simulink model "ATRIAS_vnmc"  (R2015a)
settings: Solver=ode45  StartTime=0.0  StopTime=60  FixedStep=1e-3  MinStep=1e-6  RelTol=1e-3  AbsTol=1e-4
values from neighbouring files (symbols this model uses):
  initial_boom_yaw = initial_boom_yaw + delta_yaw0    [run_model.m]
  max_floor_diff = cost_fun_opts.max_floor_diff    [opt_cmaes.m]    (also in run_model.m; set_all_params_simple.m = 0)
  noise_on_off = cost_fun_opts.noise_on_off    [opt_cmaes.m]    (also in run_model.m; set_all_params_simple.m = 0)
  noise_seed = cost_fun_opts.noise_seed    [opt_cmaes.m]    (also in run_model.m; set_all_params_simple.m = 1)
  noise_variance = cost_fun_opts.noise_variance    [opt_cmaes.m]    (also in run_model.m; set_all_params_simple.m = 0.000174532925199)
  SEA_swing_ctrl_on_off = cost_fun_opts.SEA_swing_ctrl_on_off    [opt_cmaes.m]    (also in run_model.m; set_all_params_simple.m = 0)
  sim_t = simout.twalk    [run_model.m]
  steady_dist = cost_fun_opts.steady_dist    [opt_cmaes.m]    (also in run_model.m; set_all_params_simple.m = 10)
  ts_anim = 0.0333    [run_model.m]
undefined symbols (not defined in the file or in its folder): A1_notch_f1, A2_notch_f1, A_lpf_dtau, A_lpf_velocity, B1_lpf_dtau, B1_lpf_velocity, B1_notch_f1, B2_lpf_dtau, B2_lpf_velocity, B2_notch_f1, b_hmotor, b_leg_spring, b_rotor, base_color_d, boom_color_d, boom_mount_to_center_diagonal, breakaway_friction, c, c_jointstop, com_height_offset, contactThr, coulomb_friction, CtrlPar_theta0, D12_S, D12_T, d_com, ddx_max, ddy_max, delta_phi_max, delta_phi_max_buffer, delta_phi_max_dropoff, delta_phi_min, des_forward_velocity, DS_width, dtau_des_max, dtheta0_vmc, dx0_vmc, dy_max, eref, fblink_color_d, fcut_acceleration, floor_color_d, floor_tile_width, floor_zero_height, FmaxBFSH, FmaxGLU, FmaxHAM, FmaxHFL, FmaxRF, FmaxVAS, FPCtrlPar, friction_linear_zone, g, gain_nodes_sea_torque, gamma_stance_thr, gamma_swing_thr, hip_height, HIP_MTR_MAX_CONT_TORQUE, HIP_MTR_MAX_TORQUE, hshaft_color_d ... (+236)
libraries: sm_lib x280, nesl_utility x174, simulink x114, simulink_extras x58, fl_lib x16, mblibv1 x2, dspswit3 x2
(part 21 of 23)

== matlab function ATRIAS_vnmc/control/Virtual Model Control/KKT_DS ==
  settings: updateMethod=DISCRETE  sampleTime=sample_time
  data: motor_trq output size=[4,1]; leg_force_hip_torque output size=[4,1]; grf output size=[4,1]; ddx_des input size=1; ddy_des input size=1; ddtheta_des input size=1; R_leg_length input size=1; L_leg_length input size=1; min_Fy input; R_gamma input size=1; L_gamma input size=1; R_splay input size=1; L_splay input size=1; theta input size=1; lambda1 input size=1; lambda2 input size=1; lambda3 input size=1; lambda4 input; mu_s input; sea_trqs input; cost_tie_break output size=1; err output size=[1,3]; grf_prev input
function [motor_trq,leg_force_hip_torque,grf,cost_tie_break,err]  = ...
         vmc(ddx_des,ddy_des,ddtheta_des,R_leg_length,L_leg_length,...
                min_Fy,R_gamma,L_gamma,R_splay,L_splay,theta,...
                lambda1,lambda2,lambda3,lambda4,mu_s,sea_trqs,grf_prev)

L1 = R_leg_length;
L2 = L_leg_length;
gamma1 = R_gamma;
gamma2 = L_gamma;
m = 64;
I = 4;
d = 0.1;
l_seg = 0.5;
g = 9.81;
% mu_s = 0.25;

% leg_force_hip_torque = J1*grf;
% motor_trq = J2*leg_force_hip_torque;
% motor_trq = J2*J1*grf;
% grf = J1_inv * J2_inv * motor_trq

J1 = [-sin(gamma1) -cos(gamma1) 0 0;
      -L1*cos(gamma1) L1*sin(gamma1) 0 0;
      0 0 -sin(gamma2) -cos(gamma2);
      0 0 -L2*cos(gamma2) L2*sin(gamma2)];
  
J2 = [-l_seg*sin(R_splay/2) 0.5 0 0;
       l_seg*sin(R_splay/2) 0.5 0 0;
       0 0 -l_seg*sin(L_splay/2) 0.5;
       0 0 l_seg*sin(R_splay/2) 0.5];
   
grf_meas = J1\J2\sea_trqs;


f1 = real([(I*ddtheta_des - L2*ddx_des*m*cos(gamma2) + L1*ddy_des*m*sin(gamma1) + L1*g*m*sin(gamma1) + d*ddx_des*m*cos(theta) - d*ddy_des*m*sin(theta) - d*g*m*sin(theta))/(L1*cos(gamma1) - L2*cos(gamma2));                                                                                                                                                                                                                                                                                                                                                                                                                                                                                                                                                                                                                                                                                                                                                                                                                                                                                                                                                                                                                                                                                                                                                                                                                                                                                                                                                                                                                                                                                                                                                                                                                                                                                                                                                                                                                                                                                                                                                                                                                                                                                                                                                                                                                                                                                                                                                                                                                                                                                                                                                                                                                                                                                                                                                                                                                                                                                                                                                                                                                                                                                                                                                                                                                                                                                                                                                                                                                                                                                                                                                                                                                                                                                                                                                                                                                                                                                                                                                                                                                                                                                                                                                                                                                                                                                                                                                                                                                                                                                                                                                                                                                                                                                                                                                                                                                                                                                                                                                                                                                                                                                                                                                                                                                                                                                                                                                                                                                                        
    (I*ddtheta_des - L2*ddx_des*m*cos(gamma2) + L2*ddy_des*m*sin(gamma2) + L2*g*m*sin(gamma2) + d*ddx_des*m*cos(theta) - d*ddy_des*m*sin(theta) - d*g*m*sin(theta))/(L1*cos(gamma1) - L2*cos(gamma2));
    (I^2*ddx_des*lambda1*lambda2*m + L1^2*ddx_des*lambda1*lambda3*m^3*sin(gamma1)^2 + d^2*ddx_des*lambda1*lambda3*m^3*sin(theta)^2 + L1^2*ddy_des*lambda2*lambda3*m^3*cos(gamma1)*sin(gamma1) + L1^2*g*lambda2*lambda3*m^3*cos(gamma1)*sin(gamma1) + I*L1*ddtheta_des*lambda2*lambda3*m^2*cos(gamma1) + d^2*ddy_des*lambda2*lambda3*m^3*cos(theta)*sin(theta) - I*d*ddtheta_des*lambda2*lambda3*m^2*cos(theta) + d^2*g*lambda2*lambda3*m^3*cos(theta)*sin(theta) - L1*d*ddy_des*lambda2*lambda3*m^3*cos(gamma1)*sin(theta) - L1*d*ddy_des*lambda2*lambda3*m^3*cos(theta)*sin(gamma1) - L1*d*g*lambda2*lambda3*m^3*cos(gamma1)*sin(theta) - L1*d*g*lambda2*lambda3*m^3*cos(theta)*sin(gamma1) - 2*L1*d*ddx_des*lambda1*lambda3*m^3*sin(gamma1)*sin(theta))/(I^2*lambda1*lambda2 + d^2*lambda1*lambda3*m^2*sin(theta)^2 + L1^2*lambda2*lambda3*m^2*cos(gamma1)^2 + L1^2*lambda1*lambda3*m^2*sin(gamma1)^2 + d^2*lambda2*lambda3*m^2*cos(theta)^2 - 2*L1*d*lambda2*lambda3*m^2*cos(gamma1)*cos(theta) - 2*L1*d*lambda1*lambda3*m^2*sin(gamma1)*sin(theta));
    0;
    0;
    0;
    0;
    0;
    (I*ddtheta_des - L2*ddx_des*m*cos(gamma2) + L1*ddy_des*m*sin(gamma1) + L1*g*m*sin(gamma1) + d*ddx_des*m*cos(theta) - d*ddy_des*m*sin(theta) - d*g*m*sin(theta))/(L1*cos(gamma1) - L2*cos(gamma2));
    0;
    (I^2*ddx_des*lambda1*lambda2*m + L1^2*ddx_des*lambda1*lambda3*m^3*sin(gamma1)^2 + d^2*ddx_des*lambda1*lambda3*m^3*sin(theta)^2 + L1^2*ddy_des*lambda2*lambda3*m^3*cos(gamma1)*sin(gamma1) + L1^2*g*lambda2*lambda3*m^3*cos(gamma1)*sin(gamma1) + I*L1*ddtheta_des*lambda2*lambda3*m^2*cos(gamma1) + d^2*ddy_des*lambda2*lambda3*m^3*cos(theta)*sin(theta) - I*d*ddtheta_des*lambda2*lambda3*m^2*cos(theta) + d^2*g*lambda2*lambda3*m^3*cos(theta)*sin(theta) - L1*d*ddy_des*lambda2*lambda3*m^3*cos(gamma1)*sin(theta) - L1*d*ddy_des*lambda2*lambda3*m^3*cos(theta)*sin(gamma1) - L1*d*g*lambda2*lambda3*m^3*cos(gamma1)*sin(theta) - L1*d*g*lambda2*lambda3*m^3*cos(theta)*sin(gamma1) - 2*L1*d*ddx_des*lambda1*lambda3*m^3*sin(gamma1)*sin(theta))/(I^2*lambda1*lambda2 + d^2*lambda1*lambda3*m^2*sin(theta)^2 + L1^2*lambda2*lambda3*m^2*cos(gamma1)^2 + L1^2*lambda1*lambda3*m^2*sin(gamma1)^2 + d^2*lambda2*lambda3*m^2*cos(theta)^2 - 2*L1*d*lambda2*lambda3*m^2*cos(gamma1)*cos(theta) - 2*L1*d*lambda1*lambda3*m^2*sin(gamma1)*sin(theta));
    0;
    0;
    0;
    0;
    0;
    (I*ddtheta_des*mu_s + L1*ddx_des*m*sin(gamma1) - L2*ddx_des*m*sin(gamma2) - L2*ddx_des*m*mu_s*cos(gamma2) + L1*ddy_des*m*mu_s*sin(gamma1) + L1*g*m*mu_s*sin(gamma1) + d*ddx_des*m*mu_s*cos(theta) - d*ddy_des*m*mu_s*sin(theta) - d*g*m*mu_s*sin(theta))/(L1*sin(gamma1) - L2*sin(gamma2) + L1*mu_s*cos(gamma1) - L2*mu_s*cos(gamma2));
    -(I*ddtheta_des*mu_s - L1*ddx_des*m*sin(gamma1) + L2*ddx_des*m*sin(gamma2) - L2*ddx_des*m*mu_s*cos(gamma2) + L1*ddy_des*m*mu_s*sin(gamma1) + L1*g*m*mu_s*sin(gamma1) + d*ddx_des*m*mu_s*cos(theta) - d*ddy_des*m*mu_s*sin(theta) - d*g*m*mu_s*sin(theta))/(L1*sin(gamma1) - L2*sin(gamma2) - L1*mu_s*cos(gamma1) + L2*mu_s*cos(gamma2));
    (mu_s*(I*ddtheta_des - L2*ddx_des*m*cos(gamma2) + L2*ddy_des*m*sin(gamma2) + L2*g*m*sin(gamma2) + d*ddx_des*m*cos(theta) - d*ddy_des*m*sin(theta) - d*g*m*sin(theta)))/(L1*sin(gamma1) - L2*sin(gamma2) + L1*mu_s*cos(gamma1) - L2*mu_s*cos(gamma2));
    -(mu_s*(I*ddtheta_des - L2*ddx_des*m*cos(gamma2) + L2*ddy_des*m*sin(gamma2) + L2*g*m*sin(gamma2) + d*ddx_des*m*cos(theta) - d*ddy_des*m*sin(theta) - d*g*m*sin(theta)))/(L1*sin(gamma1) - L2*sin(gamma2) - L1*mu_s*cos(gamma1) + L2*mu_s*cos(gamma2));
    (m*mu_s*(I^2*ddy_des*lambda1*lambda2 + I^2*g*lambda1*lambda2 + L2^2*ddy_des*lambda2*lambda3*m^2*cos(gamma2)^2 + L2^2*g*lambda2*lambda3*m^2*cos(gamma2)^2 + d^2*ddy_des*lambda2*lambda3*m^2*cos(theta)^2 + d^2*g*lambda2*lambda3*m^2*cos(theta)^2 - I*L1*ddtheta_des*lambda1*lambda3*m*sin(gamma1) + I*d*ddtheta_des*lambda1*lambda3*m*sin(theta) + L2^2*ddx_des*lambda1*lambda3*m^2*mu_s*cos(gamma2)^2 + d^2*ddx_des*lambda1*lambda3*m^2*cos(theta)*sin(theta) + L1*L2*ddx_des*lambda1*lambda3*m^2*cos(gamma2)*sin(gamma1) - 2*L2*d*ddy_des*lambda2*lambda3*m^2*cos(gamma2)*cos(theta) - 2*L2*d*g*lambda2*lambda3*m^2*cos(gamma2)*cos(theta) - L1*d*ddx_des*lambda1*lambda3*m^2*cos(theta)*sin(gamma1) - L2*d*ddx_des*lambda1*lambda3*m^2*cos(gamma2)*sin(theta) + I*L1*ddtheta_des*lambda1*lambda3*m*mu_s*cos(gamma1) - I*L2*ddtheta_des*lambda1*lambda3*m*mu_s*cos(gamma2) - L1*L2*ddx_des*lambda1*lambda3*m^2*mu_s*cos(gamma1)*cos(gamma2) + L1*d*ddx_des*lambda1*lambda3*m^2*mu_s*cos(gamma1)*cos(theta) - L2*d*ddx_des*lambda1*lambda3*m^2*mu_s*cos(gamma2)*cos(theta)))/(I^2*lambda1*lambda2 + d^2*lambda1*lambda3*m^2*sin(theta)^2 + L2^2*lambda2*lambda3*m^2*cos(gamma2)^2 + L1^2*lambda1*lambda3*m^2*sin(gamma1)^2 + d^2*lambda2*lambda3*m^2*cos(theta)^2 + L1^2*lambda1*lambda3*m^2*mu_s^2*cos(gamma1)^2 + L2^2*lambda1*lambda3*m^2*mu_s^2*cos(gamma2)^2 - 2*L2*d*lambda2*lambda3*m^2*cos(gamma2)*cos(theta) - 2*L1*d*lambda1*lambda3*m^2*sin(gamma1)*sin(theta) - 2*L1^2*lambda1*lambda3*m^2*mu_s*cos(gamma1)*sin(gamma1) + 2*L1*L2*lambda1*lambda3*m^2*mu_s*cos(gamma2)*sin(gamma1) + 2*L1*d*lambda1*lambda3*m^2*mu_s*cos(gamma1)*sin(theta) - 2*L2*d*lambda1*lambda3*m^2*mu_s*cos(gamma2)*sin(theta) - 2*L1*L2*lambda1*lambda3*m^2*mu_s^2*cos(gamma1)*cos(gamma2));
    0;
    (I*m*mu_s*(I*ddy_des*lambda2 + I*g*lambda2 + I*ddx_des*lambda1*mu_s - L1*ddtheta_des*lambda3*m*sin(gamma1) + d*ddtheta_des*lambda3*m*sin(theta) + L1*ddtheta_des*lambda3*m*mu_s*cos(gamma1) - d*ddtheta_des*lambda3*m*mu_s*cos(theta)))/(I^2*lambda2 + I^2*lambda1*mu_s^2 + L1^2*lambda3*m^2*sin(gamma1)^2 + d^2*lambda3*m^2*sin(theta)^2 + L1^2*lambda3*m^2*mu_s^2*cos(gamma1)^2 + d^2*lambda3*m^2*mu_s^2*cos(theta)^2 - 2*L1*d*lambda3*m^2*sin(gamma1)*sin(theta) - 2*L1^2*lambda3*m^2*mu_s*cos(gamma1)*sin(gamma1) - 2*d^2*lambda3*m^2*mu_s*cos(theta)*sin(theta) + 2*L1*d*lambda3*m^2*mu_s*cos(gamma1)*sin(theta) + 2*L1*d*lambda3*m^2*mu_s*cos(theta)*sin(gamma1) - 2*L1*d*lambda3*m^2*mu_s^2*cos(gamma1)*cos(theta));
    -(I*m*mu_s*(I*ddy_des*lambda2 + I*g*lambda2 - I*ddx_des*lambda1*mu_s - L1*ddtheta_des*lambda3*m*sin(gamma1) + d*ddtheta_des*lambda3*m*sin(theta) - L1*ddtheta_des*lambda3*m*mu_s*cos(gamma1) + d*ddtheta_des*lambda3*m*mu_s*cos(theta)))/(I^2*lambda2 + I^2*lambda1*mu_s^2 + L1^2*lambda3*m^2*sin(gamma1)^2 + d^2*lambda3*m^2*sin(theta)^2 + L1^2*lambda3*m^2*mu_s^2*cos(gamma1)^2 + d^2*lambda3*m^2*mu_s^2*cos(theta)^2 - 2*L1*d*lambda3*m^2*sin(gamma1)*sin(theta) + 2*L1^2*lambda3*m^2*mu_s*cos(gamma1)*sin(gamma1) + 2*d^2*lambda3*m^2*mu_s*cos(theta)*sin(theta) - 2*L1*d*lambda3*m^2*mu_s*cos(gamma1)*sin(theta) - 2*L1*d*lambda3*m^2*mu_s*cos(theta)*sin(gamma1) - 2*L1*d*lambda3*m^2*mu_s^2*cos(gamma1)*cos(theta));
    0;
    0;
    (I*(I*ddx_des*lambda1*m + L1*ddtheta_des*lambda3*m^2*cos(gamma1) - d*ddtheta_des*lambda3*m^2*cos(theta)))/(I^2*lambda1 + L1^2*lambda3*m^2*cos(gamma1)^2 + d^2*lambda3*m^2*cos(theta)^2 - 2*L1*d*lambda3*m^2*cos(gamma1)*cos(theta));
    (mu_s*(I*ddtheta_des*lambda2 + I*ddtheta_des*lambda1*mu_s^2 + L2*ddy_des*lambda2*m*sin(gamma2) + L2*g*lambda2*m*sin(gamma2) - d*ddy_des*lambda2*m*sin(theta) - d*g*lambda2*m*sin(theta) + L2*ddy_des*lambda2*m*mu_s*cos(gamma2) + L2*g*lambda2*m*mu_s*cos(gamma2) - L2*ddx_des*lambda1*m*mu_s*sin(gamma2) - d*ddy_des*lambda2*m*mu_s*cos(theta) - d*g*lambda2*m*mu_s*cos(theta) + d*ddx_des*lambda1*m*mu_s*sin(theta) - L2*ddx_des*lambda1*m*mu_s^2*cos(gamma2) + d*ddx_des*lambda1*m*mu_s^2*cos(theta)))/((lambda1*mu_s^2 + lambda2)*(L1*sin(gamma1) - L2*sin(gamma2) + L1*mu_s*cos(gamma1) - L2*mu_s*cos(gamma2)));
    -(mu_s*(I*ddtheta_des*lambda2 + I*ddtheta_des*lambda1*mu_s^2 + L2*ddy_des*lambda2*m*sin(gamma2) + L2*g*lambda2*m*sin(gamma2) - d*ddy_des*lambda2*m*sin(theta) - d*g*lambda2*m*sin(theta) - L2*ddy_des*lambda2*m*mu_s*cos(gamma2) - L2*g*lambda2*m*mu_s*cos(gamma2) + L2*ddx_des*lambda1*m*mu_s*sin(gamma2) + d*ddy_des*lambda2*m*mu_s*cos(theta) + d*g*lambda2*m*mu_s*cos(theta) - d*ddx_des*lambda1*m*mu_s*sin(theta) - L2*ddx_des*lambda1*m*mu_s^2*cos(gamma2) + d*ddx_des*lambda1*m*mu_s^2*cos(theta)))/((lambda1*mu_s^2 + lambda2)*(L1*sin(gamma1) - L2*sin(gamma2) - L1*mu_s*cos(gamma1) + L2*mu_s*cos(gamma2)));
    -(m*mu_s*(I^2*ddy_des*lambda1*lambda2 + I^2*g*lambda1*lambda2 + L2^2*ddy_des*lambda2*lambda3*m^2*cos(gamma2)^2 + L2^2*g*lambda2*lambda3*m^2*cos(gamma2)^2 + d^2*ddy_des*lambda2*lambda3*m^2*cos(theta)^2 + d^2*g*lambda2*lambda3*m^2*cos(theta)^2 - I*L1*ddtheta_des*lambda1*lambda3*m*sin(gamma1) + I*d*ddtheta_des*lambda1*lambda3*m*sin(theta) - L2^2*ddx_des*lambda1*lambda3*m^2*mu_s*cos(gamma2)^2 + d^2*ddx_des*lambda1*lambda3*m^2*cos(theta)*sin(theta) + L1*L2*ddx_des*lambda1*lambda3*m^2*cos(gamma2)*sin(gamma1) - 2*L2*d*ddy_des*lambda2*lambda3*m^2*cos(gamma2)*cos(theta) - 2*L2*d*g*lambda2*lambda3*m^2*cos(gamma2)*cos(theta) - L1*d*ddx_des*lambda1*lambda3*m^2*cos(theta)*sin(gamma1) - L2*d*ddx_des*lambda1*lambda3*m^2*cos(gamma2)*sin(theta) - I*L1*ddtheta_des*lambda1*lambda3*m*mu_s*cos(gamma1) + I*L2*ddtheta_des*lambda1*lambda3*m*mu_s*cos(gamma2) + L1*L2*ddx_des*lambda1*lambda3*m^2*mu_s*cos(gamma1)*cos(gamma2) - L1*d*ddx_des*lambda1*lambda3*m^2*mu_s*cos(gamma1)*cos(theta) + L2*d*ddx_des*lambda1*lambda3*m^2*mu_s*cos(gamma2)*cos(theta)))/(I^2*lambda1*lambda2 + d^2*lambda1*lambda3*m^2*sin(theta)^2 + L2^2*lambda2*lambda3*m^2*cos(gamma2)^2 + L1^2*lambda1*lambda3*m^2*sin(gamma1)^2 + d^2*lambda2*lambda3*m^2*cos(theta)^2 + L1^2*lambda1*lambda3*m^2*mu_s^2*cos(gamma1)^2 + L2^2*lambda1*lambda3*m^2*mu_s^2*cos(gamma2)^2 - 2*L2*d*lambda2*lambda3*m^2*cos(gamma2)*cos(theta) - 2*L1*d*lambda1*lambda3*m^2*sin(gamma1)*sin(theta) + 2*L1^2*lambda1*lambda3*m^2*mu_s*cos(gamma1)*sin(gamma1) - 2*L1*L2*lambda1*lambda3*m^2*mu_s*cos(gamma2)*sin(gamma1) - 2*L1*d*lambda1*lambda3*m^2*mu_s*cos(gamma1)*sin(theta) + 2*L2*d*lambda1*lambda3*m^2*mu_s*cos(gamma2)*sin(theta) - 2*L1*L2*lambda1*lambda3*m^2*mu_s^2*cos(gamma1)*cos(gamma2));
    (I^2*ddx_des*lambda1*lambda2*m - I^2*ddy_des*lambda1*lambda2*m*mu_s - I^2*g*lambda1*lambda2*m*mu_s + L2^2*ddx_des*lambda1*lambda3*m^3*sin(gamma2)^2 + d^2*ddx_des*lambda1*lambda3*m^3*sin(theta)^2 + L2^2*ddx_des*lambda1*lambda3*m^3*mu_s^2*cos(gamma2)^2 + I*L1*ddtheta_des*lambda2*lambda3*m^2*cos(gamma1) - d^2*ddy_des*lambda2*lambda3*m^3*mu_s*cos(theta)^2 - d^2*g*lambda2*lambda3*m^3*mu_s*cos(theta)^2 + d^2*ddy_des*lambda2*lambda3*m^3*cos(theta)*sin(theta) - I*d*ddtheta_des*lambda2*lambda3*m^2*cos(theta) + d^2*g*lambda2*lambda3*m^3*cos(theta)*sin(theta) - 2*L2^2*ddx_des*lambda1*lambda3*m^3*mu_s*cos(gamma2)*sin(gamma2) + I*L2*ddtheta_des*lambda1*lambda3*m^2*mu_s*sin(gamma2) - d^2*ddx_des*lambda1*lambda3*m^3*mu_s*cos(theta)*sin(theta) - I*d*ddtheta_des*lambda1*lambda3*m^2*mu_s*sin(theta) + I*L1*ddtheta_des*lambda1*lambda3*m^2*mu_s^2*cos(gamma1) - I*L2*ddtheta_des*lambda1*lambda3*m^2*mu_s^2*cos(gamma2) + L1*L2*ddy_des*lambda2*lambda3*m^3*cos(gamma1)*sin(gamma2) + L1*L2*g*lambda2*lambda3*m^3*cos(gamma1)*sin(gamma2) - L1*d*ddy_des*lambda2*lambda3*m^3*cos(gamma1)*sin(theta) - L2*d*ddy_des*lambda2*lambda3*m^3*cos(theta)*sin(gamma2) - L1*d*g*lambda2*lambda3*m^3*cos(gamma1)*sin(theta) - L2*d*g*lambda2*lambda3*m^3*cos(theta)*sin(gamma2) - 2*L2*d*ddx_des*lambda1*lambda3*m^3*sin(gamma2)*sin(theta) - L1*L2*ddy_des*lambda2*lambda3*m^3*mu_s*cos(gamma1)*cos(gamma2) - L1*L2*g*lambda2*lambda3*m^3*mu_s*cos(gamma1)*cos(gamma2) + L1*L2*ddx_des*lambda1*lambda3*m^3*mu_s*cos(gamma1)*sin(gamma2) + L1*d*ddy_des*lambda2*lambda3*m^3*mu_s*cos(gamma1)*cos(theta) + L2*d*ddy_des*lambda2*lambda3*m^3*mu_s*cos(gamma2)*cos(theta) + L1*d*g*lambda2*lambda3*m^3*mu_s*cos(gamma1)*cos(theta) + L2*d*g*lambda2*lambda3*m^3*mu_s*cos(gamma2)*cos(theta) - L1*d*ddx_des*lambda1*lambda3*m^3*mu_s*cos(gamma1)*sin(theta) + 2*L2*d*ddx_des*lambda1*lambda3*m^3*mu_s*cos(gamma2)*sin(theta) + L2*d*ddx_des*lambda1*lambda3*m^3*mu_s*cos(theta)*sin(gamma2) - L1*L2*ddx_des*lambda1*lambda3*m^3*mu_s^2*cos(gamma1)*cos(gamma2) + L1*d*ddx_des*lambda1*lambda3*m^3*mu_s^2*cos(gamma1)*cos(theta) - L2*d*ddx_des*lambda1*lambda3*m^3*mu_s^2*cos(gamma2)*cos(theta))/(I^2*lambda1*lambda2 + d^2*lambda1*lambda3*m^2*sin(theta)^2 + L1^2*lambda2*lambda3*m^2*cos(gamma1)^2 + L2^2*lambda1*lambda3*m^2*sin(gamma2)^2 + d^2*lambda2*lambda3*m^2*cos(theta)^2 + L1^2*lambda1*lambda3*m^2*mu_s^2*cos(gamma1)^2 + L2^2*lambda1*lambda3*m^2*mu_s^2*cos(gamma2)^2 - 2*L1*d*lambda2*lambda3*m^2*cos(gamma1)*cos(theta) - 2*L2*d*lambda1*lambda3*m^2*sin(gamma2)*sin(theta) - 2*L2^2*lambda1*lambda3*m^2*mu_s*cos(gamma2)*sin(gamma2) + 2*L1*L2*lambda1*lambda3*m^2*mu_s*cos(gamma1)*sin(gamma2) - 2*L1*d*lambda1*lambda3*m^2*mu_s*cos(gamma1)*sin(theta) + 2*L2*d*lambda1*lambda3*m^2*mu_s*cos(gamma2)*sin(theta) - 2*L1*L2*lambda1*lambda3*m^2*mu_s^2*cos(gamma1)*cos(gamma2));
    (I^2*ddx_des*lambda1*lambda2*m + I^2*ddy_des*lambda1*lambda2*m*mu_s + I^2*g*lambda1*lambda2*m*mu_s + L2^2*ddx_des*lambda1*lambda3*m^3*sin(gamma2)^2 + d^2*ddx_des*lambda1*lambda3*m^3*sin(theta)^2 + L2^2*ddx_des*lambda1*lambda3*m^3*mu_s^2*cos(gamma2)^2 + I*L1*ddtheta_des*lambda2*lambda3*m^2*cos(gamma1) + d^2*ddy_des*lambda2*lambda3*m^3*mu_s*cos(theta)^2 + d^2*g*lambda2*lambda3*m^3*mu_s*cos(theta)^2 + d^2*ddy_des*lambda2*lambda3*m^3*cos(theta)*sin(theta) - I*d*ddtheta_des*lambda2*lambda3*m^2*cos(theta) + d^2*g*lambda2*lambda3*m^3*cos(theta)*sin(theta) + 2*L2^2*ddx_des*lambda1*lambda3*m^3*mu_s*cos(gamma2)*sin(gamma2) - I*L2*ddtheta_des*lambda1*lambda3*m^2*mu_s*sin(gamma2) + d^2*ddx_des*lambda1*lambda3*m^3*mu_s*cos(theta)*sin(theta) + I*d*ddtheta_des*lambda1*lambda3*m^2*mu_s*sin(theta) + I*L1*ddtheta_des*lambda1*lambda3*m^2*mu_s^2*cos(gamma1) - I*L2*ddtheta_des*lambda1*lambda3*m^2*mu_s^2*cos(gamma2) + L1*L2*ddy_des*lambda2*lambda3*m^3*cos(gamma1)*sin(gamma2) + L1*L2*g*lambda2*lambda3*m^3*cos(gamma1)*sin(gamma2) - L1*d*ddy_des*lambda2*lambda3*m^3*cos(gamma1)*sin(theta) - L2*d*ddy_des*lambda2*lambda3*m^3*cos(theta)*sin(gamma2) - L1*d*g*lambda2*lambda3*m^3*cos(gamma1)*sin(theta) - L2*d*g*lambda2*lambda3*m^3*cos(theta)*sin(gamma2) - 2*L2*d*ddx_des*lambda1*lambda3*m^3*sin(gamma2)*sin(theta) + L1*L2*ddy_des*lambda2*lambda3*m^3*mu_s*cos(gamma1)*cos(gamma2) + L1*L2*g*lambda2*lambda3*m^3*mu_s*cos(gamma1)*cos(gamma2) - L1*L2*ddx_des*lambda1*lambda3*m^3*mu_s*cos(gamma1)*sin(gamma2) - L1*d*ddy_des*lambda2*lambda3*m^3*mu_s*cos(gamma1)*cos(theta) - L2*d*ddy_des*lambda2*lambda3*m^3*mu_s*cos(gamma2)*cos(theta) - L1*d*g*lambda2*lambda3*m^3*mu_s*cos(gamma1)*cos(theta) - L2*d*g*lambda2*lambda3*m^3*mu_s*cos(gamma2)*cos(theta) + L1*d*ddx_des*lambda1*lambda3*m^3*mu_s*cos(gamma1)*sin(theta) - 2*L2*d*ddx_des*lambda1*lambda3*m^3*mu_s*cos(gamma2)*sin(theta) - L2*d*ddx_des*lambda1*lambda3*m^3*mu_s*cos(theta)*sin(gamma2) - L1*L2*ddx_des*lambda1*lambda3*m^3*mu_s^2*cos(gamma1)*cos(gamma2) + L1*d*ddx_des*lambda1*lambda3*m^3*mu_s^2*cos(gamma1)*cos(theta) - L2*d*ddx_des*lambda1*lambda3*m^3*mu_s^2*cos(gamma2)*cos(theta))/(I^2*lambda1*lambda2 + d^2*lambda1*lambda3*m^2*sin(theta)^2 + L1^2*lambda2*lambda3*m^2*cos(gamma1)^2 + L2^2*lambda1*lambda3*m^2*sin(gamma2)^2 + d^2*lambda2*lambda3*m^2*cos(theta)^2 + L1^2*lambda1*lambda3*m^2*mu_s^2*cos(gamma1)^2 + L2^2*lambda1*lambda3*m^2*mu_s^2*cos(gamma2)^2 - 2*L1*d*lambda2*lambda3*m^2*cos(gamma1)*cos(theta) - 2*L2*d*lambda1*lambda3*m^2*sin(gamma2)*sin(theta) + 2*L2^2*lambda1*lambda3*m^2*mu_s*cos(gamma2)*sin(gamma2) - 2*L1*L2*lambda1*lambda3*m^2*mu_s*cos(gamma1)*sin(gamma2) + 2*L1*d*lambda1*lambda3*m^2*mu_s*cos(gamma1)*sin(theta) - 2*L2*d*lambda1*lambda3*m^2*mu_s*cos(gamma2)*sin(theta) - 2*L1*L2*lambda1*lambda3*m^2*mu_s^2*cos(gamma1)*cos(gamma2));
    (I*(I*ddx_des*lambda1*m + L1*ddtheta_des*lambda3*m^2*cos(gamma1) - d*ddtheta_des*lambda3*m^2*cos(theta)))/(I^2*lambda1 + L1^2*lambda3*m^2*cos(gamma1)^2 + d^2*lambda3*m^2*cos(theta)^2 - 2*L1*d*lambda3*m^2*cos(gamma1)*cos(theta));
    (I^2*ddx_des*lambda1*lambda2*m + L1^2*ddx_des*lambda1*lambda3*m^3*sin(gamma1)^2 + d^2*ddx_des*lambda1*lambda3*m^3*sin(theta)^2 + L1^2*ddy_des*lambda2*lambda3*m^3*cos(gamma1)*sin(gamma1) + L1^2*g*lambda2*lambda3*m^3*cos(gamma1)*sin(gamma1) + I*L1*ddtheta_des*lambda2*lambda3*m^2*cos(gamma1) + d^2*ddy_des*lambda2*lambda3*m^3*cos(theta)*sin(theta) - I*d*ddtheta_des*lambda2*lambda3*m^2*cos(theta) + d^2*g*lambda2*lambda3*m^3*cos(theta)*sin(theta) - L1*d*ddy_des*lambda2*lambda3*m^3*cos(gamma1)*sin(theta) - L1*d*ddy_des*lambda2*lambda3*m^3*cos(theta)*sin(gamma1) - L1*d*g*lambda2*lambda3*m^3*cos(gamma1)*sin(theta) - L1*d*g*lambda2*lambda3*m^3*cos(theta)*sin(gamma1) - 2*L1*d*ddx_des*lambda1*lambda3*m^3*sin(gamma1)*sin(theta))/(I^2*lambda1*lambda2 + d^2*lambda1*lambda3*m^2*sin(theta)^2 + L1^2*lambda2*lambda3*m^2*cos(gamma1)^2 + L1^2*lambda1*lambda3*m^2*sin(gamma1)^2 + d^2*lambda2*lambda3*m^2*cos(theta)^2 - 2*L1*d*lambda2*lambda3*m^2*cos(gamma1)*cos(theta) - 2*L1*d*lambda1*lambda3*m^2*sin(gamma1)*sin(theta));
    (I^2*ddx_des*lambda1*lambda2*m + L1^2*ddx_des*lambda1*lambda3*m^3*sin(gamma1)^2 + d^2*ddx_des*lambda1*lambda3*m^3*sin(theta)^2 + L1^2*ddy_des*lambda2*lambda3*m^3*cos(gamma1)*sin(gamma1) + L1^2*g*lambda2*lambda3*m^3*cos(gamma1)*sin(gamma1) + I*L1*ddtheta_des*lambda2*lambda3*m^2*cos(gamma1) + d^2*ddy_des*lambda2*lambda3*m^3*cos(theta)*sin(theta) - I*d*ddtheta_des*lambda2*lambda3*m^2*cos(theta) + d^2*g*lambda2*lambda3*m^3*cos(theta)*sin(theta) - L1*d*ddy_des*lambda2*lambda3*m^3*cos(gamma1)*sin(theta) - L1*d*ddy_des*lambda2*lambda3*m^3*cos(theta)*sin(gamma1) - L1*d*g*lambda2*lambda3*m^3*cos(gamma1)*sin(theta) - L1*d*g*lambda2*lambda3*m^3*cos(theta)*sin(gamma1) - 2*L1*d*ddx_des*lambda1*lambda3*m^3*sin(gamma1)*sin(theta))/(I^2*lambda1*lambda2 + d^2*lambda1*lambda3*m^2*sin(theta)^2 + L1^2*lambda2*lambda3*m^2*cos(gamma1)^2 + L1^2*lambda1*lambda3*m^2*sin(gamma1)^2 + d^2*lambda2*lambda3*m^2*cos(theta)^2 - 2*L1*d*lambda2*lambda3*m^2*cos(gamma1)*cos(theta) - 2*L1*d*lambda1*lambda3*m^2*sin(gamma1)*sin(theta));
    0;
    0;
    (I*ddtheta_des - L2*ddx_des*m*cos(gamma2) + d*ddx_des*m*cos(theta))/(L1*cos(gamma1) - L2*cos(gamma2));
    (I*(I*ddx_des*lambda1*m + L1*ddtheta_des*lambda3*m^2*cos(gamma1) - d*ddtheta_des*lambda3*m^2*cos(theta)))/(I^2*lambda1 + L1^2*lambda3*m^2*cos(gamma1)^2 + d^2*lambda3*m^2*cos(theta)^2 - 2*L1*d*lambda3*m^2*cos(gamma1)*cos(theta));
    (I*(I*ddx_des*lambda1*m + L1*ddtheta_des*lambda3*m^2*cos(gamma1) - d*ddtheta_des*lambda3*m^2*cos(theta)))/(I^2*lambda1 + L1^2*lambda3*m^2*cos(gamma1)^2 + d^2*lambda3*m^2*cos(theta)^2 - 2*L1*d*lambda3*m^2*cos(gamma1)*cos(theta));
    0;
    0;
    0;
    0;
    0;
    0;
    0;
    0;
    (I*m*mu_s*(I*ddy_des*lambda2 + I*g*lambda2 + I*ddx_des*lambda1*mu_s - L1*ddtheta_des*lambda3*m*sin(gamma1) + d*ddtheta_des*lambda3*m*sin(theta) + L1*ddtheta_des*lambda3*m*mu_s*cos(gamma1) - d*ddtheta_des*lambda3*m*mu_s*cos(theta)))/(I^2*lambda2 + I^2*lambda1*mu_s^2 + L1^2*lambda3*m^2*sin(gamma1)^2 + d^2*lambda3*m^2*sin(theta)^2 + L1^2*lambda3*m^2*mu_s^2*cos(gamma1)^2 + d^2*lambda3*m^2*mu_s^2*cos(theta)^2 - 2*L1*d*lambda3*m^2*sin(gamma1)*sin(theta) - 2*L1^2*lambda3*m^2*mu_s*cos(gamma1)*sin(gamma1) - 2*d^2*lambda3*m^2*mu_s*cos(theta)*sin(theta) + 2*L1*d*lambda3*m^2*mu_s*cos(gamma1)*sin(theta) + 2*L1*d*lambda3*m^2*mu_s*cos(theta)*sin(gamma1) - 2*L1*d*lambda3*m^2*mu_s^2*cos(gamma1)*cos(theta));
    -(I*m*mu_s*(I*ddy_des*lambda2 + I*g*lambda2 - I*ddx_des*lambda1*mu_s - L1*ddtheta_des*lambda3*m*sin(gamma1) + d*ddtheta_des*lambda3*m*sin(theta) - L1*ddtheta_des*lambda3*m*mu_s*cos(gamma1) + d*ddtheta_des*lambda3*m*mu_s*cos(theta)))/(I^2*lambda2 + I^2*lambda1*mu_s^2 + L1^2*lambda3*m^2*sin(gamma1)^2 + d^2*lambda3*m^2*sin(theta)^2 + L1^2*lambda3*m^2*mu_s^2*cos(gamma1)^2 + d^2*lambda3*m^2*mu_s^2*cos(theta)^2 - 2*L1*d*lambda3*m^2*sin(gamma1)*sin(theta) + 2*L1^2*lambda3*m^2*mu_s*cos(gamma1)*sin(gamma1) + 2*d^2*lambda3*m^2*mu_s*cos(theta)*sin(theta) - 2*L1*d*lambda3*m^2*mu_s*cos(gamma1)*sin(theta) - 2*L1*d*lambda3*m^2*mu_s*cos(theta)*sin(gamma1) - 2*L1*d*lambda3*m^2*mu_s^2*cos(gamma1)*cos(theta));
    0;
    0;
    0;
    0;
    -(I*m*mu_s*(I*ddy_des*lambda2 + I*g*lambda2 - I*ddx_des*lambda1*mu_s - L1*ddtheta_des*lambda3*m*sin(gamma1) + d*ddtheta_des*lambda3*m*sin(theta) - L1*ddtheta_des*lambda3*m*mu_s*cos(gamma1) + d*ddtheta_des*lambda3*m*mu_s*cos(theta)))/(I^2*lambda2 + I^2*lambda1*mu_s^2 + L1^2*lambda3*m^2*sin(gamma1)^2 + d^2*lambda3*m^2*sin(theta)^2 + L1^2*lambda3*m^2*mu_s^2*cos(gamma1)^2 + d^2*lambda3*m^2*mu_s^2*cos(theta)^2 - 2*L1*d*lambda3*m^2*sin(gamma1)*sin(theta) + 2*L1^2*lambda3*m^2*mu_s*cos(gamma1)*sin(gamma1) + 2*d^2*lambda3*m^2*mu_s*cos(theta)*sin(theta) - 2*L1*d*lambda3*m^2*mu_s*cos(gamma1)*sin(theta) - 2*L1*d*lambda3*m^2*mu_s*cos(theta)*sin(gamma1) - 2*L1*d*lambda3*m^2*mu_s^2*cos(gamma1)*cos(theta));
    (I*m*mu_s*(I*ddy_des*lambda2 + I*g*lambda2 + I*ddx_des*lambda1*mu_s - L1*ddtheta_des*lambda3*m*sin(gamma1) + d*ddtheta_des*lambda3*m*sin(theta) + L1*ddtheta_des*lambda3*m*mu_s*cos(gamma1) - d*ddtheta_des*lambda3*m*mu_s*cos(theta)))/(I^2*lambda2 + I^2*lambda1*mu_s^2 + L1^2*lambda3*m^2*sin(gamma1)^2 + d^2*lambda3*m^2*sin(theta)^2 + L1^2*lambda3*m^2*mu_s^2*cos(gamma1)^2 + d^2*lambda3*m^2*mu_s^2*cos(theta)^2 - 2*L1*d*lambda3*m^2*sin(gamma1)*sin(theta) - 2*L1^2*lambda3*m^2*mu_s*cos(gamma1)*sin(gamma1) - 2*d^2*lambda3*m^2*mu_s*cos(theta)*sin(theta) + 2*L1*d*lambda3*m^2*mu_s*cos(gamma1)*sin(theta) + 2*L1*d*lambda3*m^2*mu_s*cos(theta)*sin(gamma1) - 2*L1*d*lambda3*m^2*mu_s^2*cos(gamma1)*cos(theta));
    0;
    0;
    (I*m*mu_s*(I*ddy_des*lambda2 + I*g*lambda2 + I*ddx_des*lambda1*mu_s - L1*ddtheta_des*lambda3*m*sin(gamma1) + d*ddtheta_des*lambda3*m*sin(theta) + L1*ddtheta_des*lambda3*m*mu_s*cos(gamma1) - d*ddtheta_des*lambda3*m*mu_s*cos(theta)))/(I^2*lambda2 + I^2*lambda1*mu_s^2 + L1^2*lambda3*m^2*sin(gamma1)^2 + d^2*lambda3*m^2*sin(theta)^2 + L1^2*lambda3*m^2*mu_s^2*cos(gamma1)^2 + d^2*lambda3*m^2*mu_s^2*cos(theta)^2 - 2*L1*d*lambda3*m^2*sin(gamma1)*sin(theta) - 2*L1^2*lambda3*m^2*mu_s*cos(gamma1)*sin(gamma1) - 2*d^2*lambda3*m^2*mu_s*cos(theta)*sin(theta) + 2*L1*d*lambda3*m^2*mu_s*cos(gamma1)*sin(theta) + 2*L1*d*lambda3*m^2*mu_s*cos(theta)*sin(gamma1) - 2*L1*d*lambda3*m^2*mu_s^2*cos(gamma1)*cos(theta));
    -(I*m*mu_s*(I*ddy_des*lambda2 + I*g*lambda2 - I*ddx_des*lambda1*mu_s - L1*ddtheta_des*lambda3*m*sin(gamma1) + d*ddtheta_des*lambda3*m*sin(theta) - L1*ddtheta_des*lambda3*m*mu_s*cos(gamma1) + d*ddtheta_des*lambda3*m*mu_s*cos(theta)))/(I^2*lambda2 + I^2*lambda1*mu_s^2 + L1^2*lambda3*m^2*sin(gamma1)^2 + d^2*lambda3*m^2*sin(theta)^2 + L1^2*lambda3*m^2*mu_s^2*cos(gamma1)^2 + d^2*lambda3*m^2*mu_s^2*cos(theta)^2 - 2*L1*d*lambda3*m^2*sin(gamma1)*sin(theta) + 2*L1^2*lambda3*m^2*mu_s*cos(gamma1)*sin(gamma1) + 2*d^2*lambda3*m^2*mu_s*cos(theta)*sin(theta) - 2*L1*d*lambda3*m^2*mu_s*cos(gamma1)*sin(theta) - 2*L1*d*lambda3*m^2*mu_s*cos(theta)*sin(gamma1) - 2*L1*d*lambda3*m^2*mu_s^2*cos(gamma1)*cos(theta));
    0;
    0;
    -(m*mu_s*(2*I^2*ddy_des*lambda1*lambda2*mu_s^2 + 2*I^2*g*lambda1*lambda2*mu_s^2 - 2*I^2*ddx_des*lambda1*lambda2*mu_s + L2^2*ddy_des*lambda2*lambda3*m^2*sin(gamma2)^2 + L2^2*g*lambda2*lambda3*m^2*sin(gamma2)^2 - L2^2*ddx_des*lambda1*lambda3*m^2*mu_s^3*cos(gamma2)^2 + L2^2*ddy_des*lambda2*lambda3*m^2*mu_s^2*cos(gamma2)^2 + L2^2*g*lambda2*lambda3*m^2*mu_s^2*cos(gamma2)^2 + 2*d^2*ddy_des*lambda2*lambda3*m^2*mu_s^2*cos(theta)^2 + 2*d^2*g*lambda2*lambda3*m^2*mu_s^2*cos(theta)^2 - I*L1*ddtheta_des*lambda2*lambda3*m*sin(gamma1) + I*L2*ddtheta_des*lambda2*lambda3*m*sin(gamma2) - L2^2*ddx_des*lambda1*lambda3*m^2*mu_s*sin(gamma2)^2 - 2*d^2*ddx_des*lambda1*lambda3*m^2*mu_s*sin(theta)^2 - 2*L2^2*ddy_des*lambda2*lambda3*m^2*mu_s*cos(gamma2)*sin(gamma2) - 2*L2^2*g*lambda2*lambda3*m^2*mu_s*cos(gamma2)*sin(gamma2) - I*L1*ddtheta_des*lambda1*lambda3*m*mu_s^3*cos(gamma1) + I*L2*ddtheta_des*lambda1*lambda3*m*mu_s^3*cos(gamma2) - I*L1*ddtheta_des*lambda1*lambda3*m*mu_s^2*sin(gamma1) - I*L2*ddtheta_des*lambda1*lambda3*m*mu_s^2*sin(gamma2) - 2*d^2*ddy_des*lambda2*lambda3*m^2*mu_s*cos(theta)*sin(theta) - 2*d^2*g*lambda2*lambda3*m^2*mu_s*cos(theta)*sin(theta) + 2*I*d*ddtheta_des*lambda1*lambda3*m*mu_s^2*sin(theta) + 2*L2^2*ddx_des*lambda1*lambda3*m^2*mu_s^2*cos(gamma2)*sin(gamma2) - L1*L2*ddy_des*lambda2*lambda3*m^2*sin(gamma1)*sin(gamma2) + 2*d^2*ddx_des*lambda1*lambda3*m^2*mu_s^2*cos(theta)*sin(theta) - L1*L2*g*lambda2*lambda3*m^2*sin(gamma1)*sin(gamma2) - I*L1*ddtheta_des*lambda2*lambda3*m*mu_s*cos(gamma1) - I*L2*ddtheta_des*lambda2*lambda3*m*mu_s*cos(gamma2) + L1*d*ddy_des*lambda2*lambda3*m^2*sin(gamma1)*sin(theta) - L2*d*ddy_des*lambda2*lambda3*m^2*sin(gamma2)*sin(theta) + L1*d*g*lambda2*lambda3*m^2*sin(gamma1)*sin(theta) - L2*d*g*lambda2*lambda3*m^2*sin(gamma2)*sin(theta) + 2*I*d*ddtheta_des*lambda2*lambda3*m*mu_s*cos(theta) - L1*L2*ddy_des*lambda2*lambda3*m^2*mu_s*cos(gamma1)*sin(gamma2) + L1*L2*ddy_des*lambda2*lambda3*m^2*mu_s*cos(gamma2)*sin(gamma1) - L1*L2*g*lambda2*lambda3*m^2*mu_s*cos(gamma1)*sin(gamma2) + L1*L2*g*lambda2*lambda3*m^2*mu_s*cos(gamma2)*sin(gamma1) - L1*L2*ddx_des*lambda1*lambda3*m^2*mu_s*sin(gamma1)*sin(gamma2) + L1*d*ddy_des*lambda2*lambda3*m^2*mu_s*cos(gamma1)*sin(theta) - L1*d*ddy_des*lambda2*lambda3*m^2*mu_s*cos(theta)*sin(gamma1) + L2*d*ddy_des*lambda2*lambda3*m^2*mu_s*cos(gamma2)*sin(theta) + 3*L2*d*ddy_des*lambda2*lambda3*m^2*mu_s*cos(theta)*sin(gamma2) + L1*d*g*lambda2*lambda3*m^2*mu_s*cos(gamma1)*sin(theta) - L1*d*g*lambda2*lambda3*m^2*mu_s*cos(theta)*sin(gamma1) + L2*d*g*lambda2*lambda3*m^2*mu_s*cos(gamma2)*sin(theta) + 3*L2*d*g*lambda2*lambda3*m^2*mu_s*cos(theta)*sin(gamma2) + L1*d*ddx_des*lambda1*lambda3*m^2*mu_s*sin(gamma1)*sin(theta) + 3*L2*d*ddx_des*lambda1*lambda3*m^2*mu_s*sin(gamma2)*sin(theta) + L1*L2*ddx_des*lambda1*lambda3*m^2*mu_s^3*cos(gamma1)*cos(gamma2) + L1*L2*ddy_des*lambda2*lambda3*m^2*mu_s^2*cos(gamma1)*cos(gamma2) + L1*L2*g*lambda2*lambda3*m^2*mu_s^2*cos(gamma1)*cos(gamma2) - L1*L2*ddx_des*lambda1*lambda3*m^2*mu_s^2*cos(gamma1)*sin(gamma2) + L1*L2*ddx_des*lambda1*lambda3*m^2*mu_s^2*cos(gamma2)*sin(gamma1) - L1*d*ddx_des*lambda1*lambda3*m^2*mu_s^3*cos(gamma1)*cos(theta) + L2*d*ddx_des*lambda1*lambda3*m^2*mu_s^3*cos(gamma2)*cos(theta) - L1*d*ddy_des*lambda2*lambda3*m^2*mu_s^2*cos(gamma1)*cos(theta) - 3*L2*d*ddy_des*lambda2*lambda3*m^2*mu_s^2*cos(gamma2)*cos(theta) - L1*d*g*lambda2*lambda3*m^2*mu_s^2*cos(gamma1)*cos(theta) - 3*L2*d*g*lambda2*lambda3*m^2*mu_s^2*cos(gamma2)*cos(theta) + L1*d*ddx_des*lambda1*lambda3*m^2*mu_s^2*cos(gamma1)*sin(theta) - L1*d*ddx_des*lambda1*lambda3*m^2*mu_s^2*cos(theta)*sin(gamma1) - 3*L2*d*ddx_des*lambda1*lambda3*m^2*mu_s^2*cos(gamma2)*sin(theta) - L2*d*ddx_des*lambda1*lambda3*m^2*mu_s^2*cos(theta)*sin(gamma2)))/(4*I^2*lambda1*lambda2*mu_s^2 + L1^2*lambda2*lambda3*m^2*sin(gamma1)^2 + L2^2*lambda2*lambda3*m^2*sin(gamma2)^2 + L1^2*lambda2*lambda3*m^2*mu_s^2*cos(gamma1)^2 + L1^2*lambda1*lambda3*m^2*mu_s^4*cos(gamma1)^2 + L2^2*lambda2*lambda3*m^2*mu_s^2*cos(gamma2)^2 + L2^2*lambda1*lambda3*m^2*mu_s^4*cos(gamma2)^2 + L1^2*lambda1*lambda3*m^2*mu_s^2*sin(gamma1)^2 + L2^2*lambda1*lambda3*m^2*mu_s^2*sin(gamma2)^2 + 4*d^2*lambda2*lambda3*m^2*mu_s^2*cos(theta)^2 + 4*d^2*lambda1*lambda3*m^2*mu_s^2*sin(theta)^2 + 2*L1^2*lambda1*lambda3*m^2*mu_s^3*cos(gamma1)*sin(gamma1) - 2*L2^2*lambda1*lambda3*m^2*mu_s^3*cos(gamma2)*sin(gamma2) - 2*L1*L2*lambda2*lambda3*m^2*sin(gamma1)*sin(gamma2) + 2*L1^2*lambda2*lambda3*m^2*mu_s*cos(gamma1)*sin(gamma1) - 2*L2^2*lambda2*lambda3*m^2*mu_s*cos(gamma2)*sin(gamma2) + 2*L1*L2*lambda1*lambda3*m^2*mu_s^3*cos(gamma1)*sin(gamma2) - 2*L1*L2*lambda1*lambda3*m^2*mu_s^3*cos(gamma2)*sin(gamma1) + 2*L1*L2*lambda1*lambda3*m^2*mu_s^2*sin(gamma1)*sin(gamma2) - 4*L1*d*lambda2*lambda3*m^2*mu_s^2*cos(gamma1)*cos(theta) - 4*L2*d*lambda2*lambda3*m^2*mu_s^2*cos(gamma2)*cos(theta) - 4*L1*d*lambda1*lambda3*m^2*mu_s^3*cos(gamma1)*sin(theta) + 4*L2*d*lambda1*lambda3*m^2*mu_s^3*cos(gamma2)*sin(theta) - 4*L1*d*lambda1*lambda3*m^2*mu_s^2*sin(gamma1)*sin(theta) - 4*L2*d*lambda1*lambda3*m^2*mu_s^2*sin(gamma2)*sin(theta) - 2*L1*L2*lambda2*lambda3*m^2*mu_s*cos(gamma1)*sin(gamma2) + 2*L1*L2*lambda2*lambda3*m^2*mu_s*cos(gamma2)*sin(gamma1) - 4*L1*d*lambda2*lambda3*m^2*mu_s*cos(theta)*sin(gamma1) + 4*L2*d*lambda2*lambda3*m^2*mu_s*cos(theta)*sin(gamma2) + 2*L1*L2*lambda2*lambda3*m^2*mu_s^2*cos(gamma1)*cos(gamma2) - 2*L1*L2*lambda1*lambda3*m^2*mu_s^4*cos(gamma1)*cos(gamma2));
    (m*mu_s*(2*I^2*ddy_des*lambda1*lambda2*mu_s^2 + 2*I^2*g*lambda1*lambda2*mu_s^2 + 2*I^2*ddx_des*lambda1*lambda2*mu_s + L2^2*ddy_des*lambda2*lambda3*m^2*sin(gamma2)^2 + L2^2*g*lambda2*lambda3*m^2*sin(gamma2)^2 + L2^2*ddx_des*lambda1*lambda3*m^2*mu_s^3*cos(gamma2)^2 + L2^2*ddy_des*lambda2*lambda3*m^2*mu_s^2*cos(gamma2)^2 + L2^2*g*lambda2*lambda3*m^2*mu_s^2*cos(gamma2)^2 + 2*d^2*ddy_des*lambda2*lambda3*m^2*mu_s^2*cos(theta)^2 + 2*d^2*g*lambda2*lambda3*m^2*mu_s^2*cos(theta)^2 - I*L1*ddtheta_des*lambda2*lambda3*m*sin(gamma1) + I*L2*ddtheta_des*lambda2*lambda3*m*sin(gamma2) + L2^2*ddx_des*lambda1*lambda3*m^2*mu_s*sin(gamma2)^2 + 2*d^2*ddx_des*lambda1*lambda3*m^2*mu_s*sin(theta)^2 + 2*L2^2*ddy_des*lambda2*lambda3*m^2*mu_s*cos(gamma2)*sin(gamma2) + 2*L2^2*g*lambda2*lambda3*m^2*mu_s*cos(gamma2)*sin(gamma2) + I*L1*ddtheta_des*lambda1*lambda3*m*mu_s^3*cos(gamma1) - I*L2*ddtheta_des*lambda1*lambda3*m*mu_s^3*cos(gamma2) - I*L1*ddtheta_des*lambda1*lambda3*m*mu_s^2*sin(gamma1) - I*L2*ddtheta_des*lambda1*lambda3*m*mu_s^2*sin(gamma2) + 2*d^2*ddy_des*lambda2*lambda3*m^2*mu_s*cos(theta)*sin(theta) + 2*d^2*g*lambda2*lambda3*m^2*mu_s*cos(theta)*sin(theta) + 2*I*d*ddtheta_des*lambda1*lambda3*m*mu_s^2*sin(theta) + 2*L2^2*ddx_des*lambda1*lambda3*m^2*mu_s^2*cos(gamma2)*sin(gamma2) - L1*L2*ddy_des*lambda2*lambda3*m^2*sin(gamma1)*sin(gamma2) + 2*d^2*ddx_des*lambda1*lambda3*m^2*mu_s^2*cos(theta)*sin(theta) - L1*L2*g*lambda2*lambda3*m^2*sin(gamma1)*sin(gamma2) + I*L1*ddtheta_des*lambda2*lambda3*m*mu_s*cos(gamma1) + I*L2*ddtheta_des*lambda2*lambda3*m*mu_s*cos(gamma2) + L1*d*ddy_des*lambda2*lambda3*m^2*sin(gamma1)*sin(theta) - L2*d*ddy_des*lambda2*lambda3*m^2*sin(gamma2)*sin(theta) + L1*d*g*lambda2*lambda3*m^2*sin(gamma1)*sin(theta) - L2*d*g*lambda2*lambda3*m^2*sin(gamma2)*sin(theta) - 2*I*d*ddtheta_des*lambda2*lambda3*m*mu_s*cos(theta) + L1*L2*ddy_des*lambda2*lambda3*m^2*mu_s*cos(gamma1)*sin(gamma2) - L1*L2*ddy_des*lambda2*lambda3*m^2*mu_s*cos(gamma2)*sin(gamma1) + L1*L2*g*lambda2*lambda3*m^2*mu_s*cos(gamma1)*sin(gamma2) - L1*L2*g*lambda2*lambda3*m^2*mu_s*cos(gamma2)*sin(gamma1) + L1*L2*ddx_des*lambda1*lambda3*m^2*mu_s*sin(gamma1)*sin(gamma2) - L1*d*ddy_des*lambda2*lambda3*m^2*mu_s*cos(gamma1)*sin(theta) + L1*d*ddy_des*lambda2*lambda3*m^2*mu_s*cos(theta)*sin(gamma1) - L2*d*ddy_des*lambda2*lambda3*m^2*mu_s*cos(gamma2)*sin(theta) - 3*L2*d*ddy_des*lambda2*lambda3*m^2*mu_s*cos(theta)*sin(gamma2) - L1*d*g*lambda2*lambda3*m^2*mu_s*cos(gamma1)*sin(theta) + L1*d*g*lambda2*lambda3*m^2*mu_s*cos(theta)*sin(gamma1) - L2*d*g*lambda2*lambda3*m^2*mu_s*cos(gamma2)*sin(theta) - 3*L2*d*g*lambda2*lambda3*m^2*mu_s*cos(theta)*sin(gamma2) - L1*d*ddx_des*lambda1*lambda3*m^2*mu_s*sin(gamma1)*sin(theta) - 3*L2*d*ddx_des*lambda1*lambda3*m^2*mu_s*sin(gamma2)*sin(theta) - L1*L2*ddx_des*lambda1*lambda3*m^2*mu_s^3*cos(gamma1)*cos(gamma2) + L1*L2*ddy_des*lambda2*lambda3*m^2*mu_s^2*cos(gamma1)*cos(gamma2) + L1*L2*g*lambda2*lambda3*m^2*mu_s^2*cos(gamma1)*cos(gamma2) - L1*L2*ddx_des*lambda1*lambda3*m^2*mu_s^2*cos(gamma1)*sin(gamma2) + L1*L2*ddx_des*lambda1*lambda3*m^2*mu_s^2*cos(gamma2)*sin(gamma1) + L1*d*ddx_des*lambda1*lambda3*m^2*mu_s^3*cos(gamma1)*cos(theta) - L2*d*ddx_des*lambda1*lambda3*m^2*mu_s^3*cos(gamma2)*cos(theta) - L1*d*ddy_des*lambda2*lambda3*m^2*mu_s^2*cos(gamma1)*cos(theta) - 3*L2*d*ddy_des*lambda2*lambda3*m^2*mu_s^2*cos(gamma2)*cos(theta) - L1*d*g*lambda2*lambda3*m^2*mu_s^2*cos(gamma1)*cos(theta) - 3*L2*d*g*lambda2*lambda3*m^2*mu_s^2*cos(gamma2)*cos(theta) + L1*d*ddx_des*lambda1*lambda3*m^2*mu_s^2*cos(gamma1)*sin(theta) - L1*d*ddx_des*lambda1*lambda3*m^2*mu_s^2*cos(theta)*sin(gamma1) - 3*L2*d*ddx_des*lambda1*lambda3*m^2*mu_s^2*cos(gamma2)*sin(theta) - L2*d*ddx_des*lambda1*lambda3*m^2*mu_s^2*cos(theta)*sin(gamma2)))/(4*I^2*lambda1*lambda2*mu_s^2 + L1^2*lambda2*lambda3*m^2*sin(gamma1)^2 + L2^2*lambda2*lambda3*m^2*sin(gamma2)^2 + L1^2*lambda2*lambda3*m^2*mu_s^2*cos(gamma1)^2 + L1^2*lambda1*lambda3*m^2*mu_s^4*cos(gamma1)^2 + L2^2*lambda2*lambda3*m^2*mu_s^2*cos(gamma2)^2 + L2^2*lambda1*lambda3*m^2*mu_s^4*cos(gamma2)^2 + L1^2*lambda1*lambda3*m^2*mu_s^2*sin(gamma1)^2 + L2^2*lambda1*lambda3*m^2*mu_s^2*sin(gamma2)^2 + 4*d^2*lambda2*lambda3*m^2*mu_s^2*cos(theta)^2 + 4*d^2*lambda1*lambda3*m^2*mu_s^2*sin(theta)^2 - 2*L1^2*lambda1*lambda3*m^2*mu_s^3*cos(gamma1)*sin(gamma1) + 2*L2^2*lambda1*lambda3*m^2*mu_s^3*cos(gamma2)*sin(gamma2) - 2*L1*L2*lambda2*lambda3*m^2*sin(gamma1)*sin(gamma2) - 2*L1^2*lambda2*lambda3*m^2*mu_s*cos(gamma1)*sin(gamma1) + 2*L2^2*lambda2*lambda3*m^2*mu_s*cos(gamma2)*sin(gamma2) - 2*L1*L2*lambda1*lambda3*m^2*mu_s^3*cos(gamma1)*sin(gamma2) + 2*L1*L2*lambda1*lambda3*m^2*mu_s^3*cos(gamma2)*sin(gamma1) + 2*L1*L2*lambda1*lambda3*m^2*mu_s^2*sin(gamma1)*sin(gamma2) - 4*L1*d*lambda2*lambda3*m^2*mu_s^2*cos(gamma1)*cos(theta) - 4*L2*d*lambda2*lambda3*m^2*mu_s^2*cos(gamma2)*cos(theta) + 4*L1*d*lambda1*lambda3*m^2*mu_s^3*cos(gamma1)*sin(theta) - 4*L2*d*lambda1*lambda3*m^2*mu_s^3*cos(gamma2)*sin(theta) - 4*L1*d*lambda1*lambda3*m^2*mu_s^2*sin(gamma1)*sin(theta) - 4*L2*d*lambda1*lambda3*m^2*mu_s^2*sin(gamma2)*sin(theta) + 2*L1*L2*lambda2*lambda3*m^2*mu_s*cos(gamma1)*sin(gamma2) - 2*L1*L2*lambda2*lambda3*m^2*mu_s*cos(gamma2)*sin(gamma1) + 4*L1*d*lambda2*lambda3*m^2*mu_s*cos(theta)*sin(gamma1) - 4*L2*d*lambda2*lambda3*m^2*mu_s*cos(theta)*sin(gamma2) + 2*L1*L2*lambda2*lambda3*m^2*mu_s^2*cos(gamma1)*cos(gamma2) - 2*L1*L2*lambda1*lambda3*m^2*mu_s^4*cos(gamma1)*cos(gamma2));
    ]);

f2 = real([                                                                                                                                                                                                                                                                                                                                                                                                                                                                                                                                                                                                                                                                                                                                                                                                                                                                                                                                                                                                                                                                                                                                                                                                                                                                                                                                                                                                                                                                                                                                                                                                                                                                                                                                                                                                                                                                                                                                                                                                                                                                                                                                                                                                                                                                                                                                                                                                                                                                                                                                                                                                                                                                                                                                                                                                                                                                                                                                                                                                                                                                                                                                                                                                                                                                                                                                                                                                                                                                                                                                                                                                                                                                                                                                                                                                                                                                                                                                                                                                                                                                                                                                                                                                                                                                                                                                                                                                                                                                                                                                                                                                                                                                                                                                                                                                                                                                                                                                                                                                                                                                                                                                                                                                                                                                                                                                                                                                                                                                                                                                                                                                                   m*(ddy_des + g);
    0;
    (m*(I^2*ddy_des*lambda1*lambda2 + I^2*g*lambda1*lambda2 + L1^2*ddy_des*lambda2*lambda3*m^2*cos(gamma1)^2 + L1^2*g*lambda2*lambda3*m^2*cos(gamma1)^2 + d^2*ddy_des*lambda2*lambda3*m^2*cos(theta)^2 + d^2*g*lambda2*lambda3*m^2*cos(theta)^2 - I*L1*ddtheta_des*lambda1*lambda3*m*sin(gamma1) + I*d*ddtheta_des*lambda1*lambda3*m*sin(theta) + L1^2*ddx_des*lambda1*lambda3*m^2*cos(gamma1)*sin(gamma1) + d^2*ddx_des*lambda1*lambda3*m^2*cos(theta)*sin(theta) - 2*L1*d*ddy_des*lambda2*lambda3*m^2*cos(gamma1)*cos(theta) - 2*L1*d*g*lambda2*lambda3*m^2*cos(gamma1)*cos(theta) - L1*d*ddx_des*lambda1*lambda3*m^2*cos(gamma1)*sin(theta) - L1*d*ddx_des*lambda1*lambda3*m^2*cos(theta)*sin(gamma1)))/(I^2*lambda1*lambda2 + d^2*lambda1*lambda3*m^2*sin(theta)^2 + L1^2*lambda2*lambda3*m^2*cos(gamma1)^2 + L1^2*lambda1*lambda3*m^2*sin(gamma1)^2 + d^2*lambda2*lambda3*m^2*cos(theta)^2 - 2*L1*d*lambda2*lambda3*m^2*cos(gamma1)*cos(theta) - 2*L1*d*lambda1*lambda3*m^2*sin(gamma1)*sin(theta));
    0;
    0;
    0;
    0;
    0;
    ddy_des*m + g*m;
    0;
    (m*(I^2*ddy_des*lambda1*lambda2 + I^2*g*lambda1*lambda2 + L1^2*ddy_des*lambda2*lambda3*m^2*cos(gamma1)^2 + L1^2*g*lambda2*lambda3*m^2*cos(gamma1)^2 + d^2*ddy_des*lambda2*lambda3*m^2*cos(theta)^2 + d^2*g*lambda2*lambda3*m^2*cos(theta)^2 - I*L1*ddtheta_des*lambda1*lambda3*m*sin(gamma1) + I*d*ddtheta_des*lambda1*lambda3*m*sin(theta) + L1^2*ddx_des*lambda1*lambda3*m^2*cos(gamma1)*sin(gamma1) + d^2*ddx_des*lambda1*lambda3*m^2*cos(theta)*sin(theta) - 2*L1*d*ddy_des*lambda2*lambda3*m^2*cos(gamma1)*cos(theta) - 2*L1*d*g*lambda2*lambda3*m^2*cos(gamma1)*cos(theta) - L1*d*ddx_des*lambda1*lambda3*m^2*cos(gamma1)*sin(theta) - L1*d*ddx_des*lambda1*lambda3*m^2*cos(theta)*sin(gamma1)))/(I^2*lambda1*lambda2 + d^2*lambda1*lambda3*m^2*sin(theta)^2 + L1^2*lambda2*lambda3*m^2*cos(gamma1)^2 + L1^2*lambda1*lambda3*m^2*sin(gamma1)^2 + d^2*lambda2*lambda3*m^2*cos(theta)^2 - 2*L1*d*lambda2*lambda3*m^2*cos(gamma1)*cos(theta) - 2*L1*d*lambda1*lambda3*m^2*sin(gamma1)*sin(theta));
    0;
    0;
    0;
    0;
    0;
    -(I*ddtheta_des - L1*ddx_des*m*cos(gamma1) + L2*ddy_des*m*sin(gamma2) + L2*g*m*sin(gamma2) + d*ddx_des*m*cos(theta) - d*ddy_des*m*sin(theta) - d*g*m*sin(theta) - L1*ddy_des*m*mu_s*cos(gamma1) + L2*ddy_des*m*mu_s*cos(gamma2) - L1*g*m*mu_s*cos(gamma1) + L2*g*m*mu_s*cos(gamma2))/(L1*sin(gamma1) - L2*sin(gamma2) + L1*mu_s*cos(gamma1) - L2*mu_s*cos(gamma2));
    -(I*ddtheta_des - L1*ddx_des*m*cos(gamma1) + L2*ddy_des*m*sin(gamma2) + L2*g*m*sin(gamma2) + d*ddx_des*m*cos(theta) - d*ddy_des*m*sin(theta) - d*g*m*sin(theta) + L1*ddy_des*m*mu_s*cos(gamma1) - L2*ddy_des*m*mu_s*cos(gamma2) + L1*g*m*mu_s*cos(gamma1) - L2*g*m*mu_s*cos(gamma2))/(L1*sin(gamma1) - L2*sin(gamma2) - L1*mu_s*cos(gamma1) + L2*mu_s*cos(gamma2));
    -(I*ddtheta_des - L2*ddx_des*m*cos(gamma2) + L2*ddy_des*m*sin(gamma2) + L2*g*m*sin(gamma2) + d*ddx_des*m*cos(theta) - d*ddy_des*m*sin(theta) - d*g*m*sin(theta))/(L1*sin(gamma1) - L2*sin(gamma2) + L1*mu_s*cos(gamma1) - L2*mu_s*cos(gamma2));
    -(I*ddtheta_des - L2*ddx_des*m*cos(gamma2) + L2*ddy_des*m*sin(gamma2) + L2*g*m*sin(gamma2) + d*ddx_des*m*cos(theta) - d*ddy_des*m*sin(theta) - d*g*m*sin(theta))/(L1*sin(gamma1) - L2*sin(gamma2) - L1*mu_s*cos(gamma1) + L2*mu_s*cos(gamma2));
    (m*(I^2*ddy_des*lambda1*lambda2 + I^2*g*lambda1*lambda2 + L2^2*ddy_des*lambda2*lambda3*m^2*cos(gamma2)^2 + L2^2*g*lambda2*lambda3*m^2*cos(gamma2)^2 + d^2*ddy_des*lambda2*lambda3*m^2*cos(theta)^2 + d^2*g*lambda2*lambda3*m^2*cos(theta)^2 - I*L1*ddtheta_des*lambda1*lambda3*m*sin(gamma1) + I*d*ddtheta_des*lambda1*lambda3*m*sin(theta) + L2^2*ddx_des*lambda1*lambda3*m^2*mu_s*cos(gamma2)^2 + d^2*ddx_des*lambda1*lambda3*m^2*cos(theta)*sin(theta) + L1*L2*ddx_des*lambda1*lambda3*m^2*cos(gamma2)*sin(gamma1) - 2*L2*d*ddy_des*lambda2*lambda3*m^2*cos(gamma2)*cos(theta) - 2*L2*d*g*lambda2*lambda3*m^2*cos(gamma2)*cos(theta) - L1*d*ddx_des*lambda1*lambda3*m^2*cos(theta)*sin(gamma1) - L2*d*ddx_des*lambda1*lambda3*m^2*cos(gamma2)*sin(theta) + I*L1*ddtheta_des*lambda1*lambda3*m*mu_s*cos(gamma1) - I*L2*ddtheta_des*lambda1*lambda3*m*mu_s*cos(gamma2) - L1*L2*ddx_des*lambda1*lambda3*m^2*mu_s*cos(gamma1)*cos(gamma2) + L1*d*ddx_des*lambda1*lambda3*m^2*mu_s*cos(gamma1)*cos(theta) - L2*d*ddx_des*lambda1*lambda3*m^2*mu_s*cos(gamma2)*cos(theta)))/(I^2*lambda1*lambda2 + d^2*lambda1*lambda3*m^2*sin(theta)^2 + L2^2*lambda2*lambda3*m^2*cos(gamma2)^2 + L1^2*lambda1*lambda3*m^2*sin(gamma1)^2 + d^2*lambda2*lambda3*m^2*cos(theta)^2 + L1^2*lambda1*lambda3*m^2*mu_s^2*cos(gamma1)^2 + L2^2*lambda1*lambda3*m^2*mu_s^2*cos(gamma2)^2 - 2*L2*d*lambda2*lambda3*m^2*cos(gamma2)*cos(theta) - 2*L1*d*lambda1*lambda3*m^2*sin(gamma1)*sin(theta) - 2*L1^2*lambda1*lambda3*m^2*mu_s*cos(gamma1)*sin(gamma1) + 2*L1*L2*lambda1*lambda3*m^2*mu_s*cos(gamma2)*sin(gamma1) + 2*L1*d*lambda1*lambda3*m^2*mu_s*cos(gamma1)*sin(theta) - 2*L2*d*lambda1*lambda3*m^2*mu_s*cos(gamma2)*sin(theta) - 2*L1*L2*lambda1*lambda3*m^2*mu_s^2*cos(gamma1)*cos(gamma2));
    0;
    (I*m*(I*ddy_des*lambda2 + I*g*lambda2 + I*ddx_des*lambda1*mu_s - L1*ddtheta_des*lambda3*m*sin(gamma1) + d*ddtheta_des*lambda3*m*sin(theta) + L1*ddtheta_des*lambda3*m*mu_s*cos(gamma1) - d*ddtheta_des*lambda3*m*mu_s*cos(theta)))/(I^2*lambda2 + I^2*lambda1*mu_s^2 + L1^2*lambda3*m^2*sin(gamma1)^2 + d^2*lambda3*m^2*sin(theta)^2 + L1^2*lambda3*m^2*mu_s^2*cos(gamma1)^2 + d^2*lambda3*m^2*mu_s^2*cos(theta)^2 - 2*L1*d*lambda3*m^2*sin(gamma1)*sin(theta) - 2*L1^2*lambda3*m^2*mu_s*cos(gamma1)*sin(gamma1) - 2*d^2*lambda3*m^2*mu_s*cos(theta)*sin(theta) + 2*L1*d*lambda3*m^2*mu_s*cos(gamma1)*sin(theta) + 2*L1*d*lambda3*m^2*mu_s*cos(theta)*sin(gamma1) - 2*L1*d*lambda3*m^2*mu_s^2*cos(gamma1)*cos(theta));
    (I*m*(I*ddy_des*lambda2 + I*g*lambda2 - I*ddx_des*lambda1*mu_s - L1*ddtheta_des*lambda3*m*sin(gamma1) + d*ddtheta_des*lambda3*m*sin(theta) - L1*ddtheta_des*lambda3*m*mu_s*cos(gamma1) + d*ddtheta_des*lambda3*m*mu_s*cos(theta)))/(I^2*lambda2 + I^2*lambda1*mu_s^2 + L1^2*lambda3*m^2*sin(gamma1)^2 + d^2*lambda3*m^2*sin(theta)^2 + L1^2*lambda3*m^2*mu_s^2*cos(gamma1)^2 + d^2*lambda3*m^2*mu_s^2*cos(theta)^2 - 2*L1*d*lambda3*m^2*sin(gamma1)*sin(theta) + 2*L1^2*lambda3*m^2*mu_s*cos(gamma1)*sin(gamma1) + 2*d^2*lambda3*m^2*mu_s*cos(theta)*sin(theta) - 2*L1*d*lambda3*m^2*mu_s*cos(gamma1)*sin(theta) - 2*L1*d*lambda3*m^2*mu_s*cos(theta)*sin(gamma1) - 2*L1*d*lambda3*m^2*mu_s^2*cos(gamma1)*cos(theta));
    0;
    0;
    0;
    -(I*ddtheta_des*lambda2 + I*ddtheta_des*lambda1*mu_s^2 + L2*ddy_des*lambda2*m*sin(gamma2) + L2*g*lambda2*m*sin(gamma2) - d*ddy_des*lambda2*m*sin(theta) - d*g*lambda2*m*sin(theta) + L2*ddy_des*lambda2*m*mu_s*cos(gamma2) + L2*g*lambda2*m*mu_s*cos(gamma2) - L2*ddx_des*lambda1*m*mu_s*sin(gamma2) - d*ddy_des*lambda2*m*mu_s*cos(theta) - d*g*lambda2*m*mu_s*cos(theta) + d*ddx_des*lambda1*m*mu_s*sin(theta) - L2*ddx_des*lambda1*m*mu_s^2*cos(gamma2) + d*ddx_des*lambda1*m*mu_s^2*cos(theta))/((lambda1*mu_s^2 + lambda2)*(L1*sin(gamma1) - L2*sin(gamma2) + L1*mu_s*cos(gamma1) - L2*mu_s*cos(gamma2)));
    -(I*ddtheta_des*lambda2 + I*ddtheta_des*lambda1*mu_s^2 + L2*ddy_des*lambda2*m*sin(gamma2) + L2*g*lambda2*m*sin(gamma2) - d*ddy_des*lambda2*m*sin(theta) - d*g*lambda2*m*sin(theta) - L2*ddy_des*lambda2*m*mu_s*cos(gamma2) - L2*g*lambda2*m*mu_s*cos(gamma2) + L2*ddx_des*lambda1*m*mu_s*sin(gamma2) + d*ddy_des*lambda2*m*mu_s*cos(theta) + d*g*lambda2*m*mu_s*cos(theta) - d*ddx_des*lambda1*m*mu_s*sin(theta) - L2*ddx_des*lambda1*m*mu_s^2*cos(gamma2) + d*ddx_des*lambda1*m*mu_s^2*cos(theta))/((lambda1*mu_s^2 + lambda2)*(L1*sin(gamma1) - L2*sin(gamma2) - L1*mu_s*cos(gamma1) + L2*mu_s*cos(gamma2)));
    (m*(I^2*ddy_des*lambda1*lambda2 + I^2*g*lambda1*lambda2 + L2^2*ddy_des*lambda2*lambda3*m^2*cos(gamma2)^2 + L2^2*g*lambda2*lambda3*m^2*cos(gamma2)^2 + d^2*ddy_des*lambda2*lambda3*m^2*cos(theta)^2 + d^2*g*lambda2*lambda3*m^2*cos(theta)^2 - I*L1*ddtheta_des*lambda1*lambda3*m*sin(gamma1) + I*d*ddtheta_des*lambda1*lambda3*m*sin(theta) - L2^2*ddx_des*lambda1*lambda3*m^2*mu_s*cos(gamma2)^2 + d^2*ddx_des*lambda1*lambda3*m^2*cos(theta)*sin(theta) + L1*L2*ddx_des*lambda1*lambda3*m^2*cos(gamma2)*sin(gamma1) - 2*L2*d*ddy_des*lambda2*lambda3*m^2*cos(gamma2)*cos(theta) - 2*L2*d*g*lambda2*lambda3*m^2*cos(gamma2)*cos(theta) - L1*d*ddx_des*lambda1*lambda3*m^2*cos(theta)*sin(gamma1) - L2*d*ddx_des*lambda1*lambda3*m^2*cos(gamma2)*sin(theta) - I*L1*ddtheta_des*lambda1*lambda3*m*mu_s*cos(gamma1) + I*L2*ddtheta_des*lambda1*lambda3*m*mu_s*cos(gamma2) + L1*L2*ddx_des*lambda1*lambda3*m^2*mu_s*cos(gamma1)*cos(gamma2) - L1*d*ddx_des*lambda1*lambda3*m^2*mu_s*cos(gamma1)*cos(theta) + L2*d*ddx_des*lambda1*lambda3*m^2*mu_s*cos(gamma2)*cos(theta)))/(I^2*lambda1*lambda2 + d^2*lambda1*lambda3*m^2*sin(theta)^2 + L2^2*lambda2*lambda3*m^2*cos(gamma2)^2 + L1^2*lambda1*lambda3*m^2*sin(gamma1)^2 + d^2*lambda2*lambda3*m^2*cos(theta)^2 + L1^2*lambda1*lambda3*m^2*mu_s^2*cos(gamma1)^2 + L2^2*lambda1*lambda3*m^2*mu_s^2*cos(gamma2)^2 - 2*L2*d*lambda2*lambda3*m^2*cos(gamma2)*cos(theta) - 2*L1*d*lambda1*lambda3*m^2*sin(gamma1)*sin(theta) + 2*L1^2*lambda1*lambda3*m^2*mu_s*cos(gamma1)*sin(gamma1) - 2*L1*L2*lambda1*lambda3*m^2*mu_s*cos(gamma2)*sin(gamma1) - 2*L1*d*lambda1*lambda3*m^2*mu_s*cos(gamma1)*sin(theta) + 2*L2*d*lambda1*lambda3*m^2*mu_s*cos(gamma2)*sin(theta) - 2*L1*L2*lambda1*lambda3*m^2*mu_s^2*cos(gamma1)*cos(gamma2));
    0;
    0;
    0;
    (m*(I^2*ddy_des*lambda1*lambda2 + I^2*g*lambda1*lambda2 + L1^2*ddy_des*lambda2*lambda3*m^2*cos(gamma1)^2 + L1^2*g*lambda2*lambda3*m^2*cos(gamma1)^2 + d^2*ddy_des*lambda2*lambda3*m^2*cos(theta)^2 + d^2*g*lambda2*lambda3*m^2*cos(theta)^2 - I*L1*ddtheta_des*lambda1*lambda3*m*sin(gamma1) + I*d*ddtheta_des*lambda1*lambda3*m*sin(theta) + L1^2*ddx_des*lambda1*lambda3*m^2*cos(gamma1)*sin(gamma1) + d^2*ddx_des*lambda1*lambda3*m^2*cos(theta)*sin(theta) - 2*L1*d*ddy_des*lambda2*lambda3*m^2*cos(gamma1)*cos(theta) - 2*L1*d*g*lambda2*lambda3*m^2*cos(gamma1)*cos(theta) - L1*d*ddx_des*lambda1*lambda3*m^2*cos(gamma1)*sin(theta) - L1*d*ddx_des*lambda1*lambda3*m^2*cos(theta)*sin(gamma1)))/(I^2*lambda1*lambda2 + d^2*lambda1*lambda3*m^2*sin(theta)^2 + L1^2*lambda2*lambda3*m^2*cos(gamma1)^2 + L1^2*lambda1*lambda3*m^2*sin(gamma1)^2 + d^2*lambda2*lambda3*m^2*cos(theta)^2 - 2*L1*d*lambda2*lambda3*m^2*cos(gamma1)*cos(theta) - 2*L1*d*lambda1*lambda3*m^2*sin(gamma1)*sin(theta));
    (m*(I^2*ddy_des*lambda1*lambda2 + I^2*g*lambda1*lambda2 + L1^2*ddy_des*lambda2*lambda3*m^2*cos(gamma1)^2 + L1^2*g*lambda2*lambda3*m^2*cos(gamma1)^2 + d^2*ddy_des*lambda2*lambda3*m^2*cos(theta)^2 + d^2*g*lambda2*lambda3*m^2*cos(theta)^2 - I*L1*ddtheta_des*lambda1*lambda3*m*sin(gamma1) + I*d*ddtheta_des*lambda1*lambda3*m*sin(theta) + L1^2*ddx_des*lambda1*lambda3*m^2*cos(gamma1)*sin(gamma1) + d^2*ddx_des*lambda1*lambda3*m^2*cos(theta)*sin(theta) - 2*L1*d*ddy_des*lambda2*lambda3*m^2*cos(gamma1)*cos(theta) - 2*L1*d*g*lambda2*lambda3*m^2*cos(gamma1)*cos(theta) - L1*d*ddx_des*lambda1*lambda3*m^2*cos(gamma1)*sin(theta) - L1*d*ddx_des*lambda1*lambda3*m^2*cos(theta)*sin(gamma1)))/(I^2*lambda1*lambda2 + d^2*lambda1*lambda3*m^2*sin(theta)^2 + L1^2*lambda2*lambda3*m^2*cos(gamma1)^2 + L1^2*lambda1*lambda3*m^2*sin(gamma1)^2 + d^2*lambda2*lambda3*m^2*cos(theta)^2 - 2*L1*d*lambda2*lambda3*m^2*cos(gamma1)*cos(theta) - 2*L1*d*lambda1*lambda3*m^2*sin(gamma1)*sin(theta));
    0;
    0;
    0;
    0;
    0;
    0;
    0;
    0;
    0;
    0;
    0;
    0;
    0;
    (I*m*(I*ddy_des*lambda2 + I*g*lambda2 + I*ddx_des*lambda1*mu_s - L1*ddtheta_des*lambda3*m*sin(gamma1) + d*ddtheta_des*lambda3*m*sin(theta) + L1*ddtheta_des*lambda3*m*mu_s*cos(gamma1) - d*ddtheta_des*lambda3*m*mu_s*cos(theta)))/(I^2*lambda2 + I^2*lambda1*mu_s^2 + L1^2*lambda3*m^2*sin(gamma1)^2 + d^2*lambda3*m^2*sin(theta)^2 + L1^2*lambda3*m^2*mu_s^2*cos(gamma1)^2 + d^2*lambda3*m^2*mu_s^2*cos(theta)^2 - 2*L1*d*lambda3*m^2*sin(gamma1)*sin(theta) - 2*L1^2*lambda3*m^2*mu_s*cos(gamma1)*sin(gamma1) - 2*d^2*lambda3*m^2*mu_s*cos(theta)*sin(theta) + 2*L1*d*lambda3*m^2*mu_s*cos(gamma1)*sin(theta) + 2*L1*d*lambda3*m^2*mu_s*cos(theta)*sin(gamma1) - 2*L1*d*lambda3*m^2*mu_s^2*cos(gamma1)*cos(theta));
    (I*m*(I*ddy_des*lambda2 + I*g*lambda2 - I*ddx_des*lambda1*mu_s - L1*ddtheta_des*lambda3*m*sin(gamma1) + d*ddtheta_des*lambda3*m*sin(theta) - L1*ddtheta_des*lambda3*m*mu_s*cos(gamma1) + d*ddtheta_des*lambda3*m*mu_s*cos(theta)))/(I^2*lambda2 + I^2*lambda1*mu_s^2 + L1^2*lambda3*m^2*sin(gamma1)^2 + d^2*lambda3*m^2*sin(theta)^2 + L1^2*lambda3*m^2*mu_s^2*cos(gamma1)^2 + d^2*lambda3*m^2*mu_s^2*cos(theta)^2 - 2*L1*d*lambda3*m^2*sin(gamma1)*sin(theta) + 2*L1^2*lambda3*m^2*mu_s*cos(gamma1)*sin(gamma1) + 2*d^2*lambda3*m^2*mu_s*cos(theta)*sin(theta) - 2*L1*d*lambda3*m^2*mu_s*cos(gamma1)*sin(theta) - 2*L1*d*lambda3*m^2*mu_s*cos(theta)*sin(gamma1) - 2*L1*d*lambda3*m^2*mu_s^2*cos(gamma1)*cos(theta));
    0;
    0;
    0;
    0;
    (I*m*(I*ddy_des*lambda2 + I*g*lambda2 - I*ddx_des*lambda1*mu_s - L1*ddtheta_des*lambda3*m*sin(gamma1) + d*ddtheta_des*lambda3*m*sin(theta) - L1*ddtheta_des*lambda3*m*mu_s*cos(gamma1) + d*ddtheta_des*lambda3*m*mu_s*cos(theta)))/(I^2*lambda2 + I^2*lambda1*mu_s^2 + L1^2*lambda3*m^2*sin(gamma1)^2 + d^2*lambda3*m^2*sin(theta)^2 + L1^2*lambda3*m^2*mu_s^2*cos(gamma1)^2 + d^2*lambda3*m^2*mu_s^2*cos(theta)^2 - 2*L1*d*lambda3*m^2*sin(gamma1)*sin(theta) + 2*L1^2*lambda3*m^2*mu_s*cos(gamma1)*sin(gamma1) + 2*d^2*lambda3*m^2*mu_s*cos(theta)*sin(theta) - 2*L1*d*lambda3*m^2*mu_s*cos(gamma1)*sin(theta) - 2*L1*d*lambda3*m^2*mu_s*cos(theta)*sin(gamma1) - 2*L1*d*lambda3*m^2*mu_s^2*cos(gamma1)*cos(theta));
    (I*m*(I*ddy_des*lambda2 + I*g*lambda2 + I*ddx_des*lambda1*mu_s - L1*ddtheta_des*lambda3*m*sin(gamma1) + d*ddtheta_des*lambda3*m*sin(theta) + L1*ddtheta_des*lambda3*m*mu_s*cos(gamma1) - d*ddtheta_des*lambda3*m*mu_s*cos(theta)))/(I^2*lambda2 + I^2*lambda1*mu_s^2 + L1^2*lambda3*m^2*sin(gamma1)^2 + d^2*lambda3*m^2*sin(theta)^2 + L1^2*lambda3*m^2*mu_s^2*cos(gamma1)^2 + d^2*lambda3*m^2*mu_s^2*cos(theta)^2 - 2*L1*d*lambda3*m^2*sin(gamma1)*sin(theta) - 2*L1^2*lambda3*m^2*mu_s*cos(gamma1)*sin(gamma1) - 2*d^2*lambda3*m^2*mu_s*cos(theta)*sin(theta) + 2*L1*d*lambda3*m^2*mu_s*cos(gamma1)*sin(theta) + 2*L1*d*lambda3*m^2*mu_s*cos(theta)*sin(gamma1) - 2*L1*d*lambda3*m^2*mu_s^2*cos(gamma1)*cos(theta));
    0;
    0;
    (I*m*(I*ddy_des*lambda2 + I*g*lambda2 + I*ddx_des*lambda1*mu_s - L1*ddtheta_des*lambda3*m*sin(gamma1) + d*ddtheta_des*lambda3*m*sin(theta) + L1*ddtheta_des*lambda3*m*mu_s*cos(gamma1) - d*ddtheta_des*lambda3*m*mu_s*cos(theta)))/(I^2*lambda2 + I^2*lambda1*mu_s^2 + L1^2*lambda3*m^2*sin(gamma1)^2 + d^2*lambda3*m^2*sin(theta)^2 + L1^2*lambda3*m^2*mu_s^2*cos(gamma1)^2 + d^2*lambda3*m^2*mu_s^2*cos(theta)^2 - 2*L1*d*lambda3*m^2*sin(gamma1)*sin(theta) - 2*L1^2*lambda3*m^2*mu_s*cos(gamma1)*sin(gamma1) - 2*d^2*lambda3*m^2*mu_s*cos(theta)*sin(theta) + 2*L1*d*lambda3*m^2*mu_s*cos(gamma1)*sin(theta) + 2*L1*d*lambda3*m^2*mu_s*cos(theta)*sin(gamma1) - 2*L1*d*lambda3*m^2*mu_s^2*cos(gamma1)*cos(theta));
    (I*m*(I*ddy_des*lambda2 + I*g*lambda2 - I*ddx_des*lambda1*mu_s - L1*ddtheta_des*lambda3*m*sin(gamma1) + d*ddtheta_des*lambda3*m*sin(theta) - L1*ddtheta_des*lambda3*m*mu_s*cos(gamma1) + d*ddtheta_des*lambda3*m*mu_s*cos(theta)))/(I^2*lambda2 + I^2*lambda1*mu_s^2 + L1^2*lambda3*m^2*sin(gamma1)^2 + d^2*lambda3*m^2*sin(theta)^2 + L1^2*lambda3*m^2*mu_s^2*cos(gamma1)^2 + d^2*lambda3*m^2*mu_s^2*cos(theta)^2 - 2*L1*d*lambda3*m^2*sin(gamma1)*sin(theta) + 2*L1^2*lambda3*m^2*mu_s*cos(gamma1)*sin(gamma1) + 2*d^2*lambda3*m^2*mu_s*cos(theta)*sin(theta) - 2*L1*d*lambda3*m^2*mu_s*cos(gamma1)*sin(theta) - 2*L1*d*lambda3*m^2*mu_s*cos(theta)*sin(gamma1) - 2*L1*d*lambda3*m^2*mu_s^2*cos(gamma1)*cos(theta));
    0;
    0;
    (m*(2*I^2*ddy_des*lambda1*lambda2*mu_s^2 + 2*I^2*g*lambda1*lambda2*mu_s^2 - 2*I^2*ddx_des*lambda1*lambda2*mu_s + L2^2*ddy_des*lambda2*lambda3*m^2*sin(gamma2)^2 + L2^2*g*lambda2*lambda3*m^2*sin(gamma2)^2 - L2^2*ddx_des*lambda1*lambda3*m^2*mu_s^3*cos(gamma2)^2 + L2^2*ddy_des*lambda2*lambda3*m^2*mu_s^2*cos(gamma2)^2 + L2^2*g*lambda2*lambda3*m^2*mu_s^2*cos(gamma2)^2 + 2*d^2*ddy_des*lambda2*lambda3*m^2*mu_s^2*cos(theta)^2 + 2*d^2*g*lambda2*lambda3*m^2*mu_s^2*cos(theta)^2 - I*L1*ddtheta_des*lambda2*lambda3*m*sin(gamma1) + I*L2*ddtheta_des*lambda2*lambda3*m*sin(gamma2) - L2^2*ddx_des*lambda1*lambda3*m^2*mu_s*sin(gamma2)^2 - 2*d^2*ddx_des*lambda1*lambda3*m^2*mu_s*sin(theta)^2 - 2*L2^2*ddy_des*lambda2*lambda3*m^2*mu_s*cos(gamma2)*sin(gamma2) - 2*L2^2*g*lambda2*lambda3*m^2*mu_s*cos(gamma2)*sin(gamma2) - I*L1*ddtheta_des*lambda1*lambda3*m*mu_s^3*cos(gamma1) + I*L2*ddtheta_des*lambda1*lambda3*m*mu_s^3*cos(gamma2) - I*L1*ddtheta_des*lambda1*lambda3*m*mu_s^2*sin(gamma1) - I*L2*ddtheta_des*lambda1*lambda3*m*mu_s^2*sin(gamma2) - 2*d^2*ddy_des*lambda2*lambda3*m^2*mu_s*cos(theta)*sin(theta) - 2*d^2*g*lambda2*lambda3*m^2*mu_s*cos(theta)*sin(theta) + 2*I*d*ddtheta_des*lambda1*lambda3*m*mu_s^2*sin(theta) + 2*L2^2*ddx_des*lambda1*lambda3*m^2*mu_s^2*cos(gamma2)*sin(gamma2) - L1*L2*ddy_des*lambda2*lambda3*m^2*sin(gamma1)*sin(gamma2) + 2*d^2*ddx_des*lambda1*lambda3*m^2*mu_s^2*cos(theta)*sin(theta) - L1*L2*g*lambda2*lambda3*m^2*sin(gamma1)*sin(gamma2) - I*L1*ddtheta_des*lambda2*lambda3*m*mu_s*cos(gamma1) - I*L2*ddtheta_des*lambda2*lambda3*m*mu_s*cos(gamma2) + L1*d*ddy_des*lambda2*lambda3*m^2*sin(gamma1)*sin(theta) - L2*d*ddy_des*lambda2*lambda3*m^2*sin(gamma2)*sin(theta) + L1*d*g*lambda2*lambda3*m^2*sin(gamma1)*sin(theta) - L2*d*g*lambda2*lambda3*m^2*sin(gamma2)*sin(theta) + 2*I*d*ddtheta_des*lambda2*lambda3*m*mu_s*cos(theta) - L1*L2*ddy_des*lambda2*lambda3*m^2*mu_s*cos(gamma1)*sin(gamma2) + L1*L2*ddy_des*lambda2*lambda3*m^2*mu_s*cos(gamma2)*sin(gamma1) - L1*L2*g*lambda2*lambda3*m^2*mu_s*cos(gamma1)*sin(gamma2) + L1*L2*g*lambda2*lambda3*m^2*mu_s*cos(gamma2)*sin(gamma1) - L1*L2*ddx_des*lambda1*lambda3*m^2*mu_s*sin(gamma1)*sin(gamma2) + L1*d*ddy_des*lambda2*lambda3*m^2*mu_s*cos(gamma1)*sin(theta) - L1*d*ddy_des*lambda2*lambda3*m^2*mu_s*cos(theta)*sin(gamma1) + L2*d*ddy_des*lambda2*lambda3*m^2*mu_s*cos(gamma2)*sin(theta) + 3*L2*d*ddy_des*lambda2*lambda3*m^2*mu_s*cos(theta)*sin(gamma2) + L1*d*g*lambda2*lambda3*m^2*mu_s*cos(gamma1)*sin(theta) - L1*d*g*lambda2*lambda3*m^2*mu_s*cos(theta)*sin(gamma1) + L2*d*g*lambda2*lambda3*m^2*mu_s*cos(gamma2)*sin(theta) + 3*L2*d*g*lambda2*lambda3*m^2*mu_s*cos(theta)*sin(gamma2) + L1*d*ddx_des*lambda1*lambda3*m^2*mu_s*sin(gamma1)*sin(theta) + 3*L2*d*ddx_des*lambda1*lambda3*m^2*mu_s*sin(gamma2)*sin(theta) + L1*L2*ddx_des*lambda1*lambda3*m^2*mu_s^3*cos(gamma1)*cos(gamma2) + L1*L2*ddy_des*lambda2*lambda3*m^2*mu_s^2*cos(gamma1)*cos(gamma2) + L1*L2*g*lambda2*lambda3*m^2*mu_s^2*cos(gamma1)*cos(gamma2) - L1*L2*ddx_des*lambda1*lambda3*m^2*mu_s^2*cos(gamma1)*sin(gamma2) + L1*L2*ddx_des*lambda1*lambda3*m^2*mu_s^2*cos(gamma2)*sin(gamma1) - L1*d*ddx_des*lambda1*lambda3*m^2*mu_s^3*cos(gamma1)*cos(theta) + L2*d*ddx_des*lambda1*lambda3*m^2*mu_s^3*cos(gamma2)*cos(theta) - L1*d*ddy_des*lambda2*lambda3*m^2*mu_s^2*cos(gamma1)*cos(theta) - 3*L2*d*ddy_des*lambda2*lambda3*m^2*mu_s^2*cos(gamma2)*cos(theta) - L1*d*g*lambda2*lambda3*m^2*mu_s^2*cos(gamma1)*cos(theta) - 3*L2*d*g*lambda2*lambda3*m^2*mu_s^2*cos(gamma2)*cos(theta) + L1*d*ddx_des*lambda1*lambda3*m^2*mu_s^2*cos(gamma1)*sin(theta) - L1*d*ddx_des*lambda1*lambda3*m^2*mu_s^2*cos(theta)*sin(gamma1) - 3*L2*d*ddx_des*lambda1*lambda3*m^2*mu_s^2*cos(gamma2)*sin(theta) - L2*d*ddx_des*lambda1*lambda3*m^2*mu_s^2*cos(theta)*sin(gamma2)))/(4*I^2*lambda1*lambda2*mu_s^2 + L1^2*lambda2*lambda3*m^2*sin(gamma1)^2 + L2^2*lambda2*lambda3*m^2*sin(gamma2)^2 + L1^2*lambda2*lambda3*m^2*mu_s^2*cos(gamma1)^2 + L1^2*lambda1*lambda3*m^2*mu_s^4*cos(gamma1)^2 + L2^2*lambda2*lambda3*m^2*mu_s^2*cos(gamma2)^2 + L2^2*lambda1*lambda3*m^2*mu_s^4*cos(gamma2)^2 + L1^2*lambda1*lambda3*m^2*mu_s^2*sin(gamma1)^2 + L2^2*lambda1*lambda3*m^2*mu_s^2*sin(gamma2)^2 + 4*d^2*lambda2*lambda3*m^2*mu_s^2*cos(theta)^2 + 4*d^2*lambda1*lambda3*m^2*mu_s^2*sin(theta)^2 + 2*L1^2*lambda1*lambda3*m^2*mu_s^3*cos(gamma1)*sin(gamma1) - 2*L2^2*lambda1*lambda3*m^2*mu_s^3*cos(gamma2)*sin(gamma2) - 2*L1*L2*lambda2*lambda3*m^2*sin(gamma1)*sin(gamma2) + 2*L1^2*lambda2*lambda3*m^2*mu_s*cos(gamma1)*sin(gamma1) - 2*L2^2*lambda2*lambda3*m^2*mu_s*cos(gamma2)*sin(gamma2) + 2*L1*L2*lambda1*lambda3*m^2*mu_s^3*cos(gamma1)*sin(gamma2) - 2*L1*L2*lambda1*lambda3*m^2*mu_s^3*cos(gamma2)*sin(gamma1) + 2*L1*L2*lambda1*lambda3*m^2*mu_s^2*sin(gamma1)*sin(gamma2) - 4*L1*d*lambda2*lambda3*m^2*mu_s^2*cos(gamma1)*cos(theta) - 4*L2*d*lambda2*lambda3*m^2*mu_s^2*cos(gamma2)*cos(theta) - 4*L1*d*lambda1*lambda3*m^2*mu_s^3*cos(gamma1)*sin(theta) + 4*L2*d*lambda1*lambda3*m^2*mu_s^3*cos(gamma2)*sin(theta) - 4*L1*d*lambda1*lambda3*m^2*mu_s^2*sin(gamma1)*sin(theta) - 4*L2*d*lambda1*lambda3*m^2*mu_s^2*sin(gamma2)*sin(theta) - 2*L1*L2*lambda2*lambda3*m^2*mu_s*cos(gamma1)*sin(gamma2) + 2*L1*L2*lambda2*lambda3*m^2*mu_s*cos(gamma2)*sin(gamma1) - 4*L1*d*lambda2*lambda3*m^2*mu_s*cos(theta)*sin(gamma1) + 4*L2*d*lambda2*lambda3*m^2*mu_s*cos(theta)*sin(gamma2) + 2*L1*L2*lambda2*lambda3*m^2*mu_s^2*cos(gamma1)*cos(gamma2) - 2*L1*L2*lambda1*lambda3*m^2*mu_s^4*cos(gamma1)*cos(gamma2));
    (m*(2*I^2*ddy_des*lambda1*lambda2*mu_s^2 + 2*I^2*g*lambda1*lambda2*mu_s^2 + 2*I^2*ddx_des*lambda1*lambda2*mu_s + L2^2*ddy_des*lambda2*lambda3*m^2*sin(gamma2)^2 + L2^2*g*lambda2*lambda3*m^2*sin(gamma2)^2 + L2^2*ddx_des*lambda1*lambda3*m^2*mu_s^3*cos(gamma2)^2 + L2^2*ddy_des*lambda2*lambda3*m^2*mu_s^2*cos(gamma2)^2 + L2^2*g*lambda2*lambda3*m^2*mu_s^2*cos(gamma2)^2 + 2*d^2*ddy_des*lambda2*lambda3*m^2*mu_s^2*cos(theta)^2 + 2*d^2*g*lambda2*lambda3*m^2*mu_s^2*cos(theta)^2 - I*L1*ddtheta_des*lambda2*lambda3*m*sin(gamma1) + I*L2*ddtheta_des*lambda2*lambda3*m*sin(gamma2) + L2^2*ddx_des*lambda1*lambda3*m^2*mu_s*sin(gamma2)^2 + 2*d^2*ddx_des*lambda1*lambda3*m^2*mu_s*sin(theta)^2 + 2*L2^2*ddy_des*lambda2*lambda3*m^2*mu_s*cos(gamma2)*sin(gamma2) + 2*L2^2*g*lambda2*lambda3*m^2*mu_s*cos(gamma2)*sin(gamma2) + I*L1*ddtheta_des*lambda1*lambda3*m*mu_s^3*cos(gamma1) - I*L2*ddtheta_des*lambda1*lambda3*m*mu_s^3*cos(gamma2) - I*L1*ddtheta_des*lambda1*lambda3*m*mu_s^2*sin(gamma1) - I*L2*ddtheta_des*lambda1*lambda3*m*mu_s^2*sin(gamma2) + 2*d^2*ddy_des*lambda2*lambda3*m^2*mu_s*cos(theta)*sin(theta) + 2*d^2*g*lambda2*lambda3*m^2*mu_s*cos(theta)*sin(theta) + 2*I*d*ddtheta_des*lambda1*lambda3*m*mu_s^2*sin(theta) + 2*L2^2*ddx_des*lambda1*lambda3*m^2*mu_s^2*cos(gamma2)*sin(gamma2) - L1*L2*ddy_des*lambda2*lambda3*m^2*sin(gamma1)*sin(gamma2) + 2*d^2*ddx_des*lambda1*lambda3*m^2*mu_s^2*cos(theta)*sin(theta) - L1*L2*g*lambda2*lambda3*m^2*sin(gamma1)*sin(gamma2) + I*L1*ddtheta_des*lambda2*lambda3*m*mu_s*cos(gamma1) + I*L2*ddtheta_des*lambda2*lambda3*m*mu_s*cos(gamma2) + L1*d*ddy_des*lambda2*lambda3*m^2*sin(gamma1)*sin(theta) - L2*d*ddy_des*lambda2*lambda3*m^2*sin(gamma2)*sin(theta) + L1*d*g*lambda2*lambda3*m^2*sin(gamma1)*sin(theta) - L2*d*g*lambda2*lambda3*m^2*sin(gamma2)*sin(theta) - 2*I*d*ddtheta_des*lambda2*lambda3*m*mu_s*cos(theta) + L1*L2*ddy_des*lambda2*lambda3*m^2*mu_s*cos(gamma1)*sin(gamma2) - L1*L2*ddy_des*lambda2*lambda3*m^2*mu_s*cos(gamma2)*sin(gamma1) + L1*L2*g*lambda2*lambda3*m^2*mu_s*cos(gamma1)*sin(gamma2) - L1*L2*g*lambda2*lambda3*m^2*mu_s*cos(gamma2)*sin(gamma1) + L1*L2*ddx_des*lambda1*lambda3*m^2*mu_s*sin(gamma1)*sin(gamma2) - L1*d*ddy_des*lambda2*lambda3*m^2*mu_s*cos(gamma1)*sin(theta) + L1*d*ddy_des*lambda2*lambda3*m^2*mu_s*cos(theta)*sin(gamma1) - L2*d*ddy_des*lambda2*lambda3*m^2*mu_s*cos(gamma2)*sin(theta) - 3*L2*d*ddy_des*lambda2*lambda3*m^2*mu_s*cos(theta)*sin(gamma2) - L1*d*g*lambda2*lambda3*m^2*mu_s*cos(gamma1)*sin(theta) + L1*d*g*lambda2*lambda3*m^2*mu_s*cos(theta)*sin(gamma1) - L2*d*g*lambda2*lambda3*m^2*mu_s*cos(gamma2)*sin(theta) - 3*L2*d*g*lambda2*lambda3*m^2*mu_s*cos(theta)*sin(gamma2) - L1*d*ddx_des*lambda1*lambda3*m^2*mu_s*sin(gamma1)*sin(theta) - 3*L2*d*ddx_des*lambda1*lambda3*m^2*mu_s*sin(gamma2)*sin(theta) - L1*L2*ddx_des*lambda1*lambda3*m^2*mu_s^3*cos(gamma1)*cos(gamma2) + L1*L2*ddy_des*lambda2*lambda3*m^2*mu_s^2*cos(gamma1)*cos(gamma2) + L1*L2*g*lambda2*lambda3*m^2*mu_s^2*cos(gamma1)*cos(gamma2) - L1*L2*ddx_des*lambda1*lambda3*m^2*mu_s^2*cos(gamma1)*sin(gamma2) + L1*L2*ddx_des*lambda1*lambda3*m^2*mu_s^2*cos(gamma2)*sin(gamma1) + L1*d*ddx_des*lambda1*lambda3*m^2*mu_s^3*cos(gamma1)*cos(theta) - L2*d*ddx_des*lambda1*lambda3*m^2*mu_s^3*cos(gamma2)*cos(theta) - L1*d*ddy_des*lambda2*lambda3*m^2*mu_s^2*cos(gamma1)*cos(theta) - 3*L2*d*ddy_des*lambda2*lambda3*m^2*mu_s^2*cos(gamma2)*cos(theta) - L1*d*g*lambda2*lambda3*m^2*mu_s^2*cos(gamma1)*cos(theta) - 3*L2*d*g*lambda2*lambda3*m^2*mu_s^2*cos(gamma2)*cos(theta) + L1*d*ddx_des*lambda1*lambda3*m^2*mu_s^2*cos(gamma1)*sin(theta) - L1*d*ddx_des*lambda1*lambda3*m^2*mu_s^2*cos(theta)*sin(gamma1) - 3*L2*d*ddx_des*lambda1*lambda3*m^2*mu_s^2*cos(gamma2)*sin(theta) - L2*d*ddx_des*lambda1*lambda3*m^2*mu_s^2*cos(theta)*sin(gamma2)))/(4*I^2*lambda1*lambda2*mu_s^2 + L1^2*lambda2*lambda3*m^2*sin(gamma1)^2 + L2^2*lambda2*lambda3*m^2*sin(gamma2)^2 + L1^2*lambda2*lambda3*m^2*mu_s^2*cos(gamma1)^2 + L1^2*lambda1*lambda3*m^2*mu_s^4*cos(gamma1)^2 + L2^2*lambda2*lambda3*m^2*mu_s^2*cos(gamma2)^2 + L2^2*lambda1*lambda3*m^2*mu_s^4*cos(gamma2)^2 + L1^2*lambda1*lambda3*m^2*mu_s^2*sin(gamma1)^2 + L2^2*lambda1*lambda3*m^2*mu_s^2*sin(gamma2)^2 + 4*d^2*lambda2*lambda3*m^2*mu_s^2*cos(theta)^2 + 4*d^2*lambda1*lambda3*m^2*mu_s^2*sin(theta)^2 - 2*L1^2*lambda1*lambda3*m^2*mu_s^3*cos(gamma1)*sin(gamma1) + 2*L2^2*lambda1*lambda3*m^2*mu_s^3*cos(gamma2)*sin(gamma2) - 2*L1*L2*lambda2*lambda3*m^2*sin(gamma1)*sin(gamma2) - 2*L1^2*lambda2*lambda3*m^2*mu_s*cos(gamma1)*sin(gamma1) + 2*L2^2*lambda2*lambda3*m^2*mu_s*cos(gamma2)*sin(gamma2) - 2*L1*L2*lambda1*lambda3*m^2*mu_s^3*cos(gamma1)*sin(gamma2) + 2*L1*L2*lambda1*lambda3*m^2*mu_s^3*cos(gamma2)*sin(gamma1) + 2*L1*L2*lambda1*lambda3*m^2*mu_s^2*sin(gamma1)*sin(gamma2) - 4*L1*d*lambda2*lambda3*m^2*mu_s^2*cos(gamma1)*cos(theta) - 4*L2*d*lambda2*lambda3*m^2*mu_s^2*cos(gamma2)*cos(theta) + 4*L1*d*lambda1*lambda3*m^2*mu_s^3*cos(gamma1)*sin(theta) - 4*L2*d*lambda1*lambda3*m^2*mu_s^3*cos(gamma2)*sin(theta) - 4*L1*d*lambda1*lambda3*m^2*mu_s^2*sin(gamma1)*sin(theta) - 4*L2*d*lambda1*lambda3*m^2*mu_s^2*sin(gamma2)*sin(theta) + 2*L1*L2*lambda2*lambda3*m^2*mu_s*cos(gamma1)*sin(gamma2) - 2*L1*L2*lambda2*lambda3*m^2*mu_s*cos(gamma2)*sin(gamma1) + 4*L1*d*lambda2*lambda3*m^2*mu_s*cos(theta)*sin(gamma1) - 4*L2*d*lambda2*lambda3*m^2*mu_s*cos(theta)*sin(gamma2) + 2*L1*L2*lambda2*lambda3*m^2*mu_s^2*cos(gamma1)*cos(gamma2) - 2*L1*L2*lambda1*lambda3*m^2*mu_s^4*cos(gamma1)*cos(gamma2));
    ]);

f3 = real([                                                                                                                                                                                                                                                                                                                                                                                                                                                                                                                                                                                                                                                                                                                                                                                                                                                                                                                                                                                                                                                                                                                                                                                                                                                                                                                                                                                                                                                                                                                                                                                                                                                                                                                                                                                                                                                                                                                                                                                                                                                                                                                                                                                                                                                                                                                                                                                                                                                                                                                                                                                                                                                                                                                                                                                                                                                                                                                                                                                                                                                                                                                                                                                                                                                                                                                                                                                                                                                                                                                                                                                                                                                                                                                                                                                                                                                                                                                                                                                                                                                                                                                                                                                                                                                                                                                                                                                                                                                                                                                                                                                                                                                                                                                                                                                                                                                                                                                                                                                                                                                                                                                                                                                                                                                                                                                                                                                                                                                              -(I*ddtheta_des - L1*ddx_des*m*cos(gamma1) + L1*ddy_des*m*sin(gamma1) + L1*g*m*sin(gamma1) + d*ddx_des*m*cos(theta) - d*ddy_des*m*sin(theta) - d*g*m*sin(theta))/(L1*cos(gamma1) - L2*cos(gamma2));
    -(I*ddtheta_des - L1*ddx_des*m*cos(gamma1) + L2*ddy_des*m*sin(gamma2) + L2*g*m*sin(gamma2) + d*ddx_des*m*cos(theta) - d*ddy_des*m*sin(theta) - d*g*m*sin(theta))/(L1*cos(gamma1) - L2*cos(gamma2));
    0;
    (I^2*ddx_des*lambda1*lambda2*m + L2^2*ddx_des*lambda1*lambda3*m^3*sin(gamma2)^2 + d^2*ddx_des*lambda1*lambda3*m^3*sin(theta)^2 + L2^2*ddy_des*lambda2*lambda3*m^3*cos(gamma2)*sin(gamma2) + L2^2*g*lambda2*lambda3*m^3*cos(gamma2)*sin(gamma2) + I*L2*ddtheta_des*lambda2*lambda3*m^2*cos(gamma2) + d^2*ddy_des*lambda2*lambda3*m^3*cos(theta)*sin(theta) - I*d*ddtheta_des*lambda2*lambda3*m^2*cos(theta) + d^2*g*lambda2*lambda3*m^3*cos(theta)*sin(theta) - L2*d*ddy_des*lambda2*lambda3*m^3*cos(gamma2)*sin(theta) - L2*d*ddy_des*lambda2*lambda3*m^3*cos(theta)*sin(gamma2) - L2*d*g*lambda2*lambda3*m^3*cos(gamma2)*sin(theta) - L2*d*g*lambda2*lambda3*m^3*cos(theta)*sin(gamma2) - 2*L2*d*ddx_des*lambda1*lambda3*m^3*sin(gamma2)*sin(theta))/(I^2*lambda1*lambda2 + d^2*lambda1*lambda3*m^2*sin(theta)^2 + L2^2*lambda2*lambda3*m^2*cos(gamma2)^2 + L2^2*lambda1*lambda3*m^2*sin(gamma2)^2 + d^2*lambda2*lambda3*m^2*cos(theta)^2 - 2*L2*d*lambda2*lambda3*m^2*cos(gamma2)*cos(theta) - 2*L2*d*lambda1*lambda3*m^2*sin(gamma2)*sin(theta));
    0;
    0;
    0;
    0;
    -(I*ddtheta_des - L1*ddx_des*m*cos(gamma1) + L1*ddy_des*m*sin(gamma1) + L1*g*m*sin(gamma1) + d*ddx_des*m*cos(theta) - d*ddy_des*m*sin(theta) - d*g*m*sin(theta))/(L1*cos(gamma1) - L2*cos(gamma2));
    0;
    0;
    (I^2*ddx_des*lambda1*lambda2*m + L2^2*ddx_des*lambda1*lambda3*m^3*sin(gamma2)^2 + d^2*ddx_des*lambda1*lambda3*m^3*sin(theta)^2 + L2^2*ddy_des*lambda2*lambda3*m^3*cos(gamma2)*sin(gamma2) + L2^2*g*lambda2*lambda3*m^3*cos(gamma2)*sin(gamma2) + I*L2*ddtheta_des*lambda2*lambda3*m^2*cos(gamma2) + d^2*ddy_des*lambda2*lambda3*m^3*cos(theta)*sin(theta) - I*d*ddtheta_des*lambda2*lambda3*m^2*cos(theta) + d^2*g*lambda2*lambda3*m^3*cos(theta)*sin(theta) - L2*d*ddy_des*lambda2*lambda3*m^3*cos(gamma2)*sin(theta) - L2*d*ddy_des*lambda2*lambda3*m^3*cos(theta)*sin(gamma2) - L2*d*g*lambda2*lambda3*m^3*cos(gamma2)*sin(theta) - L2*d*g*lambda2*lambda3*m^3*cos(theta)*sin(gamma2) - 2*L2*d*ddx_des*lambda1*lambda3*m^3*sin(gamma2)*sin(theta))/(I^2*lambda1*lambda2 + d^2*lambda1*lambda3*m^2*sin(theta)^2 + L2^2*lambda2*lambda3*m^2*cos(gamma2)^2 + L2^2*lambda1*lambda3*m^2*sin(gamma2)^2 + d^2*lambda2*lambda3*m^2*cos(theta)^2 - 2*L2*d*lambda2*lambda3*m^2*cos(gamma2)*cos(theta) - 2*L2*d*lambda1*lambda3*m^2*sin(gamma2)*sin(theta));
    0;
    0;
    0;
    0;
    -(mu_s*(I*ddtheta_des - L1*ddx_des*m*cos(gamma1) + L1*ddy_des*m*sin(gamma1) + L1*g*m*sin(gamma1) + d*ddx_des*m*cos(theta) - d*ddy_des*m*sin(theta) - d*g*m*sin(theta)))/(L1*sin(gamma1) - L2*sin(gamma2) + L1*mu_s*cos(gamma1) - L2*mu_s*cos(gamma2));
    (mu_s*(I*ddtheta_des - L1*ddx_des*m*cos(gamma1) + L1*ddy_des*m*sin(gamma1) + L1*g*m*sin(gamma1) + d*ddx_des*m*cos(theta) - d*ddy_des*m*sin(theta) - d*g*m*sin(theta)))/(L1*sin(gamma1) - L2*sin(gamma2) - L1*mu_s*cos(gamma1) + L2*mu_s*cos(gamma2));
    -(I*ddtheta_des*mu_s - L1*ddx_des*m*sin(gamma1) + L2*ddx_des*m*sin(gamma2) - L1*ddx_des*m*mu_s*cos(gamma1) + L2*ddy_des*m*mu_s*sin(gamma2) + L2*g*m*mu_s*sin(gamma2) + d*ddx_des*m*mu_s*cos(theta) - d*ddy_des*m*mu_s*sin(theta) - d*g*m*mu_s*sin(theta))/(L1*sin(gamma1) - L2*sin(gamma2) + L1*mu_s*cos(gamma1) - L2*mu_s*cos(gamma2));
    (I*ddtheta_des*mu_s + L1*ddx_des*m*sin(gamma1) - L2*ddx_des*m*sin(gamma2) - L1*ddx_des*m*mu_s*cos(gamma1) + L2*ddy_des*m*mu_s*sin(gamma2) + L2*g*m*mu_s*sin(gamma2) + d*ddx_des*m*mu_s*cos(theta) - d*ddy_des*m*mu_s*sin(theta) - d*g*m*mu_s*sin(theta))/(L1*sin(gamma1) - L2*sin(gamma2) - L1*mu_s*cos(gamma1) + L2*mu_s*cos(gamma2));
    (I^2*ddx_des*lambda1*lambda2*m - I^2*ddy_des*lambda1*lambda2*m*mu_s - I^2*g*lambda1*lambda2*m*mu_s + L1^2*ddx_des*lambda1*lambda3*m^3*sin(gamma1)^2 + d^2*ddx_des*lambda1*lambda3*m^3*sin(theta)^2 + L1^2*ddx_des*lambda1*lambda3*m^3*mu_s^2*cos(gamma1)^2 + I*L2*ddtheta_des*lambda2*lambda3*m^2*cos(gamma2) - d^2*ddy_des*lambda2*lambda3*m^3*mu_s*cos(theta)^2 - d^2*g*lambda2*lambda3*m^3*mu_s*cos(theta)^2 + d^2*ddy_des*lambda2*lambda3*m^3*cos(theta)*sin(theta) - I*d*ddtheta_des*lambda2*lambda3*m^2*cos(theta) + d^2*g*lambda2*lambda3*m^3*cos(theta)*sin(theta) - 2*L1^2*ddx_des*lambda1*lambda3*m^3*mu_s*cos(gamma1)*sin(gamma1) + I*L1*ddtheta_des*lambda1*lambda3*m^2*mu_s*sin(gamma1) - d^2*ddx_des*lambda1*lambda3*m^3*mu_s*cos(theta)*sin(theta) - I*d*ddtheta_des*lambda1*lambda3*m^2*mu_s*sin(theta) - I*L1*ddtheta_des*lambda1*lambda3*m^2*mu_s^2*cos(gamma1) + I*L2*ddtheta_des*lambda1*lambda3*m^2*mu_s^2*cos(gamma2) + L1*L2*ddy_des*lambda2*lambda3*m^3*cos(gamma2)*sin(gamma1) + L1*L2*g*lambda2*lambda3*m^3*cos(gamma2)*sin(gamma1) - L1*d*ddy_des*lambda2*lambda3*m^3*cos(theta)*sin(gamma1) - L2*d*ddy_des*lambda2*lambda3*m^3*cos(gamma2)*sin(theta) - L1*d*g*lambda2*lambda3*m^3*cos(theta)*sin(gamma1) - L2*d*g*lambda2*lambda3*m^3*cos(gamma2)*sin(theta) - 2*L1*d*ddx_des*lambda1*lambda3*m^3*sin(gamma1)*sin(theta) - L1*L2*ddy_des*lambda2*lambda3*m^3*mu_s*cos(gamma1)*cos(gamma2) - L1*L2*g*lambda2*lambda3*m^3*mu_s*cos(gamma1)*cos(gamma2) + L1*L2*ddx_des*lambda1*lambda3*m^3*mu_s*cos(gamma2)*sin(gamma1) + L1*d*ddy_des*lambda2*lambda3*m^3*mu_s*cos(gamma1)*cos(theta) + L2*d*ddy_des*lambda2*lambda3*m^3*mu_s*cos(gamma2)*cos(theta) + L1*d*g*lambda2*lambda3*m^3*mu_s*cos(gamma1)*cos(theta) + L2*d*g*lambda2*lambda3*m^3*mu_s*cos(gamma2)*cos(theta) + 2*L1*d*ddx_des*lambda1*lambda3*m^3*mu_s*cos(gamma1)*sin(theta) + L1*d*ddx_des*lambda1*lambda3*m^3*mu_s*cos(theta)*sin(gamma1) - L2*d*ddx_des*lambda1*lambda3*m^3*mu_s*cos(gamma2)*sin(theta) - L1*L2*ddx_des*lambda1*lambda3*m^3*mu_s^2*cos(gamma1)*cos(gamma2) - L1*d*ddx_des*lambda1*lambda3*m^3*mu_s^2*cos(gamma1)*cos(theta) + L2*d*ddx_des*lambda1*lambda3*m^3*mu_s^2*cos(gamma2)*cos(theta))/(I^2*lambda1*lambda2 + d^2*lambda1*lambda3*m^2*sin(theta)^2 + L2^2*lambda2*lambda3*m^2*cos(gamma2)^2 + L1^2*lambda1*lambda3*m^2*sin(gamma1)^2 + d^2*lambda2*lambda3*m^2*cos(theta)^2 + L1^2*lambda1*lambda3*m^2*mu_s^2*cos(gamma1)^2 + L2^2*lambda1*lambda3*m^2*mu_s^2*cos(gamma2)^2 - 2*L2*d*lambda2*lambda3*m^2*cos(gamma2)*cos(theta) - 2*L1*d*lambda1*lambda3*m^2*sin(gamma1)*sin(theta) - 2*L1^2*lambda1*lambda3*m^2*mu_s*cos(gamma1)*sin(gamma1) + 2*L1*L2*lambda1*lambda3*m^2*mu_s*cos(gamma2)*sin(gamma1) + 2*L1*d*lambda1*lambda3*m^2*mu_s*cos(gamma1)*sin(theta) - 2*L2*d*lambda1*lambda3*m^2*mu_s*cos(gamma2)*sin(theta) - 2*L1*L2*lambda1*lambda3*m^2*mu_s^2*cos(gamma1)*cos(gamma2));
    0;
    0;
    0;
    (I*m*mu_s*(I*ddy_des*lambda2 + I*g*lambda2 + I*ddx_des*lambda1*mu_s - L2*ddtheta_des*lambda3*m*sin(gamma2) + d*ddtheta_des*lambda3*m*sin(theta) + L2*ddtheta_des*lambda3*m*mu_s*cos(gamma2) - d*ddtheta_des*lambda3*m*mu_s*cos(theta)))/(I^2*lambda2 + I^2*lambda1*mu_s^2 + L2^2*lambda3*m^2*sin(gamma2)^2 + d^2*lambda3*m^2*sin(theta)^2 + L2^2*lambda3*m^2*mu_s^2*cos(gamma2)^2 + d^2*lambda3*m^2*mu_s^2*cos(theta)^2 - 2*L2*d*lambda3*m^2*sin(gamma2)*sin(theta) - 2*L2^2*lambda3*m^2*mu_s*cos(gamma2)*sin(gamma2) - 2*d^2*lambda3*m^2*mu_s*cos(theta)*sin(theta) + 2*L2*d*lambda3*m^2*mu_s*cos(gamma2)*sin(theta) + 2*L2*d*lambda3*m^2*mu_s*cos(theta)*sin(gamma2) - 2*L2*d*lambda3*m^2*mu_s^2*cos(gamma2)*cos(theta));
    -(I*m*mu_s*(I*ddy_des*lambda2 + I*g*lambda2 - I*ddx_des*lambda1*mu_s - L2*ddtheta_des*lambda3*m*sin(gamma2) + d*ddtheta_des*lambda3*m*sin(theta) - L2*ddtheta_des*lambda3*m*mu_s*cos(gamma2) + d*ddtheta_des*lambda3*m*mu_s*cos(theta)))/(I^2*lambda2 + I^2*lambda1*mu_s^2 + L2^2*lambda3*m^2*sin(gamma2)^2 + d^2*lambda3*m^2*sin(theta)^2 + L2^2*lambda3*m^2*mu_s^2*cos(gamma2)^2 + d^2*lambda3*m^2*mu_s^2*cos(theta)^2 - 2*L2*d*lambda3*m^2*sin(gamma2)*sin(theta) + 2*L2^2*lambda3*m^2*mu_s*cos(gamma2)*sin(gamma2) + 2*d^2*lambda3*m^2*mu_s*cos(theta)*sin(theta) - 2*L2*d*lambda3*m^2*mu_s*cos(gamma2)*sin(theta) - 2*L2*d*lambda3*m^2*mu_s*cos(theta)*sin(gamma2) - 2*L2*d*lambda3*m^2*mu_s^2*cos(gamma2)*cos(theta));
    0;
    -(mu_s*(I*ddtheta_des*lambda2 + I*ddtheta_des*lambda1*mu_s^2 + L1*ddy_des*lambda2*m*sin(gamma1) + L1*g*lambda2*m*sin(gamma1) - d*ddy_des*lambda2*m*sin(theta) - d*g*lambda2*m*sin(theta) + L1*ddy_des*lambda2*m*mu_s*cos(gamma1) + L1*g*lambda2*m*mu_s*cos(gamma1) - L1*ddx_des*lambda1*m*mu_s*sin(gamma1) - d*ddy_des*lambda2*m*mu_s*cos(theta) - d*g*lambda2*m*mu_s*cos(theta) + d*ddx_des*lambda1*m*mu_s*sin(theta) - L1*ddx_des*lambda1*m*mu_s^2*cos(gamma1) + d*ddx_des*lambda1*m*mu_s^2*cos(theta)))/((lambda1*mu_s^2 + lambda2)*(L1*sin(gamma1) - L2*sin(gamma2) + L1*mu_s*cos(gamma1) - L2*mu_s*cos(gamma2)));
    (mu_s*(I*ddtheta_des*lambda2 + I*ddtheta_des*lambda1*mu_s^2 + L1*ddy_des*lambda2*m*sin(gamma1) + L1*g*lambda2*m*sin(gamma1) - d*ddy_des*lambda2*m*sin(theta) - d*g*lambda2*m*sin(theta) - L1*ddy_des*lambda2*m*mu_s*cos(gamma1) - L1*g*lambda2*m*mu_s*cos(gamma1) + L1*ddx_des*lambda1*m*mu_s*sin(gamma1) + d*ddy_des*lambda2*m*mu_s*cos(theta) + d*g*lambda2*m*mu_s*cos(theta) - d*ddx_des*lambda1*m*mu_s*sin(theta) - L1*ddx_des*lambda1*m*mu_s^2*cos(gamma1) + d*ddx_des*lambda1*m*mu_s^2*cos(theta)))/((lambda1*mu_s^2 + lambda2)*(L1*sin(gamma1) - L2*sin(gamma2) - L1*mu_s*cos(gamma1) + L2*mu_s*cos(gamma2)));
    (I^2*ddx_des*lambda1*lambda2*m + I^2*ddy_des*lambda1*lambda2*m*mu_s + I^2*g*lambda1*lambda2*m*mu_s + L1^2*ddx_des*lambda1*lambda3*m^3*sin(gamma1)^2 + d^2*ddx_des*lambda1*lambda3*m^3*sin(theta)^2 + L1^2*ddx_des*lambda1*lambda3*m^3*mu_s^2*cos(gamma1)^2 + I*L2*ddtheta_des*lambda2*lambda3*m^2*cos(gamma2) + d^2*ddy_des*lambda2*lambda3*m^3*mu_s*cos(theta)^2 + d^2*g*lambda2*lambda3*m^3*mu_s*cos(theta)^2 + d^2*ddy_des*lambda2*lambda3*m^3*cos(theta)*sin(theta) - I*d*ddtheta_des*lambda2*lambda3*m^2*cos(theta) + d^2*g*lambda2*lambda3*m^3*cos(theta)*sin(theta) + 2*L1^2*ddx_des*lambda1*lambda3*m^3*mu_s*cos(gamma1)*sin(gamma1) - I*L1*ddtheta_des*lambda1*lambda3*m^2*mu_s*sin(gamma1) + d^2*ddx_des*lambda1*lambda3*m^3*mu_s*cos(theta)*sin(theta) + I*d*ddtheta_des*lambda1*lambda3*m^2*mu_s*sin(theta) - I*L1*ddtheta_des*lambda1*lambda3*m^2*mu_s^2*cos(gamma1) + I*L2*ddtheta_des*lambda1*lambda3*m^2*mu_s^2*cos(gamma2) + L1*L2*ddy_des*lambda2*lambda3*m^3*cos(gamma2)*sin(gamma1) + L1*L2*g*lambda2*lambda3*m^3*cos(gamma2)*sin(gamma1) - L1*d*ddy_des*lambda2*lambda3*m^3*cos(theta)*sin(gamma1) - L2*d*ddy_des*lambda2*lambda3*m^3*cos(gamma2)*sin(theta) - L1*d*g*lambda2*lambda3*m^3*cos(theta)*sin(gamma1) - L2*d*g*lambda2*lambda3*m^3*cos(gamma2)*sin(theta) - 2*L1*d*ddx_des*lambda1*lambda3*m^3*sin(gamma1)*sin(theta) + L1*L2*ddy_des*lambda2*lambda3*m^3*mu_s*cos(gamma1)*cos(gamma2) + L1*L2*g*lambda2*lambda3*m^3*mu_s*cos(gamma1)*cos(gamma2) - L1*L2*ddx_des*lambda1*lambda3*m^3*mu_s*cos(gamma2)*sin(gamma1) - L1*d*ddy_des*lambda2*lambda3*m^3*mu_s*cos(gamma1)*cos(theta) - L2*d*ddy_des*lambda2*lambda3*m^3*mu_s*cos(gamma2)*cos(theta) - L1*d*g*lambda2*lambda3*m^3*mu_s*cos(gamma1)*cos(theta) - L2*d*g*lambda2*lambda3*m^3*mu_s*cos(gamma2)*cos(theta) - 2*L1*d*ddx_des*lambda1*lambda3*m^3*mu_s*cos(gamma1)*sin(theta) - L1*d*ddx_des*lambda1*lambda3*m^3*mu_s*cos(theta)*sin(gamma1) + L2*d*ddx_des*lambda1*lambda3*m^3*mu_s*cos(gamma2)*sin(theta) - L1*L2*ddx_des*lambda1*lambda3*m^3*mu_s^2*cos(gamma1)*cos(gamma2) - L1*d*ddx_des*lambda1*lambda3*m^3*mu_s^2*cos(gamma1)*cos(theta) + L2*d*ddx_des*lambda1*lambda3*m^3*mu_s^2*cos(gamma2)*cos(theta))/(I^2*lambda1*lambda2 + d^2*lambda1*lambda3*m^2*sin(theta)^2 + L2^2*lambda2*lambda3*m^2*cos(gamma2)^2 + L1^2*lambda1*lambda3*m^2*sin(gamma1)^2 + d^2*lambda2*lambda3*m^2*cos(theta)^2 + L1^2*lambda1*lambda3*m^2*mu_s^2*cos(gamma1)^2 + L2^2*lambda1*lambda3*m^2*mu_s^2*cos(gamma2)^2 - 2*L2*d*lambda2*lambda3*m^2*cos(gamma2)*cos(theta) - 2*L1*d*lambda1*lambda3*m^2*sin(gamma1)*sin(theta) + 2*L1^2*lambda1*lambda3*m^2*mu_s*cos(gamma1)*sin(gamma1) - 2*L1*L2*lambda1*lambda3*m^2*mu_s*cos(gamma2)*sin(gamma1) - 2*L1*d*lambda1*lambda3*m^2*mu_s*cos(gamma1)*sin(theta) + 2*L2*d*lambda1*lambda3*m^2*mu_s*cos(gamma2)*sin(theta) - 2*L1*L2*lambda1*lambda3*m^2*mu_s^2*cos(gamma1)*cos(gamma2));
    (m*mu_s*(I^2*ddy_des*lambda1*lambda2 + I^2*g*lambda1*lambda2 + L1^2*ddy_des*lambda2*lambda3*m^2*cos(gamma1)^2 + L1^2*g*lambda2*lambda3*m^2*cos(gamma1)^2 + d^2*ddy_des*lambda2*lambda3*m^2*cos(theta)^2 + d^2*g*lambda2*lambda3*m^2*cos(theta)^2 - I*L2*ddtheta_des*lambda1*lambda3*m*sin(gamma2) + I*d*ddtheta_des*lambda1*lambda3*m*sin(theta) + L1^2*ddx_des*lambda1*lambda3*m^2*mu_s*cos(gamma1)^2 + d^2*ddx_des*lambda1*lambda3*m^2*cos(theta)*sin(theta) + L1*L2*ddx_des*lambda1*lambda3*m^2*cos(gamma1)*sin(gamma2) - 2*L1*d*ddy_des*lambda2*lambda3*m^2*cos(gamma1)*cos(theta) - 2*L1*d*g*lambda2*lambda3*m^2*cos(gamma1)*cos(theta) - L1*d*ddx_des*lambda1*lambda3*m^2*cos(gamma1)*sin(theta) - L2*d*ddx_des*lambda1*lambda3*m^2*cos(theta)*sin(gamma2) - I*L1*ddtheta_des*lambda1*lambda3*m*mu_s*cos(gamma1) + I*L2*ddtheta_des*lambda1*lambda3*m*mu_s*cos(gamma2) - L1*L2*ddx_des*lambda1*lambda3*m^2*mu_s*cos(gamma1)*cos(gamma2) - L1*d*ddx_des*lambda1*lambda3*m^2*mu_s*cos(gamma1)*cos(theta) + L2*d*ddx_des*lambda1*lambda3*m^2*mu_s*cos(gamma2)*cos(theta)))/(I^2*lambda1*lambda2 + d^2*lambda1*lambda3*m^2*sin(theta)^2 + L1^2*lambda2*lambda3*m^2*cos(gamma1)^2 + L2^2*lambda1*lambda3*m^2*sin(gamma2)^2 + d^2*lambda2*lambda3*m^2*cos(theta)^2 + L1^2*lambda1*lambda3*m^2*mu_s^2*cos(gamma1)^2 + L2^2*lambda1*lambda3*m^2*mu_s^2*cos(gamma2)^2 - 2*L1*d*lambda2*lambda3*m^2*cos(gamma1)*cos(theta) - 2*L2*d*lambda1*lambda3*m^2*sin(gamma2)*sin(theta) - 2*L2^2*lambda1*lambda3*m^2*mu_s*cos(gamma2)*sin(gamma2) + 2*L1*L2*lambda1*lambda3*m^2*mu_s*cos(gamma1)*sin(gamma2) - 2*L1*d*lambda1*lambda3*m^2*mu_s*cos(gamma1)*sin(theta) + 2*L2*d*lambda1*lambda3*m^2*mu_s*cos(gamma2)*sin(theta) - 2*L1*L2*lambda1*lambda3*m^2*mu_s^2*cos(gamma1)*cos(gamma2));
    -(m*mu_s*(I^2*ddy_des*lambda1*lambda2 + I^2*g*lambda1*lambda2 + L1^2*ddy_des*lambda2*lambda3*m^2*cos(gamma1)^2 + L1^2*g*lambda2*lambda3*m^2*cos(gamma1)^2 + d^2*ddy_des*lambda2*lambda3*m^2*cos(theta)^2 + d^2*g*lambda2*lambda3*m^2*cos(theta)^2 - I*L2*ddtheta_des*lambda1*lambda3*m*sin(gamma2) + I*d*ddtheta_des*lambda1*lambda3*m*sin(theta) - L1^2*ddx_des*lambda1*lambda3*m^2*mu_s*cos(gamma1)^2 + d^2*ddx_des*lambda1*lambda3*m^2*cos(theta)*sin(theta) + L1*L2*ddx_des*lambda1*lambda3*m^2*cos(gamma1)*sin(gamma2) - 2*L1*d*ddy_des*lambda2*lambda3*m^2*cos(gamma1)*cos(theta) - 2*L1*d*g*lambda2*lambda3*m^2*cos(gamma1)*cos(theta) - L1*d*ddx_des*lambda1*lambda3*m^2*cos(gamma1)*sin(theta) - L2*d*ddx_des*lambda1*lambda3*m^2*cos(theta)*sin(gamma2) + I*L1*ddtheta_des*lambda1*lambda3*m*mu_s*cos(gamma1) - I*L2*ddtheta_des*lambda1*lambda3*m*mu_s*cos(gamma2) + L1*L2*ddx_des*lambda1*lambda3*m^2*mu_s*cos(gamma1)*cos(gamma2) + L1*d*ddx_des*lambda1*lambda3*m^2*mu_s*cos(gamma1)*cos(theta) - L2*d*ddx_des*lambda1*lambda3*m^2*mu_s*cos(gamma2)*cos(theta)))/(I^2*lambda1*lambda2 + d^2*lambda1*lambda3*m^2*sin(theta)^2 + L1^2*lambda2*lambda3*m^2*cos(gamma1)^2 + L2^2*lambda1*lambda3*m^2*sin(gamma2)^2 + d^2*lambda2*lambda3*m^2*cos(theta)^2 + L1^2*lambda1*lambda3*m^2*mu_s^2*cos(gamma1)^2 + L2^2*lambda1*lambda3*m^2*mu_s^2*cos(gamma2)^2 - 2*L1*d*lambda2*lambda3*m^2*cos(gamma1)*cos(theta) - 2*L2*d*lambda1*lambda3*m^2*sin(gamma2)*sin(theta) + 2*L2^2*lambda1*lambda3*m^2*mu_s*cos(gamma2)*sin(gamma2) - 2*L1*L2*lambda1*lambda3*m^2*mu_s*cos(gamma1)*sin(gamma2) + 2*L1*d*lambda1*lambda3*m^2*mu_s*cos(gamma1)*sin(theta) - 2*L2*d*lambda1*lambda3*m^2*mu_s*cos(gamma2)*sin(theta) - 2*L1*L2*lambda1*lambda3*m^2*mu_s^2*cos(gamma1)*cos(gamma2));
    0;
    0;
    0;
    (I^2*ddx_des*lambda1*lambda2*m + L2^2*ddx_des*lambda1*lambda3*m^3*sin(gamma2)^2 + d^2*ddx_des*lambda1*lambda3*m^3*sin(theta)^2 + L2^2*ddy_des*lambda2*lambda3*m^3*cos(gamma2)*sin(gamma2) + L2^2*g*lambda2*lambda3*m^3*cos(gamma2)*sin(gamma2) + I*L2*ddtheta_des*lambda2*lambda3*m^2*cos(gamma2) + d^2*ddy_des*lambda2*lambda3*m^3*cos(theta)*sin(theta) - I*d*ddtheta_des*lambda2*lambda3*m^2*cos(theta) + d^2*g*lambda2*lambda3*m^3*cos(theta)*sin(theta) - L2*d*ddy_des*lambda2*lambda3*m^3*cos(gamma2)*sin(theta) - L2*d*ddy_des*lambda2*lambda3*m^3*cos(theta)*sin(gamma2) - L2*d*g*lambda2*lambda3*m^3*cos(gamma2)*sin(theta) - L2*d*g*lambda2*lambda3*m^3*cos(theta)*sin(gamma2) - 2*L2*d*ddx_des*lambda1*lambda3*m^3*sin(gamma2)*sin(theta))/(I^2*lambda1*lambda2 + d^2*lambda1*lambda3*m^2*sin(theta)^2 + L2^2*lambda2*lambda3*m^2*cos(gamma2)^2 + L2^2*lambda1*lambda3*m^2*sin(gamma2)^2 + d^2*lambda2*lambda3*m^2*cos(theta)^2 - 2*L2*d*lambda2*lambda3*m^2*cos(gamma2)*cos(theta) - 2*L2*d*lambda1*lambda3*m^2*sin(gamma2)*sin(theta));
    (I^2*ddx_des*lambda1*lambda2*m + L2^2*ddx_des*lambda1*lambda3*m^3*sin(gamma2)^2 + d^2*ddx_des*lambda1*lambda3*m^3*sin(theta)^2 + L2^2*ddy_des*lambda2*lambda3*m^3*cos(gamma2)*sin(gamma2) + L2^2*g*lambda2*lambda3*m^3*cos(gamma2)*sin(gamma2) + I*L2*ddtheta_des*lambda2*lambda3*m^2*cos(gamma2) + d^2*ddy_des*lambda2*lambda3*m^3*cos(theta)*sin(theta) - I*d*ddtheta_des*lambda2*lambda3*m^2*cos(theta) + d^2*g*lambda2*lambda3*m^3*cos(theta)*sin(theta) - L2*d*ddy_des*lambda2*lambda3*m^3*cos(gamma2)*sin(theta) - L2*d*ddy_des*lambda2*lambda3*m^3*cos(theta)*sin(gamma2) - L2*d*g*lambda2*lambda3*m^3*cos(gamma2)*sin(theta) - L2*d*g*lambda2*lambda3*m^3*cos(theta)*sin(gamma2) - 2*L2*d*ddx_des*lambda1*lambda3*m^3*sin(gamma2)*sin(theta))/(I^2*lambda1*lambda2 + d^2*lambda1*lambda3*m^2*sin(theta)^2 + L2^2*lambda2*lambda3*m^2*cos(gamma2)^2 + L2^2*lambda1*lambda3*m^2*sin(gamma2)^2 + d^2*lambda2*lambda3*m^2*cos(theta)^2 - 2*L2*d*lambda2*lambda3*m^2*cos(gamma2)*cos(theta) - 2*L2*d*lambda1*lambda3*m^2*sin(gamma2)*sin(theta));
    -(I*ddtheta_des - L1*ddx_des*m*cos(gamma1) + d*ddx_des*m*cos(theta))/(L1*cos(gamma1) - L2*cos(gamma2));
    0;
    0;
    0;
    0;
    0;
    0;
    (I*m*(I*ddx_des*lambda1 + L2*ddtheta_des*lambda3*m*cos(gamma2) - d*ddtheta_des*lambda3*m*cos(theta)))/(I^2*lambda1 + L2^2*lambda3*m^2*cos(gamma2)^2 + d^2*lambda3*m^2*cos(theta)^2 - 2*L2*d*lambda3*m^2*cos(gamma2)*cos(theta));
    0;
    0;
    (I*m*(I*ddx_des*lambda1 + L2*ddtheta_des*lambda3*m*cos(gamma2) - d*ddtheta_des*lambda3*m*cos(theta)))/(I^2*lambda1 + L2^2*lambda3*m^2*cos(gamma2)^2 + d^2*lambda3*m^2*cos(theta)^2 - 2*L2*d*lambda3*m^2*cos(gamma2)*cos(theta));
    0;
    0;
    (I*m*mu_s*(I*ddy_des*lambda2 + I*g*lambda2 + I*ddx_des*lambda1*mu_s - L2*ddtheta_des*lambda3*m*sin(gamma2) + d*ddtheta_des*lambda3*m*sin(theta) + L2*ddtheta_des*lambda3*m*mu_s*cos(gamma2) - d*ddtheta_des*lambda3*m*mu_s*cos(theta)))/(I^2*lambda2 + I^2*lambda1*mu_s^2 + L2^2*lambda3*m^2*sin(gamma2)^2 + d^2*lambda3*m^2*sin(theta)^2 + L2^2*lambda3*m^2*mu_s^2*cos(gamma2)^2 + d^2*lambda3*m^2*mu_s^2*cos(theta)^2 - 2*L2*d*lambda3*m^2*sin(gamma2)*sin(theta) - 2*L2^2*lambda3*m^2*mu_s*cos(gamma2)*sin(gamma2) - 2*d^2*lambda3*m^2*mu_s*cos(theta)*sin(theta) + 2*L2*d*lambda3*m^2*mu_s*cos(gamma2)*sin(theta) + 2*L2*d*lambda3*m^2*mu_s*cos(theta)*sin(gamma2) - 2*L2*d*lambda3*m^2*mu_s^2*cos(gamma2)*cos(theta));
    -(I*m*mu_s*(I*ddy_des*lambda2 + I*g*lambda2 - I*ddx_des*lambda1*mu_s - L2*ddtheta_des*lambda3*m*sin(gamma2) + d*ddtheta_des*lambda3*m*sin(theta) - L2*ddtheta_des*lambda3*m*mu_s*cos(gamma2) + d*ddtheta_des*lambda3*m*mu_s*cos(theta)))/(I^2*lambda2 + I^2*lambda1*mu_s^2 + L2^2*lambda3*m^2*sin(gamma2)^2 + d^2*lambda3*m^2*sin(theta)^2 + L2^2*lambda3*m^2*mu_s^2*cos(gamma2)^2 + d^2*lambda3*m^2*mu_s^2*cos(theta)^2 - 2*L2*d*lambda3*m^2*sin(gamma2)*sin(theta) + 2*L2^2*lambda3*m^2*mu_s*cos(gamma2)*sin(gamma2) + 2*d^2*lambda3*m^2*mu_s*cos(theta)*sin(theta) - 2*L2*d*lambda3*m^2*mu_s*cos(gamma2)*sin(theta) - 2*L2*d*lambda3*m^2*mu_s*cos(theta)*sin(gamma2) - 2*L2*d*lambda3*m^2*mu_s^2*cos(gamma2)*cos(theta));
    (I*m*(I*ddx_des*lambda1 + L2*ddtheta_des*lambda3*m*cos(gamma2) - d*ddtheta_des*lambda3*m*cos(theta)))/(I^2*lambda1 + L2^2*lambda3*m^2*cos(gamma2)^2 + d^2*lambda3*m^2*cos(theta)^2 - 2*L2*d*lambda3*m^2*cos(gamma2)*cos(theta));
    (I*m*(I*ddx_des*lambda1 + L2*ddtheta_des*lambda3*m*cos(gamma2) - d*ddtheta_des*lambda3*m*cos(theta)))/(I^2*lambda1 + L2^2*lambda3*m^2*cos(gamma2)^2 + d^2*lambda3*m^2*cos(theta)^2 - 2*L2*d*lambda3*m^2*cos(gamma2)*cos(theta));
    0;
    0;
    -(I*m*mu_s*(I*ddy_des*lambda2 + I*g*lambda2 - I*ddx_des*lambda1*mu_s - L2*ddtheta_des*lambda3*m*sin(gamma2) + d*ddtheta_des*lambda3*m*sin(theta) - L2*ddtheta_des*lambda3*m*mu_s*cos(gamma2) + d*ddtheta_des*lambda3*m*mu_s*cos(theta)))/(I^2*lambda2 + I^2*lambda1*mu_s^2 + L2^2*lambda3*m^2*sin(gamma2)^2 + d^2*lambda3*m^2*sin(theta)^2 + L2^2*lambda3*m^2*mu_s^2*cos(gamma2)^2 + d^2*lambda3*m^2*mu_s^2*cos(theta)^2 - 2*L2*d*lambda3*m^2*sin(gamma2)*sin(theta) + 2*L2^2*lambda3*m^2*mu_s*cos(gamma2)*sin(gamma2) + 2*d^2*lambda3*m^2*mu_s*cos(theta)*sin(theta) - 2*L2*d*lambda3*m^2*mu_s*cos(gamma2)*sin(theta) - 2*L2*d*lambda3*m^2*mu_s*cos(theta)*sin(gamma2) - 2*L2*d*lambda3*m^2*mu_s^2*cos(gamma2)*cos(theta));
    (I*m*mu_s*(I*ddy_des*lambda2 + I*g*lambda2 + I*ddx_des*lambda1*mu_s - L2*ddtheta_des*lambda3*m*sin(gamma2) + d*ddtheta_des*lambda3*m*sin(theta) + L2*ddtheta_des*lambda3*m*mu_s*cos(gamma2) - d*ddtheta_des*lambda3*m*mu_s*cos(theta)))/(I^2*lambda2 + I^2*lambda1*mu_s^2 + L2^2*lambda3*m^2*sin(gamma2)^2 + d^2*lambda3*m^2*sin(theta)^2 + L2^2*lambda3*m^2*mu_s^2*cos(gamma2)^2 + d^2*lambda3*m^2*mu_s^2*cos(theta)^2 - 2*L2*d*lambda3*m^2*sin(gamma2)*sin(theta) - 2*L2^2*lambda3*m^2*mu_s*cos(gamma2)*sin(gamma2) - 2*d^2*lambda3*m^2*mu_s*cos(theta)*sin(theta) + 2*L2*d*lambda3*m^2*mu_s*cos(gamma2)*sin(theta) + 2*L2*d*lambda3*m^2*mu_s*cos(theta)*sin(gamma2) - 2*L2*d*lambda3*m^2*mu_s^2*cos(gamma2)*cos(theta));
    0;
    0;
    (I*m*mu_s*(I*ddy_des*lambda2 + I*g*lambda2 + I*ddx_des*lambda1*mu_s - L2*ddtheta_des*lambda3*m*sin(gamma2) + d*ddtheta_des*lambda3*m*sin(theta) + L2*ddtheta_des*lambda3*m*mu_s*cos(gamma2) - d*ddtheta_des*lambda3*m*mu_s*cos(theta)))/(I^2*lambda2 + I^2*lambda1*mu_s^2 + L2^2*lambda3*m^2*sin(gamma2)^2 + d^2*lambda3*m^2*sin(theta)^2 + L2^2*lambda3*m^2*mu_s^2*cos(gamma2)^2 + d^2*lambda3*m^2*mu_s^2*cos(theta)^2 - 2*L2*d*lambda3*m^2*sin(gamma2)*sin(theta) - 2*L2^2*lambda3*m^2*mu_s*cos(gamma2)*sin(gamma2) - 2*d^2*lambda3*m^2*mu_s*cos(theta)*sin(theta) + 2*L2*d*lambda3*m^2*mu_s*cos(gamma2)*sin(theta) + 2*L2*d*lambda3*m^2*mu_s*cos(theta)*sin(gamma2) - 2*L2*d*lambda3*m^2*mu_s^2*cos(gamma2)*cos(theta));
    -(I*m*mu_s*(I*ddy_des*lambda2 + I*g*lambda2 - I*ddx_des*lambda1*mu_s - L2*ddtheta_des*lambda3*m*sin(gamma2) + d*ddtheta_des*lambda3*m*sin(theta) - L2*ddtheta_des*lambda3*m*mu_s*cos(gamma2) + d*ddtheta_des*lambda3*m*mu_s*cos(theta)))/(I^2*lambda2 + I^2*lambda1*mu_s^2 + L2^2*lambda3*m^2*sin(gamma2)^2 + d^2*lambda3*m^2*sin(theta)^2 + L2^2*lambda3*m^2*mu_s^2*cos(gamma2)^2 + d^2*lambda3*m^2*mu_s^2*cos(theta)^2 - 2*L2*d*lambda3*m^2*sin(gamma2)*sin(theta) + 2*L2^2*lambda3*m^2*mu_s*cos(gamma2)*sin(gamma2) + 2*d^2*lambda3*m^2*mu_s*cos(theta)*sin(theta) - 2*L2*d*lambda3*m^2*mu_s*cos(gamma2)*sin(theta) - 2*L2*d*lambda3*m^2*mu_s*cos(theta)*sin(gamma2) - 2*L2*d*lambda3*m^2*mu_s^2*cos(gamma2)*cos(theta));
    (mu_s*(2*I^2*ddx_des*lambda1*lambda2*m*mu_s + L1^2*ddy_des*lambda2*lambda3*m^3*sin(gamma1)^2 + L1^2*g*lambda2*lambda3*m^3*sin(gamma1)^2 + 2*I^2*ddy_des*lambda1*lambda2*m*mu_s^2 + 2*I^2*g*lambda1*lambda2*m*mu_s^2 + L1^2*ddx_des*lambda1*lambda3*m^3*mu_s^3*cos(gamma1)^2 + L1^2*ddy_des*lambda2*lambda3*m^3*mu_s^2*cos(gamma1)^2 + L1^2*g*lambda2*lambda3*m^3*mu_s^2*cos(gamma1)^2 + 2*d^2*ddy_des*lambda2*lambda3*m^3*mu_s^2*cos(theta)^2 + 2*d^2*g*lambda2*lambda3*m^3*mu_s^2*cos(theta)^2 + L1^2*ddx_des*lambda1*lambda3*m^3*mu_s*sin(gamma1)^2 + I*L1*ddtheta_des*lambda2*lambda3*m^2*sin(gamma1) - I*L2*ddtheta_des*lambda2*lambda3*m^2*sin(gamma2) + 2*d^2*ddx_des*lambda1*lambda3*m^3*mu_s*sin(theta)^2 + 2*L1^2*ddy_des*lambda2*lambda3*m^3*mu_s*cos(gamma1)*sin(gamma1) + 2*L1^2*g*lambda2*lambda3*m^3*mu_s*cos(gamma1)*sin(gamma1) + I*L1*ddtheta_des*lambda2*lambda3*m^2*mu_s*cos(gamma1) + I*L2*ddtheta_des*lambda2*lambda3*m^2*mu_s*cos(gamma2) + 2*d^2*ddy_des*lambda2*lambda3*m^3*mu_s*cos(theta)*sin(theta) - 2*I*d*ddtheta_des*lambda2*lambda3*m^2*mu_s*cos(theta) + 2*d^2*g*lambda2*lambda3*m^3*mu_s*cos(theta)*sin(theta) + 2*L1^2*ddx_des*lambda1*lambda3*m^3*mu_s^2*cos(gamma1)*sin(gamma1) - I*L1*ddtheta_des*lambda1*lambda3*m^2*mu_s^3*cos(gamma1) + I*L2*ddtheta_des*lambda1*lambda3*m^2*mu_s^3*cos(gamma2) - I*L1*ddtheta_des*lambda1*lambda3*m^2*mu_s^2*sin(gamma1) - I*L2*ddtheta_des*lambda1*lambda3*m^2*mu_s^2*sin(gamma2) - L1*L2*ddy_des*lambda2*lambda3*m^3*sin(gamma1)*sin(gamma2) + 2*d^2*ddx_des*lambda1*lambda3*m^3*mu_s^2*cos(theta)*sin(theta) - L1*L2*g*lambda2*lambda3*m^3*sin(gamma1)*sin(gamma2) + 2*I*d*ddtheta_des*lambda1*lambda3*m^2*mu_s^2*sin(theta) - L1*d*ddy_des*lambda2*lambda3*m^3*sin(gamma1)*sin(theta) + L2*d*ddy_des*lambda2*lambda3*m^3*sin(gamma2)*sin(theta) - L1*d*g*lambda2*lambda3*m^3*sin(gamma1)*sin(theta) + L2*d*g*lambda2*lambda3*m^3*sin(gamma2)*sin(theta) - L1*L2*ddy_des*lambda2*lambda3*m^3*mu_s*cos(gamma1)*sin(gamma2) + L1*L2*ddy_des*lambda2*lambda3*m^3*mu_s*cos(gamma2)*sin(gamma1) - L1*L2*g*lambda2*lambda3*m^3*mu_s*cos(gamma1)*sin(gamma2) + L1*L2*g*lambda2*lambda3*m^3*mu_s*cos(gamma2)*sin(gamma1) + L1*L2*ddx_des*lambda1*lambda3*m^3*mu_s*sin(gamma1)*sin(gamma2) - L1*d*ddy_des*lambda2*lambda3*m^3*mu_s*cos(gamma1)*sin(theta) - 3*L1*d*ddy_des*lambda2*lambda3*m^3*mu_s*cos(theta)*sin(gamma1) - L2*d*ddy_des*lambda2*lambda3*m^3*mu_s*cos(gamma2)*sin(theta) + L2*d*ddy_des*lambda2*lambda3*m^3*mu_s*cos(theta)*sin(gamma2) - L1*d*g*lambda2*lambda3*m^3*mu_s*cos(gamma1)*sin(theta) - 3*L1*d*g*lambda2*lambda3*m^3*mu_s*cos(theta)*sin(gamma1) - L2*d*g*lambda2*lambda3*m^3*mu_s*cos(gamma2)*sin(theta) + L2*d*g*lambda2*lambda3*m^3*mu_s*cos(theta)*sin(gamma2) - 3*L1*d*ddx_des*lambda1*lambda3*m^3*mu_s*sin(gamma1)*sin(theta) - L2*d*ddx_des*lambda1*lambda3*m^3*mu_s*sin(gamma2)*sin(theta) - L1*L2*ddx_des*lambda1*lambda3*m^3*mu_s^3*cos(gamma1)*cos(gamma2) + L1*L2*ddy_des*lambda2*lambda3*m^3*mu_s^2*cos(gamma1)*cos(gamma2) + L1*L2*g*lambda2*lambda3*m^3*mu_s^2*cos(gamma1)*cos(gamma2) + L1*L2*ddx_des*lambda1*lambda3*m^3*mu_s^2*cos(gamma1)*sin(gamma2) - L1*L2*ddx_des*lambda1*lambda3*m^3*mu_s^2*cos(gamma2)*sin(gamma1) - L1*d*ddx_des*lambda1*lambda3*m^3*mu_s^3*cos(gamma1)*cos(theta) + L2*d*ddx_des*lambda1*lambda3*m^3*mu_s^3*cos(gamma2)*cos(theta) - 3*L1*d*ddy_des*lambda2*lambda3*m^3*mu_s^2*cos(gamma1)*cos(theta) - L2*d*ddy_des*lambda2*lambda3*m^3*mu_s^2*cos(gamma2)*cos(theta) - 3*L1*d*g*lambda2*lambda3*m^3*mu_s^2*cos(gamma1)*cos(theta) - L2*d*g*lambda2*lambda3*m^3*mu_s^2*cos(gamma2)*cos(theta) - 3*L1*d*ddx_des*lambda1*lambda3*m^3*mu_s^2*cos(gamma1)*sin(theta) - L1*d*ddx_des*lambda1*lambda3*m^3*mu_s^2*cos(theta)*sin(gamma1) + L2*d*ddx_des*lambda1*lambda3*m^3*mu_s^2*cos(gamma2)*sin(theta) - L2*d*ddx_des*lambda1*lambda3*m^3*mu_s^2*cos(theta)*sin(gamma2)))/(4*I^2*lambda1*lambda2*mu_s^2 + L1^2*lambda2*lambda3*m^2*sin(gamma1)^2 + L2^2*lambda2*lambda3*m^2*sin(gamma2)^2 + L1^2*lambda2*lambda3*m^2*mu_s^2*cos(gamma1)^2 + L1^2*lambda1*lambda3*m^2*mu_s^4*cos(gamma1)^2 + L2^2*lambda2*lambda3*m^2*mu_s^2*cos(gamma2)^2 + L2^2*lambda1*lambda3*m^2*mu_s^4*cos(gamma2)^2 + L1^2*lambda1*lambda3*m^2*mu_s^2*sin(gamma1)^2 + L2^2*lambda1*lambda3*m^2*mu_s^2*sin(gamma2)^2 + 4*d^2*lambda2*lambda3*m^2*mu_s^2*cos(theta)^2 + 4*d^2*lambda1*lambda3*m^2*mu_s^2*sin(theta)^2 + 2*L1^2*lambda1*lambda3*m^2*mu_s^3*cos(gamma1)*sin(gamma1) - 2*L2^2*lambda1*lambda3*m^2*mu_s^3*cos(gamma2)*sin(gamma2) - 2*L1*L2*lambda2*lambda3*m^2*sin(gamma1)*sin(gamma2) + 2*L1^2*lambda2*lambda3*m^2*mu_s*cos(gamma1)*sin(gamma1) - 2*L2^2*lambda2*lambda3*m^2*mu_s*cos(gamma2)*sin(gamma2) + 2*L1*L2*lambda1*lambda3*m^2*mu_s^3*cos(gamma1)*sin(gamma2) - 2*L1*L2*lambda1*lambda3*m^2*mu_s^3*cos(gamma2)*sin(gamma1) + 2*L1*L2*lambda1*lambda3*m^2*mu_s^2*sin(gamma1)*sin(gamma2) - 4*L1*d*lambda2*lambda3*m^2*mu_s^2*cos(gamma1)*cos(theta) - 4*L2*d*lambda2*lambda3*m^2*mu_s^2*cos(gamma2)*cos(theta) - 4*L1*d*lambda1*lambda3*m^2*mu_s^3*cos(gamma1)*sin(theta) + 4*L2*d*lambda1*lambda3*m^2*mu_s^3*cos(gamma2)*sin(theta) - 4*L1*d*lambda1*lambda3*m^2*mu_s^2*sin(gamma1)*sin(theta) - 4*L2*d*lambda1*lambda3*m^2*mu_s^2*sin(gamma2)*sin(theta) - 2*L1*L2*lambda2*lambda3*m^2*mu_s*cos(gamma1)*sin(gamma2) + 2*L1*L2*lambda2*lambda3*m^2*mu_s*cos(gamma2)*sin(gamma1) - 4*L1*d*lambda2*lambda3*m^2*mu_s*cos(theta)*sin(gamma1) + 4*L2*d*lambda2*lambda3*m^2*mu_s*cos(theta)*sin(gamma2) + 2*L1*L2*lambda2*lambda3*m^2*mu_s^2*cos(gamma1)*cos(gamma2) - 2*L1*L2*lambda1*lambda3*m^2*mu_s^4*cos(gamma1)*cos(gamma2));
    (mu_s*(2*I^2*ddx_des*lambda1*lambda2*m*mu_s - L1^2*ddy_des*lambda2*lambda3*m^3*sin(gamma1)^2 - L1^2*g*lambda2*lambda3*m^3*sin(gamma1)^2 - 2*I^2*ddy_des*lambda1*lambda2*m*mu_s^2 - 2*I^2*g*lambda1*lambda2*m*mu_s^2 + L1^2*ddx_des*lambda1*lambda3*m^3*mu_s^3*cos(gamma1)^2 - L1^2*ddy_des*lambda2*lambda3*m^3*mu_s^2*cos(gamma1)^2 - L1^2*g*lambda2*lambda3*m^3*mu_s^2*cos(gamma1)^2 - 2*d^2*ddy_des*lambda2*lambda3*m^3*mu_s^2*cos(theta)^2 - 2*d^2*g*lambda2*lambda3*m^3*mu_s^2*cos(theta)^2 + L1^2*ddx_des*lambda1*lambda3*m^3*mu_s*sin(gamma1)^2 - I*L1*ddtheta_des*lambda2*lambda3*m^2*sin(gamma1) + I*L2*ddtheta_des*lambda2*lambda3*m^2*sin(gamma2) + 2*d^2*ddx_des*lambda1*lambda3*m^3*mu_s*sin(theta)^2 + 2*L1^2*ddy_des*lambda2*lambda3*m^3*mu_s*cos(gamma1)*sin(gamma1) + 2*L1^2*g*lambda2*lambda3*m^3*mu_s*cos(gamma1)*sin(gamma1) + I*L1*ddtheta_des*lambda2*lambda3*m^2*mu_s*cos(gamma1) + I*L2*ddtheta_des*lambda2*lambda3*m^2*mu_s*cos(gamma2) + 2*d^2*ddy_des*lambda2*lambda3*m^3*mu_s*cos(theta)*sin(theta) - 2*I*d*ddtheta_des*lambda2*lambda3*m^2*mu_s*cos(theta) + 2*d^2*g*lambda2*lambda3*m^3*mu_s*cos(theta)*sin(theta) - 2*L1^2*ddx_des*lambda1*lambda3*m^3*mu_s^2*cos(gamma1)*sin(gamma1) - I*L1*ddtheta_des*lambda1*lambda3*m^2*mu_s^3*cos(gamma1) + I*L2*ddtheta_des*lambda1*lambda3*m^2*mu_s^3*cos(gamma2) + I*L1*ddtheta_des*lambda1*lambda3*m^2*mu_s^2*sin(gamma1) + I*L2*ddtheta_des*lambda1*lambda3*m^2*mu_s^2*sin(gamma2) + L1*L2*ddy_des*lambda2*lambda3*m^3*sin(gamma1)*sin(gamma2) - 2*d^2*ddx_des*lambda1*lambda3*m^3*mu_s^2*cos(theta)*sin(theta) + L1*L2*g*lambda2*lambda3*m^3*sin(gamma1)*sin(gamma2) - 2*I*d*ddtheta_des*lambda1*lambda3*m^2*mu_s^2*sin(theta) + L1*d*ddy_des*lambda2*lambda3*m^3*sin(gamma1)*sin(theta) - L2*d*ddy_des*lambda2*lambda3*m^3*sin(gamma2)*sin(theta) + L1*d*g*lambda2*lambda3*m^3*sin(gamma1)*sin(theta) - L2*d*g*lambda2*lambda3*m^3*sin(gamma2)*sin(theta) - L1*L2*ddy_des*lambda2*lambda3*m^3*mu_s*cos(gamma1)*sin(gamma2) + L1*L2*ddy_des*lambda2*lambda3*m^3*mu_s*cos(gamma2)*sin(gamma1) - L1*L2*g*lambda2*lambda3*m^3*mu_s*cos(gamma1)*sin(gamma2) + L1*L2*g*lambda2*lambda3*m^3*mu_s*cos(gamma2)*sin(gamma1) + L1*L2*ddx_des*lambda1*lambda3*m^3*mu_s*sin(gamma1)*sin(gamma2) - L1*d*ddy_des*lambda2*lambda3*m^3*mu_s*cos(gamma1)*sin(theta) - 3*L1*d*ddy_des*lambda2*lambda3*m^3*mu_s*cos(theta)*sin(gamma1) - L2*d*ddy_des*lambda2*lambda3*m^3*mu_s*cos(gamma2)*sin(theta) + L2*d*ddy_des*lambda2*lambda3*m^3*mu_s*cos(theta)*sin(gamma2) - L1*d*g*lambda2*lambda3*m^3*mu_s*cos(gamma1)*sin(theta) - 3*L1*d*g*lambda2*lambda3*m^3*mu_s*cos(theta)*sin(gamma1) - L2*d*g*lambda2*lambda3*m^3*mu_s*cos(gamma2)*sin(theta) + L2*d*g*lambda2*lambda3*m^3*mu_s*cos(theta)*sin(gamma2) - 3*L1*d*ddx_des*lambda1*lambda3*m^3*mu_s*sin(gamma1)*sin(theta) - L2*d*ddx_des*lambda1*lambda3*m^3*mu_s*sin(gamma2)*sin(theta) - L1*L2*ddx_des*lambda1*lambda3*m^3*mu_s^3*cos(gamma1)*cos(gamma2) - L1*L2*ddy_des*lambda2*lambda3*m^3*mu_s^2*cos(gamma1)*cos(gamma2) - L1*L2*g*lambda2*lambda3*m^3*mu_s^2*cos(gamma1)*cos(gamma2) - L1*L2*ddx_des*lambda1*lambda3*m^3*mu_s^2*cos(gamma1)*sin(gamma2) + L1*L2*ddx_des*lambda1*lambda3*m^3*mu_s^2*cos(gamma2)*sin(gamma1) - L1*d*ddx_des*lambda1*lambda3*m^3*mu_s^3*cos(gamma1)*cos(theta) + L2*d*ddx_des*lambda1*lambda3*m^3*mu_s^3*cos(gamma2)*cos(theta) + 3*L1*d*ddy_des*lambda2*lambda3*m^3*mu_s^2*cos(gamma1)*cos(theta) + L2*d*ddy_des*lambda2*lambda3*m^3*mu_s^2*cos(gamma2)*cos(theta) + 3*L1*d*g*lambda2*lambda3*m^3*mu_s^2*cos(gamma1)*cos(theta) + L2*d*g*lambda2*lambda3*m^3*mu_s^2*cos(gamma2)*cos(theta) + 3*L1*d*ddx_des*lambda1*lambda3*m^3*mu_s^2*cos(gamma1)*sin(theta) + L1*d*ddx_des*lambda1*lambda3*m^3*mu_s^2*cos(theta)*sin(gamma1) - L2*d*ddx_des*lambda1*lambda3*m^3*mu_s^2*cos(gamma2)*sin(theta) + L2*d*ddx_des*lambda1*lambda3*m^3*mu_s^2*cos(theta)*sin(gamma2)))/(4*I^2*lambda1*lambda2*mu_s^2 + L1^2*lambda2*lambda3*m^2*sin(gamma1)^2 + L2^2*lambda2*lambda3*m^2*sin(gamma2)^2 + L1^2*lambda2*lambda3*m^2*mu_s^2*cos(gamma1)^2 + L1^2*lambda1*lambda3*m^2*mu_s^4*cos(gamma1)^2 + L2^2*lambda2*lambda3*m^2*mu_s^2*cos(gamma2)^2 + L2^2*lambda1*lambda3*m^2*mu_s^4*cos(gamma2)^2 + L1^2*lambda1*lambda3*m^2*mu_s^2*sin(gamma1)^2 + L2^2*lambda1*lambda3*m^2*mu_s^2*sin(gamma2)^2 + 4*d^2*lambda2*lambda3*m^2*mu_s^2*cos(theta)^2 + 4*d^2*lambda1*lambda3*m^2*mu_s^2*sin(theta)^2 - 2*L1^2*lambda1*lambda3*m^2*mu_s^3*cos(gamma1)*sin(gamma1) + 2*L2^2*lambda1*lambda3*m^2*mu_s^3*cos(gamma2)*sin(gamma2) - 2*L1*L2*lambda2*lambda3*m^2*sin(gamma1)*sin(gamma2) - 2*L1^2*lambda2*lambda3*m^2*mu_s*cos(gamma1)*sin(gamma1) + 2*L2^2*lambda2*lambda3*m^2*mu_s*cos(gamma2)*sin(gamma2) - 2*L1*L2*lambda1*lambda3*m^2*mu_s^3*cos(gamma1)*sin(gamma2) + 2*L1*L2*lambda1*lambda3*m^2*mu_s^3*cos(gamma2)*sin(gamma1) + 2*L1*L2*lambda1*lambda3*m^2*mu_s^2*sin(gamma1)*sin(gamma2) - 4*L1*d*lambda2*lambda3*m^2*mu_s^2*cos(gamma1)*cos(theta) - 4*L2*d*lambda2*lambda3*m^2*mu_s^2*cos(gamma2)*cos(theta) + 4*L1*d*lambda1*lambda3*m^2*mu_s^3*cos(gamma1)*sin(theta) - 4*L2*d*lambda1*lambda3*m^2*mu_s^3*cos(gamma2)*sin(theta) - 4*L1*d*lambda1*lambda3*m^2*mu_s^2*sin(gamma1)*sin(theta) - 4*L2*d*lambda1*lambda3*m^2*mu_s^2*sin(gamma2)*sin(theta) + 2*L1*L2*lambda2*lambda3*m^2*mu_s*cos(gamma1)*sin(gamma2) - 2*L1*L2*lambda2*lambda3*m^2*mu_s*cos(gamma2)*sin(gamma1) + 4*L1*d*lambda2*lambda3*m^2*mu_s*cos(theta)*sin(gamma1) - 4*L2*d*lambda2*lambda3*m^2*mu_s*cos(theta)*sin(gamma2) + 2*L1*L2*lambda2*lambda3*m^2*mu_s^2*cos(gamma1)*cos(gamma2) - 2*L1*L2*lambda1*lambda3*m^2*mu_s^4*cos(gamma1)*cos(gamma2));
    ]);

f4 = real([                                                                                                                                                                                                                                                                                                                                                                                                                                                                                                                                                                                                                                                                                                                                                                                                                                                                                                                                                                                                                                                                                                                                                                                                                                                                                                                                                                                                                                                                                                                                                                                                                                                                                                                                                                                                                                                                                                                                                                                                                                                                                                                                                                                                                                                                                                                                                                                                                                                                                                                                                                                                                                                                                                                                                                                                                                                                                                                                                                                                                                                                                                                                                                                                                                                                                                                                                                                                                                                                                                                                                                                                                                                                                                                                                                                                                                                                                                                                                                                                                                                                                                                                                                                                                                                                                                                                                                                                                                                                                                                                                                                                                                                                                                                                                                                                                                                                                                                                                                                                                                                                                                                                                                                                                                                                                                                                                                                                                                                                                                                                                                                                                                                         0;
    m*(ddy_des + g);
    0;
    (m*(I^2*ddy_des*lambda1*lambda2 + I^2*g*lambda1*lambda2 + L2^2*ddy_des*lambda2*lambda3*m^2*cos(gamma2)^2 + L2^2*g*lambda2*lambda3*m^2*cos(gamma2)^2 + d^2*ddy_des*lambda2*lambda3*m^2*cos(theta)^2 + d^2*g*lambda2*lambda3*m^2*cos(theta)^2 - I*L2*ddtheta_des*lambda1*lambda3*m*sin(gamma2) + I*d*ddtheta_des*lambda1*lambda3*m*sin(theta) + L2^2*ddx_des*lambda1*lambda3*m^2*cos(gamma2)*sin(gamma2) + d^2*ddx_des*lambda1*lambda3*m^2*cos(theta)*sin(theta) - 2*L2*d*ddy_des*lambda2*lambda3*m^2*cos(gamma2)*cos(theta) - 2*L2*d*g*lambda2*lambda3*m^2*cos(gamma2)*cos(theta) - L2*d*ddx_des*lambda1*lambda3*m^2*cos(gamma2)*sin(theta) - L2*d*ddx_des*lambda1*lambda3*m^2*cos(theta)*sin(gamma2)))/(I^2*lambda1*lambda2 + d^2*lambda1*lambda3*m^2*sin(theta)^2 + L2^2*lambda2*lambda3*m^2*cos(gamma2)^2 + L2^2*lambda1*lambda3*m^2*sin(gamma2)^2 + d^2*lambda2*lambda3*m^2*cos(theta)^2 - 2*L2*d*lambda2*lambda3*m^2*cos(gamma2)*cos(theta) - 2*L2*d*lambda1*lambda3*m^2*sin(gamma2)*sin(theta));
    0;
    0;
    0;
    0;
    0;
    0;
    0;
    (m*(I^2*ddy_des*lambda1*lambda2 + I^2*g*lambda1*lambda2 + L2^2*ddy_des*lambda2*lambda3*m^2*cos(gamma2)^2 + L2^2*g*lambda2*lambda3*m^2*cos(gamma2)^2 + d^2*ddy_des*lambda2*lambda3*m^2*cos(theta)^2 + d^2*g*lambda2*lambda3*m^2*cos(theta)^2 - I*L2*ddtheta_des*lambda1*lambda3*m*sin(gamma2) + I*d*ddtheta_des*lambda1*lambda3*m*sin(theta) + L2^2*ddx_des*lambda1*lambda3*m^2*cos(gamma2)*sin(gamma2) + d^2*ddx_des*lambda1*lambda3*m^2*cos(theta)*sin(theta) - 2*L2*d*ddy_des*lambda2*lambda3*m^2*cos(gamma2)*cos(theta) - 2*L2*d*g*lambda2*lambda3*m^2*cos(gamma2)*cos(theta) - L2*d*ddx_des*lambda1*lambda3*m^2*cos(gamma2)*sin(theta) - L2*d*ddx_des*lambda1*lambda3*m^2*cos(theta)*sin(gamma2)))/(I^2*lambda1*lambda2 + d^2*lambda1*lambda3*m^2*sin(theta)^2 + L2^2*lambda2*lambda3*m^2*cos(gamma2)^2 + L2^2*lambda1*lambda3*m^2*sin(gamma2)^2 + d^2*lambda2*lambda3*m^2*cos(theta)^2 - 2*L2*d*lambda2*lambda3*m^2*cos(gamma2)*cos(theta) - 2*L2*d*lambda1*lambda3*m^2*sin(gamma2)*sin(theta));
    0;
    0;
    0;
    0;
    (I*ddtheta_des - L1*ddx_des*m*cos(gamma1) + L1*ddy_des*m*sin(gamma1) + L1*g*m*sin(gamma1) + d*ddx_des*m*cos(theta) - d*ddy_des*m*sin(theta) - d*g*m*sin(theta))/(L1*sin(gamma1) - L2*sin(gamma2) + L1*mu_s*cos(gamma1) - L2*mu_s*cos(gamma2));
    (I*ddtheta_des - L1*ddx_des*m*cos(gamma1) + L1*ddy_des*m*sin(gamma1) + L1*g*m*sin(gamma1) + d*ddx_des*m*cos(theta) - d*ddy_des*m*sin(theta) - d*g*m*sin(theta))/(L1*sin(gamma1) - L2*sin(gamma2) - L1*mu_s*cos(gamma1) + L2*mu_s*cos(gamma2));
    (I*ddtheta_des - L2*ddx_des*m*cos(gamma2) + L1*ddy_des*m*sin(gamma1) + L1*g*m*sin(gamma1) + d*ddx_des*m*cos(theta) - d*ddy_des*m*sin(theta) - d*g*m*sin(theta) + L1*ddy_des*m*mu_s*cos(gamma1) - L2*ddy_des*m*mu_s*cos(gamma2) + L1*g*m*mu_s*cos(gamma1) - L2*g*m*mu_s*cos(gamma2))/(L1*sin(gamma1) - L2*sin(gamma2) + L1*mu_s*cos(gamma1) - L2*mu_s*cos(gamma2));
    (I*ddtheta_des - L2*ddx_des*m*cos(gamma2) + L1*ddy_des*m*sin(gamma1) + L1*g*m*sin(gamma1) + d*ddx_des*m*cos(theta) - d*ddy_des*m*sin(theta) - d*g*m*sin(theta) - L1*ddy_des*m*mu_s*cos(gamma1) + L2*ddy_des*m*mu_s*cos(gamma2) - L1*g*m*mu_s*cos(gamma1) + L2*g*m*mu_s*cos(gamma2))/(L1*sin(gamma1) - L2*sin(gamma2) - L1*mu_s*cos(gamma1) + L2*mu_s*cos(gamma2));
    0;
    0;
    0;
    0;
    (I*m*(I*ddy_des*lambda2 + I*g*lambda2 + I*ddx_des*lambda1*mu_s - L2*ddtheta_des*lambda3*m*sin(gamma2) + d*ddtheta_des*lambda3*m*sin(theta) + L2*ddtheta_des*lambda3*m*mu_s*cos(gamma2) - d*ddtheta_des*lambda3*m*mu_s*cos(theta)))/(I^2*lambda2 + I^2*lambda1*mu_s^2 + L2^2*lambda3*m^2*sin(gamma2)^2 + d^2*lambda3*m^2*sin(theta)^2 + L2^2*lambda3*m^2*mu_s^2*cos(gamma2)^2 + d^2*lambda3*m^2*mu_s^2*cos(theta)^2 - 2*L2*d*lambda3*m^2*sin(gamma2)*sin(theta) - 2*L2^2*lambda3*m^2*mu_s*cos(gamma2)*sin(gamma2) - 2*d^2*lambda3*m^2*mu_s*cos(theta)*sin(theta) + 2*L2*d*lambda3*m^2*mu_s*cos(gamma2)*sin(theta) + 2*L2*d*lambda3*m^2*mu_s*cos(theta)*sin(gamma2) - 2*L2*d*lambda3*m^2*mu_s^2*cos(gamma2)*cos(theta));
    (I*m*(I*ddy_des*lambda2 + I*g*lambda2 - I*ddx_des*lambda1*mu_s - L2*ddtheta_des*lambda3*m*sin(gamma2) + d*ddtheta_des*lambda3*m*sin(theta) - L2*ddtheta_des*lambda3*m*mu_s*cos(gamma2) + d*ddtheta_des*lambda3*m*mu_s*cos(theta)))/(I^2*lambda2 + I^2*lambda1*mu_s^2 + L2^2*lambda3*m^2*sin(gamma2)^2 + d^2*lambda3*m^2*sin(theta)^2 + L2^2*lambda3*m^2*mu_s^2*cos(gamma2)^2 + d^2*lambda3*m^2*mu_s^2*cos(theta)^2 - 2*L2*d*lambda3*m^2*sin(gamma2)*sin(theta) + 2*L2^2*lambda3*m^2*mu_s*cos(gamma2)*sin(gamma2) + 2*d^2*lambda3*m^2*mu_s*cos(theta)*sin(theta) - 2*L2*d*lambda3*m^2*mu_s*cos(gamma2)*sin(theta) - 2*L2*d*lambda3*m^2*mu_s*cos(theta)*sin(gamma2) - 2*L2*d*lambda3*m^2*mu_s^2*cos(gamma2)*cos(theta));
    0;
    (I*ddtheta_des*lambda2 + I*ddtheta_des*lambda1*mu_s^2 + L1*ddy_des*lambda2*m*sin(gamma1) + L1*g*lambda2*m*sin(gamma1) - d*ddy_des*lambda2*m*sin(theta) - d*g*lambda2*m*sin(theta) + L1*ddy_des*lambda2*m*mu_s*cos(gamma1) + L1*g*lambda2*m*mu_s*cos(gamma1) - L1*ddx_des*lambda1*m*mu_s*sin(gamma1) - d*ddy_des*lambda2*m*mu_s*cos(theta) - d*g*lambda2*m*mu_s*cos(theta) + d*ddx_des*lambda1*m*mu_s*sin(theta) - L1*ddx_des*lambda1*m*mu_s^2*cos(gamma1) + d*ddx_des*lambda1*m*mu_s^2*cos(theta))/((lambda1*mu_s^2 + lambda2)*(L1*sin(gamma1) - L2*sin(gamma2) + L1*mu_s*cos(gamma1) - L2*mu_s*cos(gamma2)));
    (I*ddtheta_des*lambda2 + I*ddtheta_des*lambda1*mu_s^2 + L1*ddy_des*lambda2*m*sin(gamma1) + L1*g*lambda2*m*sin(gamma1) - d*ddy_des*lambda2*m*sin(theta) - d*g*lambda2*m*sin(theta) - L1*ddy_des*lambda2*m*mu_s*cos(gamma1) - L1*g*lambda2*m*mu_s*cos(gamma1) + L1*ddx_des*lambda1*m*mu_s*sin(gamma1) + d*ddy_des*lambda2*m*mu_s*cos(theta) + d*g*lambda2*m*mu_s*cos(theta) - d*ddx_des*lambda1*m*mu_s*sin(theta) - L1*ddx_des*lambda1*m*mu_s^2*cos(gamma1) + d*ddx_des*lambda1*m*mu_s^2*cos(theta))/((lambda1*mu_s^2 + lambda2)*(L1*sin(gamma1) - L2*sin(gamma2) - L1*mu_s*cos(gamma1) + L2*mu_s*cos(gamma2)));
    0;
    (m*(I^2*ddy_des*lambda1*lambda2 + I^2*g*lambda1*lambda2 + L1^2*ddy_des*lambda2*lambda3*m^2*cos(gamma1)^2 + L1^2*g*lambda2*lambda3*m^2*cos(gamma1)^2 + d^2*ddy_des*lambda2*lambda3*m^2*cos(theta)^2 + d^2*g*lambda2*lambda3*m^2*cos(theta)^2 - I*L2*ddtheta_des*lambda1*lambda3*m*sin(gamma2) + I*d*ddtheta_des*lambda1*lambda3*m*sin(theta) + L1^2*ddx_des*lambda1*lambda3*m^2*mu_s*cos(gamma1)^2 + d^2*ddx_des*lambda1*lambda3*m^2*cos(theta)*sin(theta) + L1*L2*ddx_des*lambda1*lambda3*m^2*cos(gamma1)*sin(gamma2) - 2*L1*d*ddy_des*lambda2*lambda3*m^2*cos(gamma1)*cos(theta) - 2*L1*d*g*lambda2*lambda3*m^2*cos(gamma1)*cos(theta) - L1*d*ddx_des*lambda1*lambda3*m^2*cos(gamma1)*sin(theta) - L2*d*ddx_des*lambda1*lambda3*m^2*cos(theta)*sin(gamma2) - I*L1*ddtheta_des*lambda1*lambda3*m*mu_s*cos(gamma1) + I*L2*ddtheta_des*lambda1*lambda3*m*mu_s*cos(gamma2) - L1*L2*ddx_des*lambda1*lambda3*m^2*mu_s*cos(gamma1)*cos(gamma2) - L1*d*ddx_des*lambda1*lambda3*m^2*mu_s*cos(gamma1)*cos(theta) + L2*d*ddx_des*lambda1*lambda3*m^2*mu_s*cos(gamma2)*cos(theta)))/(I^2*lambda1*lambda2 + d^2*lambda1*lambda3*m^2*sin(theta)^2 + L1^2*lambda2*lambda3*m^2*cos(gamma1)^2 + L2^2*lambda1*lambda3*m^2*sin(gamma2)^2 + d^2*lambda2*lambda3*m^2*cos(theta)^2 + L1^2*lambda1*lambda3*m^2*mu_s^2*cos(gamma1)^2 + L2^2*lambda1*lambda3*m^2*mu_s^2*cos(gamma2)^2 - 2*L1*d*lambda2*lambda3*m^2*cos(gamma1)*cos(theta) - 2*L2*d*lambda1*lambda3*m^2*sin(gamma2)*sin(theta) - 2*L2^2*lambda1*lambda3*m^2*mu_s*cos(gamma2)*sin(gamma2) + 2*L1*L2*lambda1*lambda3*m^2*mu_s*cos(gamma1)*sin(gamma2) - 2*L1*d*lambda1*lambda3*m^2*mu_s*cos(gamma1)*sin(theta) + 2*L2*d*lambda1*lambda3*m^2*mu_s*cos(gamma2)*sin(theta) - 2*L1*L2*lambda1*lambda3*m^2*mu_s^2*cos(gamma1)*cos(gamma2));
    (m*(I^2*ddy_des*lambda1*lambda2 + I^2*g*lambda1*lambda2 + L1^2*ddy_des*lambda2*lambda3*m^2*cos(gamma1)^2 + L1^2*g*lambda2*lambda3*m^2*cos(gamma1)^2 + d^2*ddy_des*lambda2*lambda3*m^2*cos(theta)^2 + d^2*g*lambda2*lambda3*m^2*cos(theta)^2 - I*L2*ddtheta_des*lambda1*lambda3*m*sin(gamma2) + I*d*ddtheta_des*lambda1*lambda3*m*sin(theta) - L1^2*ddx_des*lambda1*lambda3*m^2*mu_s*cos(gamma1)^2 + d^2*ddx_des*lambda1*lambda3*m^2*cos(theta)*sin(theta) + L1*L2*ddx_des*lambda1*lambda3*m^2*cos(gamma1)*sin(gamma2) - 2*L1*d*ddy_des*lambda2*lambda3*m^2*cos(gamma1)*cos(theta) - 2*L1*d*g*lambda2*lambda3*m^2*cos(gamma1)*cos(theta) - L1*d*ddx_des*lambda1*lambda3*m^2*cos(gamma1)*sin(theta) - L2*d*ddx_des*lambda1*lambda3*m^2*cos(theta)*sin(gamma2) + I*L1*ddtheta_des*lambda1*lambda3*m*mu_s*cos(gamma1) - I*L2*ddtheta_des*lambda1*lambda3*m*mu_s*cos(gamma2) + L1*L2*ddx_des*lambda1*lambda3*m^2*mu_s*cos(gamma1)*cos(gamma2) + L1*d*ddx_des*lambda1*lambda3*m^2*mu_s*cos(gamma1)*cos(theta) - L2*d*ddx_des*lambda1*lambda3*m^2*mu_s*cos(gamma2)*cos(theta)))/(I^2*lambda1*lambda2 + d^2*lambda1*lambda3*m^2*sin(theta)^2 + L1^2*lambda2*lambda3*m^2*cos(gamma1)^2 + L2^2*lambda1*lambda3*m^2*sin(gamma2)^2 + d^2*lambda2*lambda3*m^2*cos(theta)^2 + L1^2*lambda1*lambda3*m^2*mu_s^2*cos(gamma1)^2 + L2^2*lambda1*lambda3*m^2*mu_s^2*cos(gamma2)^2 - 2*L1*d*lambda2*lambda3*m^2*cos(gamma1)*cos(theta) - 2*L2*d*lambda1*lambda3*m^2*sin(gamma2)*sin(theta) + 2*L2^2*lambda1*lambda3*m^2*mu_s*cos(gamma2)*sin(gamma2) - 2*L1*L2*lambda1*lambda3*m^2*mu_s*cos(gamma1)*sin(gamma2) + 2*L1*d*lambda1*lambda3*m^2*mu_s*cos(gamma1)*sin(theta) - 2*L2*d*lambda1*lambda3*m^2*mu_s*cos(gamma2)*sin(theta) - 2*L1*L2*lambda1*lambda3*m^2*mu_s^2*cos(gamma1)*cos(gamma2));
    0;
    0;
    0;
    (m*(I^2*ddy_des*lambda1*lambda2 + I^2*g*lambda1*lambda2 + L2^2*ddy_des*lambda2*lambda3*m^2*cos(gamma2)^2 + L2^2*g*lambda2*lambda3*m^2*cos(gamma2)^2 + d^2*ddy_des*lambda2*lambda3*m^2*cos(theta)^2 + d^2*g*lambda2*lambda3*m^2*cos(theta)^2 - I*L2*ddtheta_des*lambda1*lambda3*m*sin(gamma2) + I*d*ddtheta_des*lambda1*lambda3*m*sin(theta) + L2^2*ddx_des*lambda1*lambda3*m^2*cos(gamma2)*sin(gamma2) + d^2*ddx_des*lambda1*lambda3*m^2*cos(theta)*sin(theta) - 2*L2*d*ddy_des*lambda2*lambda3*m^2*cos(gamma2)*cos(theta) - 2*L2*d*g*lambda2*lambda3*m^2*cos(gamma2)*cos(theta) - L2*d*ddx_des*lambda1*lambda3*m^2*cos(gamma2)*sin(theta) - L2*d*ddx_des*lambda1*lambda3*m^2*cos(theta)*sin(gamma2)))/(I^2*lambda1*lambda2 + d^2*lambda1*lambda3*m^2*sin(theta)^2 + L2^2*lambda2*lambda3*m^2*cos(gamma2)^2 + L2^2*lambda1*lambda3*m^2*sin(gamma2)^2 + d^2*lambda2*lambda3*m^2*cos(theta)^2 - 2*L2*d*lambda2*lambda3*m^2*cos(gamma2)*cos(theta) - 2*L2*d*lambda1*lambda3*m^2*sin(gamma2)*sin(theta));
    (m*(I^2*ddy_des*lambda1*lambda2 + I^2*g*lambda1*lambda2 + L2^2*ddy_des*lambda2*lambda3*m^2*cos(gamma2)^2 + L2^2*g*lambda2*lambda3*m^2*cos(gamma2)^2 + d^2*ddy_des*lambda2*lambda3*m^2*cos(theta)^2 + d^2*g*lambda2*lambda3*m^2*cos(theta)^2 - I*L2*ddtheta_des*lambda1*lambda3*m*sin(gamma2) + I*d*ddtheta_des*lambda1*lambda3*m*sin(theta) + L2^2*ddx_des*lambda1*lambda3*m^2*cos(gamma2)*sin(gamma2) + d^2*ddx_des*lambda1*lambda3*m^2*cos(theta)*sin(theta) - 2*L2*d*ddy_des*lambda2*lambda3*m^2*cos(gamma2)*cos(theta) - 2*L2*d*g*lambda2*lambda3*m^2*cos(gamma2)*cos(theta) - L2*d*ddx_des*lambda1*lambda3*m^2*cos(gamma2)*sin(theta) - L2*d*ddx_des*lambda1*lambda3*m^2*cos(theta)*sin(gamma2)))/(I^2*lambda1*lambda2 + d^2*lambda1*lambda3*m^2*sin(theta)^2 + L2^2*lambda2*lambda3*m^2*cos(gamma2)^2 + L2^2*lambda1*lambda3*m^2*sin(gamma2)^2 + d^2*lambda2*lambda3*m^2*cos(theta)^2 - 2*L2*d*lambda2*lambda3*m^2*cos(gamma2)*cos(theta) - 2*L2*d*lambda1*lambda3*m^2*sin(gamma2)*sin(theta));
    0;
    0;
    0;
    0;
    0;
    0;
    0;
    0;
    0;
    0;
    0;
    0;
    0;
    (I*m*(I*ddy_des*lambda2 + I*g*lambda2 + I*ddx_des*lambda1*mu_s - L2*ddtheta_des*lambda3*m*sin(gamma2) + d*ddtheta_des*lambda3*m*sin(theta) + L2*ddtheta_des*lambda3*m*mu_s*cos(gamma2) - d*ddtheta_des*lambda3*m*mu_s*cos(theta)))/(I^2*lambda2 + I^2*lambda1*mu_s^2 + L2^2*lambda3*m^2*sin(gamma2)^2 + d^2*lambda3*m^2*sin(theta)^2 + L2^2*lambda3*m^2*mu_s^2*cos(gamma2)^2 + d^2*lambda3*m^2*mu_s^2*cos(theta)^2 - 2*L2*d*lambda3*m^2*sin(gamma2)*sin(theta) - 2*L2^2*lambda3*m^2*mu_s*cos(gamma2)*sin(gamma2) - 2*d^2*lambda3*m^2*mu_s*cos(theta)*sin(theta) + 2*L2*d*lambda3*m^2*mu_s*cos(gamma2)*sin(theta) + 2*L2*d*lambda3*m^2*mu_s*cos(theta)*sin(gamma2) - 2*L2*d*lambda3*m^2*mu_s^2*cos(gamma2)*cos(theta));
    (I*m*(I*ddy_des*lambda2 + I*g*lambda2 - I*ddx_des*lambda1*mu_s - L2*ddtheta_des*lambda3*m*sin(gamma2) + d*ddtheta_des*lambda3*m*sin(theta) - L2*ddtheta_des*lambda3*m*mu_s*cos(gamma2) + d*ddtheta_des*lambda3*m*mu_s*cos(theta)))/(I^2*lambda2 + I^2*lambda1*mu_s^2 + L2^2*lambda3*m^2*sin(gamma2)^2 + d^2*lambda3*m^2*sin(theta)^2 + L2^2*lambda3*m^2*mu_s^2*cos(gamma2)^2 + d^2*lambda3*m^2*mu_s^2*cos(theta)^2 - 2*L2*d*lambda3*m^2*sin(gamma2)*sin(theta) + 2*L2^2*lambda3*m^2*mu_s*cos(gamma2)*sin(gamma2) + 2*d^2*lambda3*m^2*mu_s*cos(theta)*sin(theta) - 2*L2*d*lambda3*m^2*mu_s*cos(gamma2)*sin(theta) - 2*L2*d*lambda3*m^2*mu_s*cos(theta)*sin(gamma2) - 2*L2*d*lambda3*m^2*mu_s^2*cos(gamma2)*cos(theta));
    0;
    0;
    0;
    0;
    (I*m*(I*ddy_des*lambda2 + I*g*lambda2 - I*ddx_des*lambda1*mu_s - L2*ddtheta_des*lambda3*m*sin(gamma2) + d*ddtheta_des*lambda3*m*sin(theta) - L2*ddtheta_des*lambda3*m*mu_s*cos(gamma2) + d*ddtheta_des*lambda3*m*mu_s*cos(theta)))/(I^2*lambda2 + I^2*lambda1*mu_s^2 + L2^2*lambda3*m^2*sin(gamma2)^2 + d^2*lambda3*m^2*sin(theta)^2 + L2^2*lambda3*m^2*mu_s^2*cos(gamma2)^2 + d^2*lambda3*m^2*mu_s^2*cos(theta)^2 - 2*L2*d*lambda3*m^2*sin(gamma2)*sin(theta) + 2*L2^2*lambda3*m^2*mu_s*cos(gamma2)*sin(gamma2) + 2*d^2*lambda3*m^2*mu_s*cos(theta)*sin(theta) - 2*L2*d*lambda3*m^2*mu_s*cos(gamma2)*sin(theta) - 2*L2*d*lambda3*m^2*mu_s*cos(theta)*sin(gamma2) - 2*L2*d*lambda3*m^2*mu_s^2*cos(gamma2)*cos(theta));
    (I*m*(I*ddy_des*lambda2 + I*g*lambda2 + I*ddx_des*lambda1*mu_s - L2*ddtheta_des*lambda3*m*sin(gamma2) + d*ddtheta_des*lambda3*m*sin(theta) + L2*ddtheta_des*lambda3*m*mu_s*cos(gamma2) - d*ddtheta_des*lambda3*m*mu_s*cos(theta)))/(I^2*lambda2 + I^2*lambda1*mu_s^2 + L2^2*lambda3*m^2*sin(gamma2)^2 + d^2*lambda3*m^2*sin(theta)^2 + L2^2*lambda3*m^2*mu_s^2*cos(gamma2)^2 + d^2*lambda3*m^2*mu_s^2*cos(theta)^2 - 2*L2*d*lambda3*m^2*sin(gamma2)*sin(theta) - 2*L2^2*lambda3*m^2*mu_s*cos(gamma2)*sin(gamma2) - 2*d^2*lambda3*m^2*mu_s*cos(theta)*sin(theta) + 2*L2*d*lambda3*m^2*mu_s*cos(gamma2)*sin(theta) + 2*L2*d*lambda3*m^2*mu_s*cos(theta)*sin(gamma2) - 2*L2*d*lambda3*m^2*mu_s^2*cos(gamma2)*cos(theta));
    0;
    0;
    (I*m*(I*ddy_des*lambda2 + I*g*lambda2 + I*ddx_des*lambda1*mu_s - L2*ddtheta_des*lambda3*m*sin(gamma2) + d*ddtheta_des*lambda3*m*sin(theta) + L2*ddtheta_des*lambda3*m*mu_s*cos(gamma2) - d*ddtheta_des*lambda3*m*mu_s*cos(theta)))/(I^2*lambda2 + I^2*lambda1*mu_s^2 + L2^2*lambda3*m^2*sin(gamma2)^2 + d^2*lambda3*m^2*sin(theta)^2 + L2^2*lambda3*m^2*mu_s^2*cos(gamma2)^2 + d^2*lambda3*m^2*mu_s^2*cos(theta)^2 - 2*L2*d*lambda3*m^2*sin(gamma2)*sin(theta) - 2*L2^2*lambda3*m^2*mu_s*cos(gamma2)*sin(gamma2) - 2*d^2*lambda3*m^2*mu_s*cos(theta)*sin(theta) + 2*L2*d*lambda3*m^2*mu_s*cos(gamma2)*sin(theta) + 2*L2*d*lambda3*m^2*mu_s*cos(theta)*sin(gamma2) - 2*L2*d*lambda3*m^2*mu_s^2*cos(gamma2)*cos(theta));
    (I*m*(I*ddy_des*lambda2 + I*g*lambda2 - I*ddx_des*lambda1*mu_s - L2*ddtheta_des*lambda3*m*sin(gamma2) + d*ddtheta_des*lambda3*m*sin(theta) - L2*ddtheta_des*lambda3*m*mu_s*cos(gamma2) + d*ddtheta_des*lambda3*m*mu_s*cos(theta)))/(I^2*lambda2 + I^2*lambda1*mu_s^2 + L2^2*lambda3*m^2*sin(gamma2)^2 + d^2*lambda3*m^2*sin(theta)^2 + L2^2*lambda3*m^2*mu_s^2*cos(gamma2)^2 + d^2*lambda3*m^2*mu_s^2*cos(theta)^2 - 2*L2*d*lambda3*m^2*sin(gamma2)*sin(theta) + 2*L2^2*lambda3*m^2*mu_s*cos(gamma2)*sin(gamma2) + 2*d^2*lambda3*m^2*mu_s*cos(theta)*sin(theta) - 2*L2*d*lambda3*m^2*mu_s*cos(gamma2)*sin(theta) - 2*L2*d*lambda3*m^2*mu_s*cos(theta)*sin(gamma2) - 2*L2*d*lambda3*m^2*mu_s^2*cos(gamma2)*cos(theta));
